simulink model "ABB_1010"  (R2024a)
(part 15 of 16)

et89 = Iyy6*dQ1*dQ5*t2*t4*t7*t35*t36*4.0+Iyy6*dQ1*dQ6*t4*t5*t9*t32*t33*4.0+Iyy6*dQ1*dQ2*t4*t5*t10*t33*t36*4.0+Iyy6*dQ1*dQ3*t4*t5*t10*t32*t36*4.0+Iyy6*dQ1*dQ3*t4*t5*t10*t33*t36*4.0+Iyy6*dQ1*dQ4*t5*t6*t11*t32*t33*4.0+Iyy6*dQ1*dQ5*t3*t4*t8*t35*t36*4.0+Iyy6*dQ2*dQ5*t2*t3*t9*t35*t36*2.0+Iyy6*dQ1*dQ4*t5*t6*t11*t32*t34*4.0+Iyy6*dQ1*dQ6*t4*t5*t9*t32*t36*4.0+Iyy6*dQ2*dQ6*t2*t5*t8*t34*t36*4.0+Iyy6*dQ2*dQ6*t3*t5*t7*t34*t36*4.0+Iyy6*dQ3*dQ5*t2*t3*t9*t35*t36*2.0+Iyy6*dQ1*dQ4*t5*t6*t11*t33*t34*4.0+Iyy6*dQ1*dQ6*t4*t5*t9*t33*t36*4.0+Iyy6*dQ3*dQ6*t2*t5*t8*t34*t36*4.0+Iyy6*dQ3*dQ6*t3*t5*t7*t34*t36*4.0-Iyy6*dQ4*dQ5*t2*t4*t8*t35*t36*2.0-Iyy6*dQ4*dQ5*t3*t4*t7*t35*t36*2.0;
et90 = Iyy6*dQ2*dQ5*t7*t8*t9*t35*t36*-2.0-Iyy6*dQ3*dQ5*t7*t8*t9*t35*t36*2.0+Iyy6*dQ1*dQ2*t2*t7*t33*t34*t35*4.0-Iyy6*dQ1*dQ2*t2*t7*t33*t34*t36*4.0+Iyy6*dQ1*dQ2*t3*t8*t32*t34*t35*4.0+Iyy6*dQ1*dQ3*t2*t7*t33*t34*t35*4.0-Iyy6*dQ1*dQ2*t2*t7*t33*t35*t36*4.0-Iyy6*dQ1*dQ2*t3*t8*t32*t34*t36*4.0-Iyy6*dQ1*dQ3*t2*t7*t33*t34*t36*4.0+Iyy6*dQ1*dQ3*t3*t8*t32*t34*t35*4.0+Iyy6*dQ1*dQ2*t2*t7*t34*t35*t36*2.0-Iyy6*dQ1*dQ2*t3*t8*t32*t35*t36*4.0-Iyy6*dQ1*dQ3*t2*t7*t33*t35*t36*4.0-Iyy6*dQ1*dQ3*t3*t8*t32*t34*t36*4.0+Iyy6*dQ1*dQ3*t2*t7*t34*t35*t36*2.0-Iyy6*dQ1*dQ3*t3*t8*t32*t35*t36*4.0+Iyy6*dQ1*dQ4*t4*t9*t32*t33*t35*4.0+Iyy6*dQ1*dQ2*t3*t8*t34*t35*t36*2.0;
et91 = Iyy6*dQ1*dQ4*t4*t9*t32*t33*t36*-4.0+Iyy6*dQ1*dQ3*t3*t8*t34*t35*t36*2.0+Iyy6*dQ1*dQ5*t5*t10*t32*t33*t34*4.0+Iyy6*dQ1*dQ4*t4*t9*t32*t35*t36*2.0+Iyy6*dQ2*dQ4*t2*t8*t34*t35*t36*2.0+Iyy6*dQ2*dQ4*t3*t7*t34*t35*t36*2.0+Iyy6*dQ1*dQ4*t4*t9*t33*t35*t36*2.0-Iyy6*dQ1*dQ5*t5*t10*t32*t33*t36*4.0+Iyy6*dQ3*dQ4*t2*t8*t34*t35*t36*2.0+Iyy6*dQ3*dQ4*t3*t7*t34*t35*t36*2.0+Iyy6*dQ1*dQ5*t5*t10*t32*t34*t36*2.0-Iyy6*dQ1*dQ6*t6*t11*t32*t33*t34*4.0+Iyy6*dQ1*dQ5*t5*t10*t33*t34*t36*2.0-Iyy6*dQ1*dQ6*t6*t11*t32*t33*t35*4.0+Iyy6*dQ1*dQ6*t6*t11*t32*t34*t35*2.0+Iyy6*dQ1*dQ6*t6*t11*t33*t34*t35*2.0-Izz5*dQ1*dQ4*t2*t5*t7*t9*t10*2.0-Izz5*dQ2*dQ3*t2*t5*t8*t9*t10*2.0-Izz5*dQ2*dQ3*t3*t5*t7*t9*t10*2.0;
et92 = Izz6*dQ1*dQ4*t2*t5*t7*t9*t10*-2.0-Izz5*dQ1*dQ4*t3*t5*t8*t9*t10*2.0-Izz6*dQ2*dQ3*t2*t5*t8*t9*t10*2.0-Izz6*dQ2*dQ3*t3*t5*t7*t9*t10*2.0-Izz6*dQ1*dQ4*t3*t5*t8*t9*t10*2.0+Izz5*dQ2*dQ3*t2*t3*t4*t9*t35*2.0+Izz6*dQ2*dQ3*t2*t3*t4*t9*t35*2.0-Izz5*dQ2*dQ3*t4*t7*t8*t9*t35*2.0-Izz6*dQ2*dQ3*t4*t7*t8*t9*t35*2.0-Izz5*dQ1*dQ2*t4*t5*t10*t32*t33*8.0-Izz5*dQ1*dQ5*t2*t4*t7*t33*t35*8.0-Izz5*dQ1*dQ3*t4*t5*t10*t32*t33*8.0-Izz5*dQ1*dQ5*t3*t4*t8*t32*t35*8.0-Izz6*dQ1*dQ2*t4*t5*t10*t32*t33*8.0-Izz6*dQ1*dQ5*t2*t4*t7*t33*t35*8.0-Izz6*dQ1*dQ3*t4*t5*t10*t32*t33*8.0-Izz6*dQ1*dQ5*t3*t4*t8*t32*t35*8.0;
et93 = Izz5*dQ1*dQ2*t2*t7*t33*t34*t35*-4.0-Izz5*dQ1*dQ2*t3*t8*t32*t34*t35*4.0-Izz5*dQ1*dQ3*t2*t7*t33*t34*t35*4.0-Izz6*dQ1*dQ2*t2*t7*t33*t34*t35*4.0-Izz5*dQ1*dQ3*t3*t8*t32*t34*t35*4.0-Izz6*dQ1*dQ2*t3*t8*t32*t34*t35*4.0-Izz6*dQ1*dQ3*t2*t7*t33*t34*t35*4.0-Izz6*dQ1*dQ3*t3*t8*t32*t34*t35*4.0-Izz5*dQ1*dQ4*t4*t9*t32*t33*t35*4.0-Izz6*dQ1*dQ4*t4*t9*t32*t33*t35*4.0-Izz5*dQ1*dQ5*t5*t10*t32*t33*t34*4.0-Izz6*dQ1*dQ5*t5*t10*t32*t33*t34*4.0+dQ2*dQ3*m4*t2*t3*t4*t9*t14*2.0+dQ2*dQ3*m5*t2*t3*t4*t9*t14*2.0+dQ2*dQ3*m4*t2*t3*t4*t9*t16*2.0+dQ2*dQ3*m6*t2*t3*t4*t9*t14*2.0-dQ2*dQ3*m4*t2*t3*t4*t9*t19*2.0-dQ2*dQ3*m6*t2*t3*t4*t9*t18*2.0;
et94 = dQ2*dQ3*m5*t2*t3*t4*t9*t20*-2.0-dQ2*dQ3*m4*t4*t7*t8*t9*t14*2.0+dQ2*dQ3*m6*t2*t3*t4*t9*t22*2.0-dQ2*dQ6*m6*t2*t3*t4*t10*t18*2.0-dQ4*dQ5*m5*t2*t3*t5*t10*t17*2.0-dQ2*dQ3*m5*t4*t7*t8*t9*t14*2.0-dQ3*dQ6*m6*t2*t3*t4*t10*t18*2.0-dQ2*dQ3*m4*t4*t7*t8*t9*t16*2.0+dQ2*dQ3*m5*t2*t3*t4*t9*t25*2.0-dQ2*dQ3*m6*t4*t7*t8*t9*t14*2.0-dQ5*dQ6*m6*t2*t4*t5*t8*t18*2.0-dQ5*dQ6*m6*t3*t4*t5*t7*t18*2.0+dQ2*dQ3*m6*t2*t3*t4*t9*t26*2.0+dQ2*dQ3*m4*t4*t7*t8*t9*t19*2.0-dQ4*dQ5*m6*t2*t3*t5*t10*t21*2.0+dQ4*dQ6*m6*t2*t3*t6*t11*t18*2.0+dQ2*dQ3*m6*t4*t7*t8*t9*t18*2.0+dQ4*dQ5*m6*t2*t3*t5*t10*t22*2.0;
et95 = dQ2*dQ3*m5*t4*t7*t8*t9*t20*2.0+dQ1*dQ6*m6*t2*t7*t9*t10*t18*2.0+dQ4*dQ5*m5*t2*t3*t5*t10*t25*2.0-dQ4*dQ6*m6*t2*t3*t6*t11*t21*2.0+dQ1*dQ6*m6*t3*t8*t9*t10*t18*2.0-dQ2*dQ3*m6*t4*t7*t8*t9*t22*2.0+dQ2*dQ6*m6*t4*t7*t8*t10*t18*2.0+dQ4*dQ5*m5*t5*t7*t8*t10*t17*2.0+dQ4*dQ5*m6*t2*t3*t5*t10*t26*2.0-dQ1*dQ6*m6*t2*t7*t9*t10*t21*2.0+dQ3*dQ6*m6*t4*t7*t8*t10*t18*2.0+dQ1*dQ2*m6*t6*t9*t10*t11*t18*2.0-dQ2*dQ3*m5*t4*t7*t8*t9*t25*2.0+dQ1*dQ3*m6*t6*t9*t10*t11*t18*2.0-dQ1*dQ6*m6*t3*t8*t9*t10*t21*2.0-dQ2*dQ3*m6*t4*t7*t8*t9*t26*2.0-dQ1*dQ2*m6*t6*t9*t10*t11*t21*2.0+dQ4*dQ5*m6*t5*t7*t8*t10*t21*2.0+dQ4*dQ6*m6*t2*t8*t9*t10*t21*2.0;
et96 = dQ4*dQ6*m6*t3*t7*t9*t10*t21*2.0-dQ4*dQ6*m6*t6*t7*t8*t11*t18*2.0-dQ1*dQ3*m6*t6*t9*t10*t11*t21*2.0-dQ4*dQ5*m6*t5*t7*t8*t10*t22*2.0-dQ4*dQ5*m5*t5*t7*t8*t10*t25*2.0+dQ4*dQ6*m6*t6*t7*t8*t11*t21*2.0-dQ4*dQ5*m6*t5*t7*t8*t10*t26*2.0+dQ1*dQ5*m5*t2*t4*t7*t17*t33*4.0+dQ1*dQ5*m5*t3*t4*t8*t17*t32*4.0+dQ1*dQ2*m5*t4*t5*t10*t17*t32*4.0+dQ1*dQ5*m5*t2*t4*t7*t17*t35*4.0+dQ1*dQ2*m5*t4*t5*t10*t17*t33*4.0+dQ1*dQ3*m5*t4*t5*t10*t17*t32*4.0+dQ1*dQ3*m5*t4*t5*t10*t17*t33*4.0+dQ1*dQ5*m5*t3*t4*t8*t17*t35*4.0+dQ2*dQ5*m5*t2*t3*t9*t17*t35*2.0-dQ1*dQ5*m6*t2*t4*t7*t18*t36*2.0+dQ1*dQ5*m6*t2*t4*t7*t21*t33*4.0+dQ3*dQ5*m5*t2*t3*t9*t17*t35*2.0;
et97 = dQ1*dQ5*m6*t2*t4*t7*t22*t33*-4.0+dQ1*dQ5*m6*t3*t4*t8*t21*t32*4.0-dQ4*dQ5*m5*t2*t4*t8*t17*t35*2.0-dQ4*dQ5*m5*t3*t4*t7*t17*t35*2.0+dQ1*dQ2*m6*t4*t5*t10*t21*t32*4.0+dQ1*dQ5*m6*t2*t4*t7*t21*t35*4.0-dQ1*dQ5*m6*t3*t4*t8*t18*t36*2.0-dQ1*dQ5*m6*t3*t4*t8*t22*t32*4.0-dQ1*dQ6*m6*t4*t5*t9*t18*t32*2.0-dQ2*dQ6*m6*t2*t5*t8*t18*t34*2.0-dQ2*dQ6*m6*t3*t5*t7*t18*t34*2.0-dQ1*dQ2*m6*t4*t5*t10*t18*t36*2.0+dQ1*dQ2*m6*t4*t5*t10*t21*t33*4.0-dQ1*dQ2*m6*t4*t5*t10*t22*t32*4.0+dQ1*dQ3*m6*t4*t5*t10*t21*t32*4.0-dQ1*dQ5*m5*t2*t4*t7*t25*t33*4.0+dQ1*dQ5*m6*t2*t4*t7*t21*t36*2.0-dQ1*dQ5*m6*t2*t4*t7*t22*t35*4.0;
et98 = dQ1*dQ6*m6*t4*t5*t9*t18*t33*-2.0-dQ3*dQ6*m6*t2*t5*t8*t18*t34*2.0-dQ3*dQ6*m6*t3*t5*t7*t18*t34*2.0-dQ1*dQ2*m6*t4*t5*t10*t22*t33*4.0-dQ1*dQ3*m6*t4*t5*t10*t18*t36*2.0+dQ1*dQ3*m6*t4*t5*t10*t21*t33*4.0-dQ1*dQ3*m6*t4*t5*t10*t22*t32*4.0-dQ1*dQ4*m6*t5*t6*t11*t18*t32*2.0-dQ1*dQ5*m5*t3*t4*t8*t25*t32*4.0+dQ1*dQ5*m6*t3*t4*t8*t21*t35*4.0+dQ2*dQ5*m6*t2*t3*t9*t21*t35*2.0-dQ2*dQ6*m6*t2*t5*t8*t18*t36*2.0-dQ2*dQ6*m6*t3*t5*t7*t18*t36*2.0+dQ4*dQ5*m6*t2*t4*t8*t18*t36*2.0+dQ4*dQ5*m6*t3*t4*t7*t18*t36*2.0-dQ1*dQ2*m5*t4*t5*t10*t25*t32*4.0-dQ1*dQ3*m6*t4*t5*t10*t22*t33*4.0-dQ1*dQ4*m6*t5*t6*t11*t18*t33*2.0;
et99 = dQ1*dQ5*m5*t2*t4*t7*t25*t35*-4.0-dQ1*dQ5*m6*t2*t4*t7*t26*t33*4.0+dQ1*dQ5*m6*t3*t4*t8*t21*t36*2.0-dQ1*dQ5*m6*t3*t4*t8*t22*t35*4.0+dQ1*dQ6*m6*t4*t5*t9*t21*t32*2.0-dQ2*dQ5*m6*t2*t3*t9*t22*t35*2.0+dQ2*dQ6*m6*t2*t5*t8*t21*t34*2.0+dQ2*dQ6*m6*t3*t5*t7*t21*t34*2.0+dQ3*dQ5*m6*t2*t3*t9*t21*t35*2.0-dQ3*dQ6*m6*t2*t5*t8*t18*t36*2.0-dQ3*dQ6*m6*t3*t5*t7*t18*t36*2.0-dQ1*dQ2*m5*t4*t5*t10*t25*t33*4.0+dQ1*dQ2*m6*t4*t5*t10*t21*t36*2.0-dQ1*dQ3*m5*t4*t5*t10*t25*t32*4.0-dQ1*dQ5*m6*t3*t4*t8*t26*t32*4.0+dQ1*dQ6*m6*t4*t5*t9*t21*t33*2.0-dQ3*dQ5*m6*t2*t3*t9*t22*t35*2.0+dQ3*dQ6*m6*t2*t5*t8*t21*t34*2.0+dQ3*dQ6*m6*t3*t5*t7*t21*t34*2.0;
et100 = dQ4*dQ5*m6*t2*t4*t8*t21*t35*-2.0-dQ4*dQ5*m6*t3*t4*t7*t21*t35*2.0-dQ1*dQ2*m6*t4*t5*t10*t26*t32*4.0-dQ1*dQ3*m5*t4*t5*t10*t25*t33*4.0+dQ1*dQ3*m6*t4*t5*t10*t21*t36*2.0+dQ1*dQ4*m6*t5*t6*t11*t21*t32*2.0-dQ1*dQ5*m5*t3*t4*t8*t25*t35*4.0-dQ1*dQ5*m6*t2*t4*t7*t26*t35*4.0-dQ2*dQ5*m5*t2*t3*t9*t25*t35*2.0+dQ2*dQ6*m6*t2*t5*t8*t21*t36*2.0+dQ2*dQ6*m6*t3*t5*t7*t21*t36*2.0-dQ4*dQ5*m6*t2*t4*t8*t21*t36*2.0+dQ4*dQ5*m6*t2*t4*t8*t22*t35*2.0-dQ4*dQ5*m6*t3*t4*t7*t21*t36*2.0+dQ4*dQ5*m6*t3*t4*t7*t22*t35*2.0+dQ5*dQ6*m6*t2*t3*t10*t18*t36*2.0-dQ1*dQ2*m6*t4*t5*t10*t26*t33*4.0-dQ1*dQ3*m6*t4*t5*t10*t26*t32*4.0;
et101 = dQ1*dQ4*m6*t5*t6*t11*t21*t33*2.0-dQ3*dQ5*m5*t2*t3*t9*t25*t35*2.0+dQ3*dQ6*m6*t2*t5*t8*t21*t36*2.0+dQ3*dQ6*m6*t3*t5*t7*t21*t36*2.0-dQ1*dQ3*m6*t4*t5*t10*t26*t33*4.0-dQ1*dQ5*m6*t3*t4*t8*t26*t35*4.0-dQ2*dQ5*m5*t7*t8*t9*t17*t35*2.0-dQ2*dQ5*m6*t2*t3*t9*t26*t35*2.0+dQ4*dQ5*m5*t2*t4*t8*t25*t35*2.0+dQ4*dQ5*m5*t3*t4*t7*t25*t35*2.0-dQ3*dQ5*m5*t7*t8*t9*t17*t35*2.0-dQ3*dQ5*m6*t2*t3*t9*t26*t35*2.0-dQ5*dQ6*m6*t2*t3*t10*t21*t36*2.0+dQ4*dQ5*m6*t2*t4*t8*t26*t35*2.0+dQ4*dQ5*m6*t3*t4*t7*t26*t35*2.0-dQ2*dQ5*m6*t7*t8*t9*t21*t35*2.0+dQ2*dQ5*m6*t7*t8*t9*t22*t35*2.0-dQ3*dQ5*m6*t7*t8*t9*t21*t35*2.0+dQ3*dQ5*m6*t7*t8*t9*t22*t35*2.0;
et102 = dQ2*dQ5*m5*t7*t8*t9*t25*t35*2.0-dQ5*dQ6*m6*t7*t8*t10*t18*t36*2.0-dQ1*dQ2*m4*t2*t7*t14*t33*t34*4.0+dQ3*dQ5*m5*t7*t8*t9*t25*t35*2.0-dQ1*dQ2*m4*t3*t8*t14*t32*t34*4.0-dQ1*dQ2*m5*t2*t7*t14*t33*t34*4.0-dQ1*dQ3*m4*t2*t7*t14*t33*t34*4.0+dQ2*dQ5*m6*t7*t8*t9*t26*t35*2.0-dQ1*dQ2*m4*t2*t7*t16*t33*t34*4.0-dQ1*dQ2*m5*t3*t8*t14*t32*t34*4.0-dQ1*dQ2*m6*t2*t7*t14*t33*t34*4.0-dQ1*dQ3*m4*t3*t8*t14*t32*t34*4.0-dQ1*dQ3*m5*t2*t7*t14*t33*t34*4.0+dQ3*dQ5*m6*t7*t8*t9*t26*t35*2.0+dQ5*dQ6*m6*t7*t8*t10*t21*t36*2.0-dQ1*dQ2*m4*t3*t8*t16*t32*t34*4.0-dQ1*dQ2*m6*t3*t8*t14*t32*t34*4.0-dQ1*dQ3*m4*t2*t7*t16*t33*t34*4.0;
et103 = dQ1*dQ3*m5*t3*t8*t14*t32*t34*-4.0-dQ1*dQ3*m6*t2*t7*t14*t33*t34*4.0-dQ1*dQ3*m4*t3*t8*t16*t32*t34*4.0-dQ1*dQ3*m6*t3*t8*t14*t32*t34*4.0-dQ1*dQ4*m4*t4*t9*t14*t32*t33*4.0+dQ1*dQ2*m4*t2*t7*t19*t33*t34*4.0-dQ1*dQ2*m5*t2*t7*t17*t33*t35*4.0-dQ1*dQ4*m5*t4*t9*t14*t32*t33*4.0+dQ1*dQ2*m4*t3*t8*t19*t32*t34*4.0+dQ1*dQ2*m5*t2*t7*t17*t34*t35*2.0-dQ1*dQ2*m5*t3*t8*t17*t32*t35*4.0+dQ1*dQ2*m6*t2*t7*t18*t33*t34*4.0+dQ1*dQ3*m4*t2*t7*t19*t33*t34*4.0-dQ1*dQ3*m5*t2*t7*t17*t33*t35*4.0-dQ1*dQ4*m4*t4*t9*t16*t32*t33*4.0-dQ1*dQ4*m6*t4*t9*t14*t32*t33*4.0+dQ1*dQ2*m5*t2*t7*t20*t33*t34*4.0+dQ1*dQ2*m6*t3*t8*t18*t32*t34*4.0;
et104 = dQ1*dQ3*m4*t3*t8*t19*t32*t34*4.0+dQ1*dQ3*m5*t2*t7*t17*t34*t35*2.0-dQ1*dQ3*m5*t3*t8*t17*t32*t35*4.0+dQ1*dQ3*m6*t2*t7*t18*t33*t34*4.0+dQ1*dQ2*m5*t3*t8*t17*t34*t35*2.0+dQ1*dQ2*m5*t3*t8*t20*t32*t34*4.0+dQ1*dQ2*m6*t2*t7*t18*t33*t36*8.0+dQ1*dQ3*m5*t2*t7*t20*t33*t34*4.0+dQ1*dQ3*m6*t3*t8*t18*t32*t34*4.0+dQ1*dQ2*m6*t2*t7*t18*t34*t36*2.0+dQ1*dQ2*m6*t3*t8*t18*t32*t36*8.0+dQ1*dQ3*m5*t3*t8*t17*t34*t35*2.0+dQ1*dQ3*m5*t3*t8*t20*t32*t34*4.0+dQ1*dQ3*m6*t2*t7*t18*t33*t36*8.0+dQ1*dQ4*m4*t4*t9*t19*t32*t33*4.0+dQ1*dQ2*m6*t2*t7*t18*t35*t36*2.0-dQ1*dQ2*m6*t2*t7*t21*t33*t35*4.0-dQ1*dQ2*m6*t2*t7*t22*t33*t34*4.0+dQ1*dQ3*m6*t2*t7*t18*t34*t36*2.0;
et105 = dQ1*dQ3*m6*t3*t8*t18*t32*t36*8.0+dQ1*dQ4*m5*t4*t9*t17*t32*t35*2.0+dQ1*dQ4*m6*t4*t9*t18*t32*t33*4.0+dQ2*dQ4*m5*t2*t8*t17*t34*t35*2.0+dQ2*dQ4*m5*t3*t7*t17*t34*t35*2.0-dQ1*dQ2*m6*t2*t7*t21*t33*t36*8.0+dQ1*dQ2*m6*t2*t7*t21*t34*t35*2.0+dQ1*dQ2*m6*t2*t7*t22*t33*t35*4.0+dQ1*dQ2*m6*t3*t8*t18*t34*t36*2.0-dQ1*dQ2*m6*t3*t8*t21*t32*t35*4.0-dQ1*dQ2*m6*t3*t8*t22*t32*t34*4.0+dQ1*dQ3*m6*t2*t7*t18*t35*t36*2.0-dQ1*dQ3*m6*t2*t7*t21*t33*t35*4.0-dQ1*dQ3*m6*t2*t7*t22*t33*t34*4.0+dQ1*dQ4*m5*t4*t9*t17*t33*t35*2.0+dQ1*dQ4*m5*t4*t9*t20*t32*t33*4.0-dQ1*dQ5*m5*t5*t10*t17*t32*t33*4.0+dQ3*dQ4*m5*t2*t8*t17*t34*t35*2.0+dQ3*dQ4*m5*t3*t7*t17*t34*t35*2.0;
et106 = dQ1*dQ2*m5*t2*t7*t25*t33*t34*-4.0-dQ1*dQ2*m6*t2*t7*t21*t34*t36*2.0-dQ1*dQ2*m6*t2*t7*t22*t34*t35*2.0+dQ1*dQ2*m6*t3*t8*t18*t35*t36*2.0-dQ1*dQ2*m6*t3*t8*t21*t32*t36*8.0+dQ1*dQ2*m6*t3*t8*t22*t32*t35*4.0-dQ1*dQ3*m6*t2*t7*t21*t33*t36*8.0+dQ1*dQ3*m6*t2*t7*t21*t34*t35*2.0+dQ1*dQ3*m6*t2*t7*t22*t33*t35*4.0+dQ1*dQ3*m6*t3*t8*t18*t34*t36*2.0-dQ1*dQ3*m6*t3*t8*t21*t32*t35*4.0-dQ1*dQ3*m6*t3*t8*t22*t32*t34*4.0+dQ1*dQ5*m5*t5*t10*t17*t32*t34*2.0+dQ1*dQ2*m5*t2*t7*t25*t33*t35*4.0-dQ1*dQ2*m5*t3*t8*t25*t32*t34*4.0-dQ1*dQ2*m6*t2*t7*t21*t35*t36*2.0+dQ1*dQ2*m6*t3*t8*t21*t34*t35*2.0-dQ1*dQ3*m5*t2*t7*t25*t33*t34*4.0;
et107 = dQ1*dQ3*m6*t2*t7*t21*t34*t36*-2.0-dQ1*dQ3*m6*t2*t7*t22*t34*t35*2.0+dQ1*dQ3*m6*t3*t8*t18*t35*t36*2.0-dQ1*dQ3*m6*t3*t8*t21*t32*t36*8.0+dQ1*dQ3*m6*t3*t8*t22*t32*t35*4.0+dQ1*dQ4*m6*t4*t9*t18*t32*t36*2.0+dQ1*dQ5*m5*t5*t10*t17*t33*t34*2.0+dQ2*dQ4*m6*t2*t8*t18*t34*t36*2.0+dQ2*dQ4*m6*t3*t7*t18*t34*t36*2.0-dQ1*dQ2*m5*t2*t7*t25*t34*t35*2.0+dQ1*dQ2*m5*t3*t8*t25*t32*t35*4.0-dQ1*dQ2*m6*t2*t7*t26*t33*t34*4.0-dQ1*dQ2*m6*t3*t8*t21*t34*t36*2.0-dQ1*dQ2*m6*t3*t8*t22*t34*t35*2.0+dQ1*dQ3*m5*t2*t7*t25*t33*t35*4.0-dQ1*dQ3*m5*t3*t8*t25*t32*t34*4.0-dQ1*dQ3*m6*t2*t7*t21*t35*t36*2.0+dQ1*dQ3*m6*t3*t8*t21*t34*t35*2.0+dQ1*dQ4*m6*t4*t9*t18*t33*t36*2.0;
et108 = dQ1*dQ4*m6*t4*t9*t22*t32*t33*-4.0-dQ2*dQ4*m6*t2*t8*t18*t35*t36*2.0-dQ2*dQ4*m6*t3*t7*t18*t35*t36*2.0+dQ3*dQ4*m6*t2*t8*t18*t34*t36*2.0+dQ3*dQ4*m6*t3*t7*t18*t34*t36*2.0+dQ1*dQ2*m6*t2*t7*t26*t33*t35*4.0-dQ1*dQ2*m6*t3*t8*t21*t35*t36*2.0-dQ1*dQ2*m6*t3*t8*t26*t32*t34*4.0-dQ1*dQ3*m5*t2*t7*t25*t34*t35*2.0+dQ1*dQ3*m5*t3*t8*t25*t32*t35*4.0-dQ1*dQ3*m6*t2*t7*t26*t33*t34*4.0-dQ1*dQ3*m6*t3*t8*t21*t34*t36*2.0-dQ1*dQ3*m6*t3*t8*t22*t34*t35*2.0+dQ1*dQ4*m6*t4*t9*t21*t32*t35*2.0+dQ2*dQ4*m6*t2*t8*t21*t34*t35*2.0+dQ2*dQ4*m6*t3*t7*t21*t34*t35*2.0-dQ3*dQ4*m6*t2*t8*t18*t35*t36*2.0-dQ3*dQ4*m6*t3*t7*t18*t35*t36*2.0;
et109 = dQ1*dQ2*m5*t3*t8*t25*t34*t35*-2.0-dQ1*dQ2*m6*t2*t7*t26*t34*t35*2.0+dQ1*dQ2*m6*t3*t8*t26*t32*t35*4.0+dQ1*dQ3*m6*t2*t7*t26*t33*t35*4.0-dQ1*dQ3*m6*t3*t8*t21*t35*t36*2.0-dQ1*dQ3*m6*t3*t8*t26*t32*t34*4.0-dQ1*dQ4*m5*t4*t9*t25*t32*t33*4.0-dQ1*dQ4*m6*t4*t9*t21*t32*t36*2.0+dQ1*dQ4*m6*t4*t9*t21*t33*t35*2.0-dQ1*dQ4*m6*t4*t9*t22*t32*t35*2.0+dQ1*dQ5*m6*t5*t10*t18*t32*t36*2.0-dQ1*dQ5*m6*t5*t10*t21*t32*t33*4.0+dQ1*dQ6*m6*t6*t11*t18*t32*t33*8.0-dQ2*dQ4*m6*t2*t8*t21*t34*t36*2.0-dQ2*dQ4*m6*t2*t8*t22*t34*t35*2.0-dQ2*dQ4*m6*t3*t7*t21*t34*t36*2.0-dQ2*dQ4*m6*t3*t7*t22*t34*t35*2.0+dQ3*dQ4*m6*t2*t8*t21*t34*t35*2.0;
et110 = dQ3*dQ4*m6*t3*t7*t21*t34*t35*2.0-dQ1*dQ3*m5*t3*t8*t25*t34*t35*2.0-dQ1*dQ3*m6*t2*t7*t26*t34*t35*2.0+dQ1*dQ3*m6*t3*t8*t26*t32*t35*4.0-dQ1*dQ4*m6*t4*t9*t21*t33*t36*2.0-dQ1*dQ4*m6*t4*t9*t22*t33*t35*2.0+dQ1*dQ5*m6*t5*t10*t18*t33*t36*2.0+dQ1*dQ5*m6*t5*t10*t21*t32*t34*2.0+dQ1*dQ5*m6*t5*t10*t22*t32*t33*4.0+dQ1*dQ6*m6*t6*t11*t18*t32*t34*2.0+dQ2*dQ4*m6*t2*t8*t21*t35*t36*2.0+dQ2*dQ4*m6*t3*t7*t21*t35*t36*2.0-dQ3*dQ4*m6*t2*t8*t21*t34*t36*2.0-dQ3*dQ4*m6*t2*t8*t22*t34*t35*2.0-dQ3*dQ4*m6*t3*t7*t21*t34*t36*2.0-dQ3*dQ4*m6*t3*t7*t22*t34*t35*2.0-dQ1*dQ2*m6*t3*t8*t26*t34*t35*2.0-dQ1*dQ4*m5*t4*t9*t25*t32*t35*2.0;
et111 = dQ1*dQ4*m6*t4*t9*t26*t32*t33*-4.0+dQ1*dQ5*m6*t5*t10*t21*t33*t34*2.0-dQ1*dQ5*m6*t5*t10*t22*t32*t34*2.0+dQ1*dQ6*m6*t6*t11*t18*t32*t35*2.0+dQ1*dQ6*m6*t6*t11*t18*t33*t34*2.0-dQ2*dQ4*m5*t2*t8*t25*t34*t35*2.0-dQ2*dQ4*m5*t3*t7*t25*t34*t35*2.0+dQ3*dQ4*m6*t2*t8*t21*t35*t36*2.0+dQ3*dQ4*m6*t3*t7*t21*t35*t36*2.0-dQ1*dQ3*m6*t3*t8*t26*t34*t35*2.0-dQ1*dQ4*m5*t4*t9*t25*t33*t35*2.0+dQ1*dQ5*m5*t5*t10*t25*t32*t33*4.0-dQ1*dQ5*m6*t5*t10*t21*t32*t36*2.0-dQ1*dQ5*m6*t5*t10*t22*t33*t34*2.0+dQ1*dQ6*m6*t6*t11*t18*t33*t35*2.0-dQ1*dQ6*m6*t6*t11*t21*t32*t33*8.0-dQ3*dQ4*m5*t2*t8*t25*t34*t35*2.0-dQ3*dQ4*m5*t3*t7*t25*t34*t35*2.0;
et112 = dQ1*dQ4*m6*t4*t9*t26*t32*t35*-2.0-dQ1*dQ5*m5*t5*t10*t25*t32*t34*2.0-dQ1*dQ5*m6*t5*t10*t21*t33*t36*2.0-dQ1*dQ6*m6*t6*t11*t21*t32*t34*2.0-dQ2*dQ4*m6*t2*t8*t26*t34*t35*2.0-dQ2*dQ4*m6*t3*t7*t26*t34*t35*2.0-dQ1*dQ4*m6*t4*t9*t26*t33*t35*2.0-dQ1*dQ5*m5*t5*t10*t25*t33*t34*2.0+dQ1*dQ5*m6*t5*t10*t26*t32*t33*4.0-dQ1*dQ6*m6*t6*t11*t21*t32*t35*2.0-dQ1*dQ6*m6*t6*t11*t21*t33*t34*2.0-dQ3*dQ4*m6*t2*t8*t26*t34*t35*2.0-dQ3*dQ4*m6*t3*t7*t26*t34*t35*2.0-dQ1*dQ5*m6*t5*t10*t26*t32*t34*2.0-dQ1*dQ6*m6*t6*t11*t21*t33*t35*2.0-dQ1*dQ5*m6*t5*t10*t26*t33*t34*2.0-Ixx6*dQ2*dQ5*t2*t3*t4*t5*t6*t11*2.0-Ixx6*dQ3*dQ5*t2*t3*t4*t5*t6*t11*2.0;
et113 = Ixx5*dQ1*dQ5*t2*t3*t5*t7*t8*t10*-4.0+Ixx5*dQ2*dQ5*t2*t4*t5*t8*t9*t10*2.0+Ixx5*dQ2*dQ5*t3*t4*t5*t7*t9*t10*2.0+Ixx6*dQ1*dQ6*t2*t3*t6*t7*t8*t11*8.0+Ixx5*dQ3*dQ5*t2*t4*t5*t8*t9*t10*2.0+Ixx5*dQ3*dQ5*t3*t4*t5*t7*t9*t10*2.0+Ixx6*dQ1*dQ4*t2*t4*t6*t7*t10*t11*2.0+Ixx6*dQ1*dQ5*t2*t5*t6*t7*t9*t11*2.0+Ixx6*dQ2*dQ3*t2*t4*t6*t8*t10*t11*2.0+Ixx6*dQ2*dQ3*t3*t4*t6*t7*t10*t11*2.0+Ixx6*dQ1*dQ4*t3*t4*t6*t8*t10*t11*2.0+Ixx6*dQ1*dQ5*t3*t5*t6*t8*t9*t11*2.0+Ixx6*dQ2*dQ5*t4*t5*t6*t7*t8*t11*2.0+Ixx6*dQ2*dQ6*t2*t4*t6*t8*t9*t11*2.0+Ixx6*dQ2*dQ6*t3*t4*t6*t7*t9*t11*2.0+Ixx6*dQ3*dQ5*t4*t5*t6*t7*t8*t11*2.0+Ixx6*dQ3*dQ6*t2*t4*t6*t8*t9*t11*2.0+Ixx6*dQ3*dQ6*t3*t4*t6*t7*t9*t11*2.0;
et114 = Ixx6*dQ2*dQ3*t2*t3*t5*t6*t11*t34*-4.0-Ixx5*dQ1*dQ4*t2*t5*t7*t9*t10*t33*4.0-Ixx5*dQ1*dQ4*t3*t5*t8*t9*t10*t32*4.0+Ixx6*dQ1*dQ4*t2*t5*t7*t9*t10*t36*2.0+Ixx6*dQ2*dQ3*t2*t5*t8*t9*t10*t36*2.0+Ixx6*dQ2*dQ3*t3*t5*t7*t9*t10*t36*2.0+Ixx6*dQ1*dQ4*t3*t5*t8*t9*t10*t36*2.0+Ixx6*dQ2*dQ3*t5*t6*t7*t8*t11*t34*4.0+Ixx6*dQ1*dQ5*t4*t6*t9*t10*t11*t32*2.0+Ixx6*dQ2*dQ5*t2*t6*t8*t10*t11*t34*2.0+Ixx6*dQ2*dQ5*t3*t6*t7*t10*t11*t34*2.0+Ixx6*dQ1*dQ5*t4*t6*t9*t10*t11*t33*2.0+Ixx6*dQ3*dQ5*t2*t6*t8*t10*t11*t34*2.0+Ixx6*dQ3*dQ5*t3*t6*t7*t10*t11*t34*2.0-Ixx6*dQ2*dQ3*t2*t3*t4*t9*t35*t36*2.0-Ixx6*dQ1*dQ2*t6*t9*t10*t11*t32*t33*8.0-Ixx6*dQ1*dQ6*t2*t7*t9*t10*t33*t36*8.0;
et115 = Ixx6*dQ2*dQ3*t4*t7*t8*t9*t35*t36*2.0-Ixx6*dQ1*dQ3*t6*t9*t10*t11*t32*t33*8.0-Ixx6*dQ1*dQ6*t3*t8*t9*t10*t32*t36*8.0+Ixx6*dQ1*dQ2*t4*t5*t10*t32*t33*t36*8.0+Ixx6*dQ1*dQ5*t2*t4*t7*t33*t35*t36*8.0+Ixx6*dQ1*dQ3*t4*t5*t10*t32*t33*t36*8.0+Ixx6*dQ1*dQ5*t3*t4*t8*t32*t35*t36*8.0+Ixx6*dQ1*dQ4*t5*t6*t11*t32*t33*t34*8.0+Ixx6*dQ1*dQ6*t4*t5*t9*t32*t33*t36*8.0+Ixx6*dQ1*dQ2*t2*t7*t33*t34*t35*t36*4.0+Ixx6*dQ1*dQ2*t3*t8*t32*t34*t35*t36*4.0+Ixx6*dQ1*dQ3*t2*t7*t33*t34*t35*t36*4.0+Ixx6*dQ1*dQ3*t3*t8*t32*t34*t35*t36*4.0+Ixx6*dQ1*dQ4*t4*t9*t32*t33*t35*t36*4.0+Ixx6*dQ1*dQ5*t5*t10*t32*t33*t34*t36*4.0+Ixx6*dQ1*dQ6*t6*t11*t32*t33*t34*t35*4.0+Iyy6*dQ2*dQ5*t2*t3*t4*t5*t6*t11*2.0;
et116 = Iyy6*dQ3*dQ5*t2*t3*t4*t5*t6*t11*2.0-Iyy6*dQ1*dQ5*t2*t3*t5*t7*t8*t10*4.0-Iyy6*dQ1*dQ6*t2*t3*t6*t7*t8*t11*8.0-Iyy6*dQ1*dQ4*t2*t4*t6*t7*t10*t11*2.0+Iyy6*dQ2*dQ5*t2*t4*t5*t8*t9*t10*2.0+Iyy6*dQ2*dQ5*t3*t4*t5*t7*t9*t10*2.0-Iyy6*dQ1*dQ5*t2*t5*t6*t7*t9*t11*2.0-Iyy6*dQ2*dQ3*t2*t4*t6*t8*t10*t11*2.0-Iyy6*dQ2*dQ3*t3*t4*t6*t7*t10*t11*2.0+Iyy6*dQ3*dQ5*t2*t4*t5*t8*t9*t10*2.0+Iyy6*dQ3*dQ5*t3*t4*t5*t7*t9*t10*2.0-Iyy6*dQ1*dQ4*t3*t4*t6*t8*t10*t11*2.0-Iyy6*dQ1*dQ5*t3*t5*t6*t8*t9*t11*2.0-Iyy6*dQ2*dQ5*t4*t5*t6*t7*t8*t11*2.0-Iyy6*dQ2*dQ6*t2*t4*t6*t8*t9*t11*2.0-Iyy6*dQ2*dQ6*t3*t4*t6*t7*t9*t11*2.0-Iyy6*dQ3*dQ5*t4*t5*t6*t7*t8*t11*2.0;
et117 = Iyy6*dQ3*dQ6*t2*t4*t6*t8*t9*t11*-2.0-Iyy6*dQ3*dQ6*t3*t4*t6*t7*t9*t11*2.0+Iyy6*dQ2*dQ3*t2*t3*t5*t6*t11*t34*4.0-Iyy6*dQ1*dQ4*t2*t5*t7*t9*t10*t33*4.0-Iyy6*dQ1*dQ4*t3*t5*t8*t9*t10*t32*4.0-Iyy6*dQ1*dQ4*t2*t5*t7*t9*t10*t36*2.0-Iyy6*dQ2*dQ3*t2*t5*t8*t9*t10*t36*2.0-Iyy6*dQ2*dQ3*t3*t5*t7*t9*t10*t36*2.0-Iyy6*dQ1*dQ4*t3*t5*t8*t9*t10*t36*2.0-Iyy6*dQ2*dQ3*t5*t6*t7*t8*t11*t34*4.0-Iyy6*dQ1*dQ5*t4*t6*t9*t10*t11*t32*2.0-Iyy6*dQ2*dQ5*t2*t6*t8*t10*t11*t34*2.0-Iyy6*dQ2*dQ5*t3*t6*t7*t10*t11*t34*2.0-Iyy6*dQ1*dQ5*t4*t6*t9*t10*t11*t33*2.0-Iyy6*dQ3*dQ5*t2*t6*t8*t10*t11*t34*2.0-Iyy6*dQ3*dQ5*t3*t6*t7*t10*t11*t34*2.0;
et118 = Iyy6*dQ2*dQ3*t2*t3*t4*t9*t35*t36*2.0+Iyy6*dQ1*dQ2*t6*t9*t10*t11*t32*t33*8.0+Iyy6*dQ1*dQ6*t2*t7*t9*t10*t33*t36*8.0-Iyy6*dQ2*dQ3*t4*t7*t8*t9*t35*t36*2.0+Iyy6*dQ1*dQ3*t6*t9*t10*t11*t32*t33*8.0+Iyy6*dQ1*dQ6*t3*t8*t9*t10*t32*t36*8.0-Iyy6*dQ1*dQ2*t4*t5*t10*t32*t33*t36*8.0-Iyy6*dQ1*dQ5*t2*t4*t7*t33*t35*t36*8.0-Iyy6*dQ1*dQ3*t4*t5*t10*t32*t33*t36*8.0-Iyy6*dQ1*dQ5*t3*t4*t8*t32*t35*t36*8.0-Iyy6*dQ1*dQ4*t5*t6*t11*t32*t33*t34*8.0-Iyy6*dQ1*dQ6*t4*t5*t9*t32*t33*t36*8.0-Iyy6*dQ1*dQ2*t2*t7*t33*t34*t35*t36*4.0-Iyy6*dQ1*dQ2*t3*t8*t32*t34*t35*t36*4.0-Iyy6*dQ1*dQ3*t2*t7*t33*t34*t35*t36*4.0-Iyy6*dQ1*dQ3*t3*t8*t32*t34*t35*t36*4.0;
et119 = Iyy6*dQ1*dQ4*t4*t9*t32*t33*t35*t36*-4.0-Iyy6*dQ1*dQ5*t5*t10*t32*t33*t34*t36*4.0-Iyy6*dQ1*dQ6*t6*t11*t32*t33*t34*t35*4.0+Izz5*dQ1*dQ5*t2*t3*t5*t7*t8*t10*4.0+Izz6*dQ1*dQ5*t2*t3*t5*t7*t8*t10*4.0-Izz5*dQ2*dQ5*t2*t4*t5*t8*t9*t10*2.0-Izz5*dQ2*dQ5*t3*t4*t5*t7*t9*t10*2.0-Izz5*dQ3*dQ5*t2*t4*t5*t8*t9*t10*2.0-Izz5*dQ3*dQ5*t3*t4*t5*t7*t9*t10*2.0-Izz6*dQ2*dQ5*t2*t4*t5*t8*t9*t10*2.0-Izz6*dQ2*dQ5*t3*t4*t5*t7*t9*t10*2.0-Izz6*dQ3*dQ5*t2*t4*t5*t8*t9*t10*2.0-Izz6*dQ3*dQ5*t3*t4*t5*t7*t9*t10*2.0+Izz5*dQ1*dQ4*t2*t5*t7*t9*t10*t33*4.0+Izz5*dQ1*dQ4*t3*t5*t8*t9*t10*t32*4.0+Izz6*dQ1*dQ4*t2*t5*t7*t9*t10*t33*4.0+Izz6*dQ1*dQ4*t3*t5*t8*t9*t10*t32*4.0;
et120 = dQ2*dQ3*m6*t2*t3*t5*t6*t11*t18*-2.0+dQ2*dQ3*m6*t2*t3*t5*t6*t11*t21*2.0-dQ1*dQ4*m5*t2*t5*t7*t9*t10*t17*2.0-dQ2*dQ3*m5*t2*t5*t8*t9*t10*t17*2.0-dQ2*dQ3*m5*t3*t5*t7*t9*t10*t17*2.0-dQ1*dQ4*m5*t3*t5*t8*t9*t10*t17*2.0-dQ1*dQ4*m6*t2*t5*t7*t9*t10*t21*2.0+dQ1*dQ4*m6*t2*t5*t7*t9*t10*t22*2.0-dQ2*dQ3*m6*t2*t5*t8*t9*t10*t21*2.0-dQ2*dQ3*m6*t3*t5*t7*t9*t10*t21*2.0+dQ2*dQ3*m6*t5*t6*t7*t8*t11*t18*2.0-dQ1*dQ4*m6*t3*t5*t8*t9*t10*t21*2.0+dQ2*dQ3*m6*t2*t5*t8*t9*t10*t22*2.0+dQ2*dQ3*m6*t3*t5*t7*t9*t10*t22*2.0+dQ1*dQ4*m5*t2*t5*t7*t9*t10*t25*2.0+dQ1*dQ4*m6*t3*t5*t8*t9*t10*t22*2.0+dQ2*dQ3*m5*t2*t5*t8*t9*t10*t25*2.0;
et121 = dQ2*dQ3*m5*t3*t5*t7*t9*t10*t25*2.0-dQ2*dQ3*m6*t5*t6*t7*t8*t11*t21*2.0+dQ1*dQ4*m5*t3*t5*t8*t9*t10*t25*2.0+dQ1*dQ4*m6*t2*t5*t7*t9*t10*t26*2.0+dQ2*dQ3*m6*t2*t5*t8*t9*t10*t26*2.0+dQ2*dQ3*m6*t3*t5*t7*t9*t10*t26*2.0-dQ5*dQ6*m6*t2*t6*t8*t9*t11*t18*2.0-dQ5*dQ6*m6*t3*t6*t7*t9*t11*t18*2.0+dQ1*dQ4*m6*t3*t5*t8*t9*t10*t26*2.0+dQ5*dQ6*m6*t2*t6*t8*t9*t11*t21*2.0+dQ5*dQ6*m6*t3*t6*t7*t9*t11*t21*2.0+dQ2*dQ3*m5*t2*t3*t4*t9*t17*t35*2.0+dQ2*dQ3*m6*t2*t3*t4*t9*t18*t36*2.0+dQ2*dQ3*m6*t2*t3*t4*t9*t21*t35*2.0-dQ2*dQ3*m6*t2*t3*t4*t9*t21*t36*2.0-dQ2*dQ3*m6*t2*t3*t4*t9*t22*t35*2.0+dQ2*dQ6*m6*t2*t3*t4*t10*t18*t36*2.0;
et122 = dQ2*dQ3*m5*t2*t3*t4*t9*t25*t35*-2.0+dQ3*dQ6*m6*t2*t3*t4*t10*t18*t36*2.0-dQ4*dQ5*m6*t2*t3*t5*t10*t18*t36*2.0-dQ2*dQ3*m5*t4*t7*t8*t9*t17*t35*2.0-dQ2*dQ3*m6*t2*t3*t4*t9*t26*t35*2.0-dQ2*dQ6*m6*t2*t3*t4*t10*t21*t36*2.0+dQ5*dQ6*m6*t2*t4*t5*t8*t18*t36*2.0+dQ5*dQ6*m6*t3*t4*t5*t7*t18*t36*2.0-dQ3*dQ6*m6*t2*t3*t4*t10*t21*t36*2.0-dQ4*dQ6*m6*t2*t3*t6*t11*t18*t35*2.0-dQ1*dQ6*m6*t2*t7*t9*t10*t18*t33*4.0+dQ4*dQ5*m6*t2*t3*t5*t10*t21*t36*2.0-dQ1*dQ6*m6*t3*t8*t9*t10*t18*t32*4.0-dQ2*dQ3*m6*t4*t7*t8*t9*t18*t36*2.0-dQ5*dQ6*m6*t2*t4*t5*t8*t21*t36*2.0-dQ5*dQ6*m6*t3*t4*t5*t7*t21*t36*2.0+dQ4*dQ6*m6*t2*t3*t6*t11*t21*t35*2.0;
et123 = dQ1*dQ2*m6*t6*t9*t10*t11*t18*t32*-4.0-dQ1*dQ6*m6*t2*t7*t9*t10*t18*t36*4.0+dQ1*dQ6*m6*t2*t7*t9*t10*t21*t33*4.0-dQ2*dQ3*m6*t4*t7*t8*t9*t21*t35*2.0-dQ1*dQ2*m6*t6*t9*t10*t11*t18*t33*4.0-dQ1*dQ3*m6*t6*t9*t10*t11*t18*t32*4.0+dQ1*dQ6*m6*t3*t8*t9*t10*t21*t32*4.0+dQ2*dQ3*m6*t4*t7*t8*t9*t21*t36*2.0+dQ2*dQ3*m6*t4*t7*t8*t9*t22*t35*2.0-dQ1*dQ3*m6*t6*t9*t10*t11*t18*t33*4.0-dQ1*dQ6*m6*t3*t8*t9*t10*t18*t36*4.0-dQ2*dQ6*m6*t4*t7*t8*t10*t18*t36*2.0+dQ1*dQ2*m6*t6*t9*t10*t11*t21*t32*4.0+dQ1*dQ6*m6*t2*t7*t9*t10*t21*t36*4.0+dQ2*dQ3*m5*t4*t7*t8*t9*t25*t35*2.0-dQ3*dQ6*m6*t4*t7*t8*t10*t18*t36*2.0+dQ1*dQ2*m6*t6*t9*t10*t11*t21*t33*4.0;
et124 = dQ1*dQ3*m6*t6*t9*t10*t11*t21*t32*4.0+dQ4*dQ5*m6*t5*t7*t8*t10*t18*t36*2.0+dQ4*dQ6*m6*t2*t8*t9*t10*t18*t36*2.0+dQ4*dQ6*m6*t3*t7*t9*t10*t18*t36*2.0+dQ1*dQ3*m6*t6*t9*t10*t11*t21*t33*4.0+dQ1*dQ6*m6*t3*t8*t9*t10*t21*t36*4.0+dQ2*dQ3*m6*t4*t7*t8*t9*t26*t35*2.0+dQ2*dQ6*m6*t4*t7*t8*t10*t21*t36*2.0+dQ3*dQ6*m6*t4*t7*t8*t10*t21*t36*2.0+dQ4*dQ6*m6*t6*t7*t8*t11*t18*t35*2.0-dQ4*dQ5*m6*t5*t7*t8*t10*t21*t36*2.0-dQ4*dQ6*m6*t2*t8*t9*t10*t21*t36*2.0-dQ4*dQ6*m6*t3*t7*t9*t10*t21*t36*2.0-dQ4*dQ6*m6*t6*t7*t8*t11*t21*t35*2.0-dQ1*dQ2*m5*t4*t5*t10*t17*t32*t33*8.0-dQ1*dQ5*m5*t2*t4*t7*t17*t33*t35*8.0-dQ1*dQ3*m5*t4*t5*t10*t17*t32*t33*8.0;
et125 = dQ1*dQ5*m5*t3*t4*t8*t17*t32*t35*-8.0+dQ1*dQ5*m6*t2*t4*t7*t18*t33*t36*4.0+dQ1*dQ5*m6*t3*t4*t8*t18*t32*t36*4.0+dQ1*dQ2*m6*t4*t5*t10*t18*t32*t36*4.0-dQ1*dQ2*m6*t4*t5*t10*t21*t32*t33*8.0+dQ1*dQ5*m6*t2*t4*t7*t18*t35*t36*4.0-dQ1*dQ5*m6*t2*t4*t7*t21*t33*t35*8.0+dQ1*dQ6*m6*t4*t5*t9*t18*t32*t33*4.0+dQ1*dQ2*m6*t4*t5*t10*t18*t33*t36*4.0+dQ1*dQ2*m6*t4*t5*t10*t22*t32*t33*8.0+dQ1*dQ3*m6*t4*t5*t10*t18*t32*t36*4.0-dQ1*dQ3*m6*t4*t5*t10*t21*t32*t33*8.0-dQ1*dQ5*m6*t2*t4*t7*t21*t33*t36*4.0+dQ1*dQ5*m6*t2*t4*t7*t22*t33*t35*8.0-dQ1*dQ5*m6*t3*t4*t8*t21*t32*t35*8.0+dQ1*dQ3*m6*t4*t5*t10*t18*t33*t36*4.0;
et126 = dQ1*dQ3*m6*t4*t5*t10*t22*t32*t33*8.0+dQ1*dQ4*m6*t5*t6*t11*t18*t32*t33*4.0+dQ1*dQ5*m6*t3*t4*t8*t18*t35*t36*4.0-dQ1*dQ5*m6*t3*t4*t8*t21*t32*t36*4.0+dQ1*dQ5*m6*t3*t4*t8*t22*t32*t35*8.0+dQ2*dQ5*m6*t2*t3*t9*t18*t35*t36*2.0+dQ1*dQ2*m5*t4*t5*t10*t25*t32*t33*8.0-dQ1*dQ2*m6*t4*t5*t10*t21*t32*t36*4.0+dQ1*dQ4*m6*t5*t6*t11*t18*t32*t34*4.0+dQ1*dQ5*m5*t2*t4*t7*t25*t33*t35*8.0-dQ1*dQ5*m6*t2*t4*t7*t21*t35*t36*4.0+dQ1*dQ6*m6*t4*t5*t9*t18*t32*t36*4.0-dQ1*dQ6*m6*t4*t5*t9*t21*t32*t33*4.0+dQ2*dQ6*m6*t2*t5*t8*t18*t34*t36*4.0+dQ2*dQ6*m6*t3*t5*t7*t18*t34*t36*4.0+dQ3*dQ5*m6*t2*t3*t9*t18*t35*t36*2.0-dQ1*dQ2*m6*t4*t5*t10*t21*t33*t36*4.0;
et127 = dQ1*dQ3*m5*t4*t5*t10*t25*t32*t33*8.0-dQ1*dQ3*m6*t4*t5*t10*t21*t32*t36*4.0+dQ1*dQ4*m6*t5*t6*t11*t18*t33*t34*4.0+dQ1*dQ5*m5*t3*t4*t8*t25*t32*t35*8.0+dQ1*dQ6*m6*t4*t5*t9*t18*t33*t36*4.0+dQ3*dQ6*m6*t2*t5*t8*t18*t34*t36*4.0+dQ3*dQ6*m6*t3*t5*t7*t18*t34*t36*4.0-dQ4*dQ5*m6*t2*t4*t8*t18*t35*t36*2.0-dQ4*dQ5*m6*t3*t4*t7*t18*t35*t36*2.0+dQ1*dQ2*m6*t4*t5*t10*t26*t32*t33*8.0-dQ1*dQ3*m6*t4*t5*t10*t21*t33*t36*4.0-dQ1*dQ4*m6*t5*t6*t11*t21*t32*t33*4.0+dQ1*dQ5*m6*t2*t4*t7*t26*t33*t35*8.0-dQ1*dQ5*m6*t3*t4*t8*t21*t35*t36*4.0-dQ2*dQ5*m6*t2*t3*t9*t21*t35*t36*2.0+dQ1*dQ3*m6*t4*t5*t10*t26*t32*t33*8.0-dQ1*dQ4*m6*t5*t6*t11*t21*t32*t34*4.0;
et128 = dQ1*dQ5*m6*t3*t4*t8*t26*t32*t35*8.0-dQ1*dQ6*m6*t4*t5*t9*t21*t32*t36*4.0-dQ2*dQ6*m6*t2*t5*t8*t21*t34*t36*4.0-dQ2*dQ6*m6*t3*t5*t7*t21*t34*t36*4.0-dQ3*dQ5*m6*t2*t3*t9*t21*t35*t36*2.0-dQ1*dQ4*m6*t5*t6*t11*t21*t33*t34*4.0-dQ1*dQ6*m6*t4*t5*t9*t21*t33*t36*4.0-dQ3*dQ6*m6*t2*t5*t8*t21*t34*t36*4.0-dQ3*dQ6*m6*t3*t5*t7*t21*t34*t36*4.0+dQ4*dQ5*m6*t2*t4*t8*t21*t35*t36*2.0+dQ4*dQ5*m6*t3*t4*t7*t21*t35*t36*2.0-dQ2*dQ5*m6*t7*t8*t9*t18*t35*t36*2.0-dQ3*dQ5*m6*t7*t8*t9*t18*t35*t36*2.0+dQ2*dQ5*m6*t7*t8*t9*t21*t35*t36*2.0+dQ3*dQ5*m6*t7*t8*t9*t21*t35*t36*2.0-dQ1*dQ2*m5*t2*t7*t17*t33*t34*t35*4.0-dQ1*dQ2*m5*t3*t8*t17*t32*t34*t35*4.0;
et129 = dQ1*dQ3*m5*t2*t7*t17*t33*t34*t35*-4.0-dQ1*dQ3*m5*t3*t8*t17*t32*t34*t35*4.0-dQ1*dQ2*m6*t2*t7*t18*t33*t34*t36*4.0-dQ1*dQ2*m6*t2*t7*t18*t33*t35*t36*4.0-dQ1*dQ2*m6*t3*t8*t18*t32*t34*t36*4.0-dQ1*dQ3*m6*t2*t7*t18*t33*t34*t36*4.0-dQ1*dQ4*m5*t4*t9*t17*t32*t33*t35*4.0+dQ1*dQ2*m6*t2*t7*t18*t34*t35*t36*2.0-dQ1*dQ2*m6*t2*t7*t21*t33*t34*t35*4.0-dQ1*dQ2*m6*t3*t8*t18*t32*t35*t36*4.0-dQ1*dQ3*m6*t2*t7*t18*t33*t35*t36*4.0-dQ1*dQ3*m6*t3*t8*t18*t32*t34*t36*4.0+dQ1*dQ2*m6*t2*t7*t21*t33*t34*t36*4.0+dQ1*dQ2*m6*t2*t7*t22*t33*t34*t35*4.0-dQ1*dQ2*m6*t3*t8*t21*t32*t34*t35*4.0+dQ1*dQ3*m6*t2*t7*t18*t34*t35*t36*2.0-dQ1*dQ3*m6*t2*t7*t21*t33*t34*t35*4.0;
et130 = dQ1*dQ3*m6*t3*t8*t18*t32*t35*t36*-4.0-dQ1*dQ5*m5*t5*t10*t17*t32*t33*t34*4.0+dQ1*dQ2*m6*t2*t7*t21*t33*t35*t36*4.0+dQ1*dQ2*m6*t3*t8*t18*t34*t35*t36*2.0+dQ1*dQ2*m6*t3*t8*t21*t32*t34*t36*4.0+dQ1*dQ2*m6*t3*t8*t22*t32*t34*t35*4.0+dQ1*dQ3*m6*t2*t7*t21*t33*t34*t36*4.0+dQ1*dQ3*m6*t2*t7*t22*t33*t34*t35*4.0-dQ1*dQ3*m6*t3*t8*t21*t32*t34*t35*4.0-dQ1*dQ4*m6*t4*t9*t18*t32*t33*t36*4.0+dQ1*dQ2*m5*t2*t7*t25*t33*t34*t35*4.0-dQ1*dQ2*m6*t2*t7*t21*t34*t35*t36*2.0+dQ1*dQ2*m6*t3*t8*t21*t32*t35*t36*4.0+dQ1*dQ3*m6*t2*t7*t21*t33*t35*t36*4.0+dQ1*dQ3*m6*t3*t8*t18*t34*t35*t36*2.0+dQ1*dQ3*m6*t3*t8*t21*t32*t34*t36*4.0+dQ1*dQ3*m6*t3*t8*t22*t32*t34*t35*4.0;
et131 = dQ1*dQ2*m5*t3*t8*t25*t32*t34*t35*4.0+dQ1*dQ3*m5*t2*t7*t25*t33*t34*t35*4.0-dQ1*dQ3*m6*t2*t7*t21*t34*t35*t36*2.0+dQ1*dQ3*m6*t3*t8*t21*t32*t35*t36*4.0+dQ1*dQ4*m6*t4*t9*t18*t32*t35*t36*2.0-dQ1*dQ4*m6*t4*t9*t21*t32*t33*t35*4.0+dQ2*dQ4*m6*t2*t8*t18*t34*t35*t36*2.0+dQ2*dQ4*m6*t3*t7*t18*t34*t35*t36*2.0+dQ1*dQ2*m6*t2*t7*t26*t33*t34*t35*4.0-dQ1*dQ2*m6*t3*t8*t21*t34*t35*t36*2.0+dQ1*dQ3*m5*t3*t8*t25*t32*t34*t35*4.0+dQ1*dQ4*m6*t4*t9*t18*t33*t35*t36*2.0+dQ1*dQ4*m6*t4*t9*t21*t32*t33*t36*4.0+dQ1*dQ4*m6*t4*t9*t22*t32*t33*t35*4.0-dQ1*dQ5*m6*t5*t10*t18*t32*t33*t36*4.0+dQ3*dQ4*m6*t2*t8*t18*t34*t35*t36*2.0+dQ3*dQ4*m6*t3*t7*t18*t34*t35*t36*2.0;
et132 = dQ1*dQ2*m6*t3*t8*t26*t32*t34*t35*4.0+dQ1*dQ3*m6*t2*t7*t26*t33*t34*t35*4.0-dQ1*dQ3*m6*t3*t8*t21*t34*t35*t36*2.0+dQ1*dQ5*m6*t5*t10*t18*t32*t34*t36*2.0-dQ1*dQ5*m6*t5*t10*t21*t32*t33*t34*4.0-dQ1*dQ6*m6*t6*t11*t18*t32*t33*t34*4.0+dQ1*dQ3*m6*t3*t8*t26*t32*t34*t35*4.0+dQ1*dQ4*m5*t4*t9*t25*t32*t33*t35*4.0-dQ1*dQ4*m6*t4*t9*t21*t32*t35*t36*2.0+dQ1*dQ5*m6*t5*t10*t18*t33*t34*t36*2.0+dQ1*dQ5*m6*t5*t10*t22*t32*t33*t34*4.0-dQ1*dQ6*m6*t6*t11*t18*t32*t33*t35*4.0-dQ2*dQ4*m6*t2*t8*t21*t34*t35*t36*2.0-dQ2*dQ4*m6*t3*t7*t21*t34*t35*t36*2.0-dQ1*dQ4*m6*t4*t9*t21*t33*t35*t36*2.0+dQ1*dQ5*m6*t5*t10*t21*t32*t33*t36*4.0+dQ1*dQ6*m6*t6*t11*t18*t32*t34*t35*2.0;
et133 = dQ3*dQ4*m6*t2*t8*t21*t34*t35*t36*-2.0-dQ3*dQ4*m6*t3*t7*t21*t34*t35*t36*2.0+dQ1*dQ4*m6*t4*t9*t26*t32*t33*t35*4.0+dQ1*dQ5*m5*t5*t10*t25*t32*t33*t34*4.0-dQ1*dQ5*m6*t5*t10*t21*t32*t34*t36*2.0+dQ1*dQ6*m6*t6*t11*t18*t33*t34*t35*2.0+dQ1*dQ6*m6*t6*t11*t21*t32*t33*t34*4.0-dQ1*dQ5*m6*t5*t10*t21*t33*t34*t36*2.0+dQ1*dQ6*m6*t6*t11*t21*t32*t33*t35*4.0+dQ1*dQ5*m6*t5*t10*t26*t32*t33*t34*4.0-dQ1*dQ6*m6*t6*t11*t21*t32*t34*t35*2.0-dQ1*dQ6*m6*t6*t11*t21*t33*t34*t35*2.0-Lx2*Lx4*dQ1*dQ2*m4*t2*t3*t4*t7*4.0-Lx2*Lx4*dQ1*dQ2*m5*t2*t3*t4*t7*4.0-Lx2*Lx4*dQ1*dQ3*m4*t2*t3*t4*t7*2.0-Lx2*Lx4*dQ1*dQ2*m6*t2*t3*t4*t7*4.0-Lx2*Lx4*dQ1*dQ3*m5*t2*t3*t4*t7*2.0;
et134 = Lx2*Lx4*dQ1*dQ3*m6*t2*t3*t4*t7*-2.0+Lx2*Lx4*dQ1*dQ4*m4*t2*t7*t8*t9*2.0+Lx2*Lx4*dQ1*dQ4*m5*t2*t7*t8*t9*2.0+Lx2*Lx4*dQ1*dQ4*m6*t2*t7*t8*t9*2.0-Lx3*Lx4*dQ1*dQ2*m4*t2*t4*t7*t33*8.0-Lx3*Lx4*dQ1*dQ2*m4*t3*t4*t8*t32*8.0-Lx3*Lx4*dQ1*dQ2*m5*t2*t4*t7*t33*8.0-Lx3*Lx4*dQ1*dQ3*m4*t2*t4*t7*t33*8.0-Lx3*Lx4*dQ1*dQ2*m5*t3*t4*t8*t32*8.0-Lx3*Lx4*dQ1*dQ2*m6*t2*t4*t7*t33*8.0-Lx3*Lx4*dQ1*dQ3*m4*t3*t4*t8*t32*8.0-Lx3*Lx4*dQ1*dQ3*m5*t2*t4*t7*t33*8.0-Lx3*Lx4*dQ1*dQ2*m6*t3*t4*t8*t32*8.0-Lx3*Lx4*dQ1*dQ3*m5*t3*t4*t8*t32*8.0-Lx3*Lx4*dQ1*dQ3*m6*t2*t4*t7*t33*8.0;
et135 = Lx3*Lx4*dQ1*dQ3*m6*t3*t4*t8*t32*-8.0-Lx2*Lxcm4*dQ1*dQ2*m4*t2*t3*t4*t7*4.0-Lx2*Lxcm4*dQ1*dQ3*m4*t2*t3*t4*t7*2.0+Lx3*Lxcm5*dQ1*dQ2*m5*t2*t4*t5*t7*4.0-Lx2*Lxcm5*dQ1*dQ5*m5*t2*t3*t5*t7*2.0+Lx3*Lxcm5*dQ1*dQ3*m5*t2*t4*t5*t7*4.0+Lx4*Lxcm4*dQ2*dQ3*m4*t2*t3*t4*t9*4.0+Lx3*Lxcm5*dQ1*dQ2*m5*t3*t4*t5*t8*4.0+Lx3*Lxcm5*dQ1*dQ3*m5*t3*t4*t5*t8*4.0+Lx3*Lxcm5*dQ2*dQ3*m5*t2*t3*t5*t9*2.0+Lx4*Lxcm5*dQ1*dQ5*m5*t2*t4*t5*t7*2.0+Lx2*Lxcm6*dQ1*dQ2*m6*t4*t5*t6*t8*2.0+Lx3*Lxcm6*dQ2*dQ3*m6*t2*t3*t4*t11*2.0+Lx4*Lxcm5*dQ1*dQ5*m5*t3*t4*t5*t8*2.0+Lx4*Lxcm5*dQ2*dQ5*m5*t2*t3*t5*t9*2.0+Lx2*Lxcm4*dQ1*dQ4*m4*t2*t7*t8*t9*2.0-Lx3*Lxcm5*dQ4*dQ5*m5*t2*t3*t4*t10*2.0;
et136 = Lx3*Lxcm6*dQ1*dQ5*m6*t2*t5*t6*t7*2.0+Lx4*Lxcm5*dQ3*dQ5*m5*t2*t3*t5*t9*2.0+Lx2*Lxcm5*dQ1*dQ2*m5*t2*t7*t8*t10*4.0+Lx2*Lxcm5*dQ1*dQ3*m5*t2*t7*t8*t10*2.0+Lx3*Lxcm6*dQ1*dQ5*m6*t3*t5*t6*t8*2.0-Lx4*Lxcm6*dQ2*dQ4*m6*t2*t5*t6*t8*4.0-Lx4*Lxcm6*dQ2*dQ4*m6*t3*t5*t6*t7*4.0-Lx4*Lxcm6*dQ3*dQ4*m6*t2*t5*t6*t8*4.0-Lx4*Lxcm6*dQ3*dQ4*m6*t3*t5*t6*t7*4.0-Lx2*Lxcm6*dQ4*dQ5*m6*t2*t4*t6*t10*2.0-Lx3*Lxcm6*dQ4*dQ6*m6*t2*t3*t6*t9*2.0-Lx4*Lxcm4*dQ2*dQ3*m4*t4*t7*t8*t9*4.0-Lx2*Lxcm6*dQ4*dQ6*m6*t2*t4*t5*t11*2.0-Lx4*Lxcm6*dQ4*dQ5*m6*t2*t3*t6*t10*2.0-Lx3*Lxcm5*dQ2*dQ3*m5*t5*t7*t8*t9*2.0-Lx3*Lxcm6*dQ1*dQ2*m6*t2*t7*t9*t11*4.0-Lx4*Lxcm5*dQ1*dQ4*m5*t2*t7*t9*t10*2.0;
et137 = Lx4*Lxcm6*dQ4*dQ6*m6*t2*t3*t5*t11*-2.0-Lx3*Lxcm6*dQ1*dQ3*m6*t2*t7*t9*t11*4.0-Lx4*Lxcm5*dQ2*dQ3*m5*t2*t8*t9*t10*2.0-Lx4*Lxcm5*dQ2*dQ3*m5*t3*t7*t9*t10*2.0-Lx3*Lxcm6*dQ1*dQ2*m6*t3*t8*t9*t11*4.0-Lx4*Lxcm5*dQ1*dQ4*m5*t3*t8*t9*t10*2.0-Lx3*Lxcm6*dQ1*dQ3*m6*t3*t8*t9*t11*4.0-Lx3*Lxcm6*dQ2*dQ3*m6*t4*t7*t8*t11*2.0-Lx4*Lxcm5*dQ2*dQ5*m5*t5*t7*t8*t9*2.0+Lx3*Lxcm5*dQ4*dQ5*m5*t4*t7*t8*t10*2.0-Lx4*Lxcm5*dQ3*dQ5*m5*t5*t7*t8*t9*2.0-Lx3*Lxcm6*dQ1*dQ6*m6*t2*t7*t10*t11*2.0-Lx3*Lxcm6*dQ1*dQ6*m6*t3*t8*t10*t11*2.0+Lx3*Lxcm6*dQ4*dQ6*m6*t6*t7*t8*t9*2.0+Lx4*Lxcm6*dQ4*dQ5*m6*t6*t7*t8*t10*2.0+Lx2*Lxcm6*dQ5*dQ6*m6*t2*t9*t10*t11*2.0+Lx4*Lxcm6*dQ4*dQ6*m6*t5*t7*t8*t11*2.0;
et138 = Lx3*Lxcm4*dQ1*dQ2*m4*t2*t4*t7*t33*-8.0-Lx3*Lxcm4*dQ1*dQ2*m4*t3*t4*t8*t32*8.0-Lx3*Lxcm4*dQ1*dQ3*m4*t2*t4*t7*t33*8.0-Lx3*Lxcm4*dQ1*dQ3*m4*t3*t4*t8*t32*8.0-Lx2*Lxcm5*dQ1*dQ2*m5*t4*t5*t8*t32*4.0-Lx2*Lxcm5*dQ1*dQ3*m5*t4*t5*t8*t32*2.0+Lx4*Lxcm5*dQ1*dQ2*m5*t2*t5*t7*t34*4.0-Lx2*Lxcm5*dQ1*dQ4*m5*t3*t5*t9*t32*2.0-Lx3*Lxcm5*dQ1*dQ5*m5*t2*t5*t7*t33*4.0+Lx4*Lxcm5*dQ1*dQ3*m5*t2*t5*t7*t34*4.0-Lx2*Lxcm5*dQ1*dQ5*m5*t3*t4*t10*t32*2.0-Lx3*Lxcm5*dQ1*dQ5*m5*t3*t5*t8*t32*4.0+Lx4*Lxcm5*dQ1*dQ2*m5*t3*t5*t8*t34*4.0-Lx2*Lxcm6*dQ1*dQ2*m6*t3*t6*t10*t32*4.0+Lx4*Lxcm5*dQ1*dQ3*m5*t3*t5*t8*t34*4.0-Lx2*Lxcm6*dQ1*dQ3*m6*t3*t6*t10*t32*2.0;
et139 = Lx2*Lxcm6*dQ1*dQ4*m6*t3*t4*t11*t32*-2.0+Lx4*Lxcm5*dQ1*dQ4*m5*t4*t5*t9*t32*4.0+Lx4*Lxcm5*dQ2*dQ4*m5*t2*t5*t8*t34*4.0+Lx4*Lxcm5*dQ2*dQ4*m5*t3*t5*t7*t34*4.0+Lx4*Lxcm5*dQ1*dQ4*m5*t4*t5*t9*t33*4.0+Lx4*Lxcm5*dQ3*dQ4*m5*t2*t5*t8*t34*4.0+Lx4*Lxcm5*dQ3*dQ4*m5*t3*t5*t7*t34*4.0-Lx2*Lxcm6*dQ1*dQ5*m6*t5*t6*t8*t32*2.0-Lx2*Lxcm6*dQ1*dQ6*m6*t3*t6*t9*t32*2.0+Lx4*Lxcm6*dQ1*dQ2*m6*t4*t6*t10*t32*4.0+Lx4*Lxcm6*dQ2*dQ3*m6*t2*t3*t11*t34*4.0+Lx3*Lxcm6*dQ1*dQ4*m6*t5*t6*t9*t32*2.0+Lx4*Lxcm6*dQ1*dQ2*m6*t4*t6*t10*t33*4.0+Lx4*Lxcm6*dQ1*dQ3*m6*t4*t6*t10*t32*4.0+Lx3*Lxcm6*dQ1*dQ4*m6*t5*t6*t9*t33*2.0+Lx3*Lxcm6*dQ1*dQ5*m6*t4*t6*t10*t32*2.0+Lx4*Lxcm6*dQ1*dQ3*m6*t4*t6*t10*t33*4.0;
et140 = Lx3*Lxcm6*dQ1*dQ5*m6*t4*t6*t10*t33*2.0+Lx3*Lxcm6*dQ1*dQ6*m6*t4*t5*t11*t32*2.0+Lx4*Lxcm6*dQ1*dQ6*m6*t4*t6*t9*t32*2.0+Lx4*Lxcm6*dQ2*dQ6*m6*t2*t6*t8*t34*2.0+Lx4*Lxcm6*dQ2*dQ6*m6*t3*t6*t7*t34*2.0+Lx3*Lxcm6*dQ1*dQ6*m6*t4*t5*t11*t33*2.0+Lx4*Lxcm6*dQ1*dQ6*m6*t4*t6*t9*t33*2.0+Lx4*Lxcm6*dQ3*dQ6*m6*t2*t6*t8*t34*2.0+Lx4*Lxcm6*dQ3*dQ6*m6*t3*t6*t7*t34*2.0+Lx2*Lxcm6*dQ1*dQ2*m6*t8*t9*t11*t32*4.0+Lx2*Lxcm6*dQ1*dQ3*m6*t8*t9*t11*t32*2.0-Lx4*Lxcm6*dQ2*dQ3*m6*t7*t8*t11*t34*4.0+Lx2*Lxcm6*dQ1*dQ6*m6*t8*t10*t11*t32*2.0-Lx4*Lxcm4*dQ1*dQ2*m4*t2*t7*t33*t34*8.0-Lx4*Lxcm4*dQ1*dQ2*m4*t3*t8*t32*t34*8.0-Lx4*Lxcm4*dQ1*dQ3*m4*t2*t7*t33*t34*8.0-Lx4*Lxcm4*dQ1*dQ3*m4*t3*t8*t32*t34*8.0;
et141 = Lx4*Lxcm4*dQ1*dQ4*m4*t4*t9*t32*t33*-8.0-Lx4*Lxcm5*dQ1*dQ2*m5*t4*t10*t32*t33*8.0-Lx3*Lxcm5*dQ1*dQ4*m5*t5*t9*t32*t33*4.0-Lx4*Lxcm5*dQ1*dQ3*m5*t4*t10*t32*t33*8.0-Lx3*Lxcm5*dQ1*dQ5*m5*t4*t10*t32*t33*4.0-Lx3*Lxcm6*dQ1*dQ2*m6*t6*t10*t32*t33*8.0-Lx3*Lxcm6*dQ1*dQ3*m6*t6*t10*t32*t33*8.0-Lx3*Lxcm6*dQ1*dQ4*m6*t4*t11*t32*t33*4.0-Lx3*Lxcm6*dQ1*dQ6*m6*t6*t9*t32*t33*4.0+Lx4*Lxcm6*dQ1*dQ5*m6*t6*t10*t32*t34*2.0+Lx4*Lxcm6*dQ1*dQ5*m6*t6*t10*t33*t34*2.0+Lx4*Lxcm6*dQ1*dQ6*m6*t5*t11*t32*t34*2.0+Lx4*Lxcm6*dQ1*dQ6*m6*t5*t11*t33*t34*2.0-Lx4*Lxcm5*dQ1*dQ5*m5*t10*t32*t33*t34*4.0-Lx4*Lxcm6*dQ1*dQ4*m6*t11*t32*t33*t34*8.0+Lx2*Lycm4*dQ1*dQ2*m4*t2*t3*t7*t9*4.0;
et142 = Lx2*Lycm4*dQ1*dQ3*m4*t2*t3*t7*t9*2.0+Lx3*Lycm6*dQ2*dQ3*m6*t2*t3*t4*t6*2.0+Lx2*Lycm4*dQ1*dQ4*m4*t2*t4*t7*t8*2.0+Lx2*Lycm5*dQ1*dQ2*m5*t2*t3*t7*t9*4.0+Lx2*Lycm5*dQ1*dQ3*m5*t2*t3*t7*t9*2.0-Lx4*Lycm4*dQ1*dQ2*m4*t2*t4*t7*t9*4.0-Lx4*Lycm4*dQ1*dQ4*m4*t2*t3*t7*t8*4.0+Lx2*Lycm5*dQ1*dQ4*m5*t2*t4*t7*t8*2.0-Lx4*Lycm4*dQ1*dQ3*m4*t2*t4*t7*t9*4.0-Lx4*Lycm4*dQ1*dQ2*m4*t3*t4*t8*t9*4.0-Lx4*Lycm5*dQ1*dQ2*m5*t2*t4*t7*t9*4.0-Lx4*Lycm5*dQ1*dQ4*m5*t2*t3*t7*t8*4.0-Lx4*Lycm4*dQ1*dQ3*m4*t3*t4*t8*t9*4.0-Lx4*Lycm5*dQ1*dQ3*m5*t2*t4*t7*t9*4.0-Lx2*Lycm6*dQ4*dQ6*m6*t2*t4*t5*t6*2.0-Lx4*Lycm4*dQ2*dQ4*m4*t2*t4*t8*t9*4.0-Lx4*Lycm4*dQ2*dQ4*m4*t3*t4*t7*t9*4.0;
et143 = Lx4*Lycm5*dQ1*dQ2*m5*t3*t4*t8*t9*-4.0-Lx3*Lycm6*dQ1*dQ2*m6*t2*t6*t7*t9*4.0-Lx4*Lycm4*dQ3*dQ4*m4*t2*t4*t8*t9*4.0-Lx4*Lycm4*dQ3*dQ4*m4*t3*t4*t7*t9*4.0-Lx4*Lycm5*dQ1*dQ3*m5*t3*t4*t8*t9*4.0-Lx4*Lycm6*dQ4*dQ6*m6*t2*t3*t5*t6*2.0-Lx3*Lycm6*dQ1*dQ3*m6*t2*t6*t7*t9*4.0-Lx4*Lycm5*dQ2*dQ4*m5*t2*t4*t8*t9*4.0-Lx4*Lycm5*dQ2*dQ4*m5*t3*t4*t7*t9*4.0-Lx3*Lycm6*dQ1*dQ2*m6*t3*t6*t8*t9*4.0-Lx4*Lycm5*dQ3*dQ4*m5*t2*t4*t8*t9*4.0-Lx4*Lycm5*dQ3*dQ4*m5*t3*t4*t7*t9*4.0-Lx2*Lycm6*dQ1*dQ2*m6*t4*t5*t8*t11*2.0-Lx3*Lycm6*dQ1*dQ3*m6*t3*t6*t8*t9*4.0-Lx3*Lycm6*dQ2*dQ3*m6*t4*t6*t7*t8*2.0-Lx3*Lycm6*dQ1*dQ5*m6*t2*t5*t7*t11*2.0;
et144 = Lx3*Lycm6*dQ1*dQ6*m6*t2*t6*t7*t10*-2.0-Lx3*Lycm6*dQ1*dQ5*m6*t3*t5*t8*t11*2.0+Lx4*Lycm6*dQ2*dQ4*m6*t2*t5*t8*t11*4.0+Lx4*Lycm6*dQ2*dQ4*m6*t3*t5*t7*t11*4.0-Lx3*Lycm6*dQ1*dQ6*m6*t3*t6*t8*t10*2.0+Lx4*Lycm6*dQ3*dQ4*m6*t2*t5*t8*t11*4.0+Lx4*Lycm6*dQ3*dQ4*m6*t3*t5*t7*t11*4.0+Lx2*Lycm6*dQ4*dQ5*m6*t2*t4*t10*t11*2.0+Lx3*Lycm6*dQ4*dQ6*m6*t2*t3*t9*t11*2.0+Lx4*Lycm6*dQ4*dQ5*m6*t2*t3*t10*t11*2.0+Lx2*Lycm6*dQ5*dQ6*m6*t2*t6*t9*t10*2.0+Lx4*Lycm6*dQ4*dQ6*m6*t5*t6*t7*t8*2.0-Lx3*Lycm6*dQ4*dQ6*m6*t7*t8*t9*t11*2.0-Lx4*Lycm6*dQ4*dQ5*m6*t7*t8*t10*t11*2.0-Lx2*Lycm6*dQ1*dQ4*m6*t3*t4*t6*t32*2.0+Lx3*Lycm4*dQ1*dQ2*m4*t2*t7*t9*t33*8.0+Lx3*Lycm4*dQ1*dQ2*m4*t3*t8*t9*t32*8.0;
et145 = Lx3*Lycm4*dQ1*dQ3*m4*t2*t7*t9*t33*8.0+Lx4*Lycm6*dQ2*dQ3*m6*t2*t3*t6*t34*4.0+Lx3*Lycm4*dQ1*dQ3*m4*t3*t8*t9*t32*8.0+Lx3*Lycm5*dQ1*dQ2*m5*t2*t7*t9*t33*8.0+Lx3*Lycm5*dQ1*dQ2*m5*t3*t8*t9*t32*8.0+Lx3*Lycm5*dQ1*dQ3*m5*t2*t7*t9*t33*8.0+Lx3*Lycm5*dQ1*dQ3*m5*t3*t8*t9*t32*8.0+Lx3*Lycm6*dQ1*dQ6*m6*t4*t5*t6*t32*2.0+Lx3*Lycm6*dQ1*dQ6*m6*t4*t5*t6*t33*2.0+Lx2*Lycm6*dQ1*dQ2*m6*t6*t8*t9*t32*4.0+Lx2*Lycm6*dQ1*dQ2*m6*t3*t10*t11*t32*4.0+Lx2*Lycm6*dQ1*dQ3*m6*t6*t8*t9*t32*2.0+Lx2*Lycm6*dQ1*dQ3*m6*t3*t10*t11*t32*2.0+Lx2*Lycm6*dQ1*dQ5*m6*t5*t8*t11*t32*2.0+Lx2*Lycm6*dQ1*dQ6*m6*t3*t9*t11*t32*2.0-Lx4*Lycm6*dQ1*dQ2*m6*t4*t10*t11*t32*4.0-Lx4*Lycm6*dQ2*dQ3*m6*t6*t7*t8*t34*4.0;
et146 = Lx2*Lycm6*dQ1*dQ6*m6*t6*t8*t10*t32*2.0-Lx3*Lycm6*dQ1*dQ4*m6*t5*t9*t11*t32*2.0-Lx4*Lycm6*dQ1*dQ2*m6*t4*t10*t11*t33*4.0-Lx4*Lycm6*dQ1*dQ3*m6*t4*t10*t11*t32*4.0-Lx3*Lycm6*dQ1*dQ4*m6*t5*t9*t11*t33*2.0-Lx3*Lycm6*dQ1*dQ5*m6*t4*t10*t11*t32*2.0-Lx4*Lycm6*dQ1*dQ3*m6*t4*t10*t11*t33*4.0-Lx3*Lycm6*dQ1*dQ5*m6*t4*t10*t11*t33*2.0-Lx4*Lycm6*dQ1*dQ6*m6*t4*t9*t11*t32*2.0-Lx4*Lycm6*dQ2*dQ6*m6*t2*t8*t11*t34*2.0-Lx4*Lycm6*dQ2*dQ6*m6*t3*t7*t11*t34*2.0-Lx4*Lycm6*dQ1*dQ6*m6*t4*t9*t11*t33*2.0-Lx4*Lycm6*dQ3*dQ6*m6*t2*t8*t11*t34*2.0-Lx4*Lycm6*dQ3*dQ6*m6*t3*t7*t11*t34*2.0-Lx3*Lycm6*dQ1*dQ4*m6*t4*t6*t32*t33*4.0+Lx4*Lycm6*dQ1*dQ6*m6*t5*t6*t32*t34*2.0;
et147 = Lx4*Lycm6*dQ1*dQ6*m6*t5*t6*t33*t34*2.0+Lx3*Lycm6*dQ1*dQ2*m6*t10*t11*t32*t33*8.0+Lx3*Lycm6*dQ1*dQ3*m6*t10*t11*t32*t33*8.0+Lx3*Lycm6*dQ1*dQ6*m6*t9*t11*t32*t33*4.0-Lx4*Lycm6*dQ1*dQ5*m6*t10*t11*t32*t34*2.0-Lx4*Lycm6*dQ1*dQ5*m6*t10*t11*t33*t34*2.0-Lx4*Lycm6*dQ1*dQ4*m6*t6*t32*t33*t34*8.0+Lxcm5*Lycm5*dQ2*dQ5*m5*t2*t3*t4*t5*2.0-Lxcm4*Lycm4*dQ1*dQ2*m4*t2*t4*t7*t9*4.0-Lxcm4*Lycm4*dQ1*dQ4*m4*t2*t3*t7*t8*4.0+Lxcm5*Lycm5*dQ3*dQ5*m5*t2*t3*t4*t5*2.0-Lxcm4*Lycm4*dQ1*dQ3*m4*t2*t4*t7*t9*4.0-Lxcm4*Lycm4*dQ1*dQ2*m4*t3*t4*t8*t9*4.0-Lxcm6*Lycm6*dQ2*dQ5*m6*t2*t3*t4*t5*2.0-Lxcm4*Lycm4*dQ1*dQ3*m4*t3*t4*t8*t9*4.0-Lxcm6*Lycm6*dQ3*dQ5*m6*t2*t3*t4*t5*2.0;
et148 = Lxcm4*Lycm4*dQ2*dQ4*m4*t2*t4*t8*t9*-4.0-Lxcm4*Lycm4*dQ2*dQ4*m4*t3*t4*t7*t9*4.0-Lxcm4*Lycm4*dQ3*dQ4*m4*t2*t4*t8*t9*4.0-Lxcm4*Lycm4*dQ3*dQ4*m4*t3*t4*t7*t9*4.0-Lxcm5*Lycm5*dQ1*dQ4*m5*t2*t4*t7*t10*2.0-Lxcm5*Lycm5*dQ1*dQ5*m5*t2*t5*t7*t9*2.0-Lxcm5*Lycm5*dQ2*dQ3*m5*t2*t4*t8*t10*2.0-Lxcm5*Lycm5*dQ2*dQ3*m5*t3*t4*t7*t10*2.0-Lxcm5*Lycm5*dQ1*dQ4*m5*t3*t4*t8*t10*2.0+Lxcm6*Lycm6*dQ1*dQ6*m6*t2*t3*t7*t8*8.0-Lxcm5*Lycm5*dQ1*dQ5*m5*t3*t5*t8*t9*2.0-Lxcm5*Lycm5*dQ2*dQ5*m5*t4*t5*t7*t8*2.0+Lxcm6*Lycm6*dQ1*dQ4*m6*t2*t4*t7*t10*2.0-Lxcm5*Lycm5*dQ3*dQ5*m5*t4*t5*t7*t8*2.0+Lxcm6*Lycm6*dQ1*dQ2*m6*t2*t6*t7*t11*8.0+Lxcm6*Lycm6*dQ1*dQ5*m6*t2*t5*t7*t9*2.0;
et149 = Lxcm6*Lycm6*dQ2*dQ3*m6*t2*t4*t8*t10*2.0+Lxcm6*Lycm6*dQ2*dQ3*m6*t3*t4*t7*t10*2.0+Lxcm6*Lycm6*dQ1*dQ3*m6*t2*t6*t7*t11*8.0+Lxcm6*Lycm6*dQ1*dQ4*m6*t3*t4*t8*t10*2.0+Lxcm6*Lycm6*dQ1*dQ2*m6*t3*t6*t8*t11*8.0+Lxcm6*Lycm6*dQ1*dQ5*m6*t3*t5*t8*t9*2.0+Lxcm6*Lycm6*dQ2*dQ5*m6*t4*t5*t7*t8*2.0+Lxcm6*Lycm6*dQ2*dQ6*m6*t2*t4*t8*t9*2.0+Lxcm6*Lycm6*dQ2*dQ6*m6*t3*t4*t7*t9*2.0+Lxcm6*Lycm6*dQ1*dQ3*m6*t3*t6*t8*t11*8.0+Lxcm6*Lycm6*dQ3*dQ5*m6*t4*t5*t7*t8*2.0+Lxcm6*Lycm6*dQ3*dQ6*m6*t2*t4*t8*t9*2.0+Lxcm6*Lycm6*dQ3*dQ6*m6*t3*t4*t7*t9*2.0+Lxcm6*Lycm6*dQ1*dQ5*m6*t5*t6*t10*t11*4.0+Lxcm5*Lycm5*dQ2*dQ3*m5*t2*t3*t5*t34*4.0-Lxcm6*Lycm6*dQ2*dQ3*m6*t2*t3*t5*t34*4.0-Lxcm6*Lycm6*dQ2*dQ3*m6*t2*t3*t5*t36*4.0;
et150 = Lxcm5*Lycm5*dQ2*dQ3*m5*t5*t7*t8*t34*-4.0-Lxcm5*Lycm5*dQ1*dQ5*m5*t4*t9*t10*t32*2.0-Lxcm5*Lycm5*dQ2*dQ5*m5*t2*t8*t10*t34*2.0-Lxcm5*Lycm5*dQ2*dQ5*m5*t3*t7*t10*t34*2.0-Lxcm5*Lycm5*dQ1*dQ5*m5*t4*t9*t10*t33*2.0-Lxcm5*Lycm5*dQ3*dQ5*m5*t2*t8*t10*t34*2.0-Lxcm5*Lycm5*dQ3*dQ5*m5*t3*t7*t10*t34*2.0+Lxcm6*Lycm6*dQ2*dQ3*m6*t5*t7*t8*t34*4.0+Lxcm6*Lycm6*dQ1*dQ5*m6*t4*t9*t10*t32*2.0+Lxcm6*Lycm6*dQ2*dQ3*m6*t5*t7*t8*t36*4.0+Lxcm6*Lycm6*dQ2*dQ5*m6*t2*t8*t10*t34*2.0+Lxcm6*Lycm6*dQ2*dQ5*m6*t3*t7*t10*t34*2.0+Lxcm6*Lycm6*dQ1*dQ5*m6*t4*t9*t10*t33*2.0+Lxcm6*Lycm6*dQ3*dQ5*m6*t2*t8*t10*t34*2.0+Lxcm6*Lycm6*dQ3*dQ5*m6*t3*t7*t10*t34*2.0-Lxcm6*Lycm6*dQ5*dQ6*m6*t2*t8*t9*t36*4.0-Lxcm6*Lycm6*dQ5*dQ6*m6*t3*t7*t9*t36*4.0;
et151 = Lxcm5*Lycm5*dQ1*dQ2*m5*t9*t10*t32*t33*8.0+Lxcm5*Lycm5*dQ1*dQ3*m5*t9*t10*t32*t33*8.0-Lxcm6*Lycm6*dQ4*dQ6*m6*t2*t3*t35*t36*4.0-Lxcm6*Lycm6*dQ1*dQ2*m6*t9*t10*t32*t33*8.0-Lxcm6*Lycm6*dQ1*dQ3*m6*t9*t10*t32*t33*8.0-Lxcm6*Lycm6*dQ1*dQ2*m6*t9*t10*t32*t36*8.0-Lxcm6*Lycm6*dQ1*dQ2*m6*t9*t10*t33*t36*8.0-Lxcm6*Lycm6*dQ1*dQ3*m6*t9*t10*t32*t36*8.0-Lxcm6*Lycm6*dQ1*dQ3*m6*t9*t10*t33*t36*8.0+Lxcm6*Lycm6*dQ4*dQ6*m6*t7*t8*t35*t36*4.0-Lxcm5*Lycm5*dQ1*dQ4*m5*t5*t32*t33*t34*8.0+Lxcm6*Lycm6*dQ1*dQ4*m6*t5*t32*t33*t34*8.0+Lxcm6*Lycm6*dQ1*dQ4*m6*t5*t32*t33*t36*8.0+Lxcm6*Lycm6*dQ1*dQ4*m6*t5*t32*t34*t36*8.0+Lxcm6*Lycm6*dQ1*dQ4*m6*t5*t33*t34*t36*8.0+Lxcm6*Lycm6*dQ1*dQ6*m6*t32*t33*t34*t35*4.0;
et152 = Lxcm6*Lycm6*dQ1*dQ6*m6*t32*t33*t34*t36*-8.0-Lxcm6*Lycm6*dQ1*dQ6*m6*t32*t33*t35*t36*8.0+Lxcm6*Lycm6*dQ1*dQ6*m6*t32*t34*t35*t36*4.0+Lxcm6*Lycm6*dQ1*dQ6*m6*t33*t34*t35*t36*4.0+Lx3*Lz6*dQ4*dQ5*m6*t2*t3*t4*t5*2.0-Lx2*Lz6*dQ1*dQ2*m6*t2*t5*t7*t8*4.0-Lx2*Lz6*dQ1*dQ3*m6*t2*t5*t7*t8*2.0+Lx3*Lz6*dQ1*dQ2*m6*t2*t4*t7*t10*4.0-Lx2*Lz6*dQ1*dQ5*m6*t2*t3*t7*t10*2.0+Lx3*Lz6*dQ1*dQ3*m6*t2*t4*t7*t10*4.0+Lx3*Lz6*dQ1*dQ2*m6*t3*t4*t8*t10*4.0+Lx3*Lz6*dQ1*dQ3*m6*t3*t4*t8*t10*4.0+Lx3*Lz6*dQ2*dQ3*m6*t2*t3*t9*t10*2.0+Lx4*Lz6*dQ1*dQ4*m6*t2*t5*t7*t9*2.0+Lx4*Lz6*dQ1*dQ5*m6*t2*t4*t7*t10*2.0+Lx4*Lz6*dQ2*dQ3*m6*t2*t5*t8*t9*2.0+Lx4*Lz6*dQ2*dQ3*m6*t3*t5*t7*t9*2.0;
et153 = Lx4*Lz6*dQ1*dQ4*m6*t3*t5*t8*t9*2.0+Lx4*Lz6*dQ1*dQ5*m6*t3*t4*t8*t10*2.0+Lx4*Lz6*dQ2*dQ5*m6*t2*t3*t9*t10*2.0-Lx3*Lz6*dQ4*dQ5*m6*t4*t5*t7*t8*2.0+Lx4*Lz6*dQ3*dQ5*m6*t2*t3*t9*t10*2.0-Lx3*Lz6*dQ2*dQ3*m6*t7*t8*t9*t10*2.0-Lx4*Lz6*dQ2*dQ5*m6*t7*t8*t9*t10*2.0-Lx4*Lz6*dQ3*dQ5*m6*t7*t8*t9*t10*2.0+Lx2*Lz6*dQ1*dQ5*m6*t3*t4*t5*t32*2.0-Lx2*Lz6*dQ1*dQ2*m6*t4*t8*t10*t32*4.0-Lx2*Lz6*dQ1*dQ3*m6*t4*t8*t10*t32*2.0+Lx4*Lz6*dQ1*dQ2*m6*t2*t7*t10*t34*4.0-Lx2*Lz6*dQ1*dQ4*m6*t3*t9*t10*t32*2.0-Lx3*Lz6*dQ1*dQ5*m6*t2*t7*t10*t33*4.0+Lx4*Lz6*dQ1*dQ3*m6*t2*t7*t10*t34*4.0-Lx3*Lz6*dQ1*dQ5*m6*t3*t8*t10*t32*4.0+Lx4*Lz6*dQ1*dQ2*m6*t3*t8*t10*t34*4.0;
et154 = Lx4*Lz6*dQ1*dQ3*m6*t3*t8*t10*t34*4.0+Lx4*Lz6*dQ1*dQ4*m6*t4*t9*t10*t32*4.0+Lx4*Lz6*dQ2*dQ4*m6*t2*t8*t10*t34*4.0+Lx4*Lz6*dQ2*dQ4*m6*t3*t7*t10*t34*4.0+Lx4*Lz6*dQ1*dQ4*m6*t4*t9*t10*t33*4.0+Lx4*Lz6*dQ3*dQ4*m6*t2*t8*t10*t34*4.0+Lx4*Lz6*dQ3*dQ4*m6*t3*t7*t10*t34*4.0+Lx4*Lz6*dQ1*dQ2*m6*t4*t5*t32*t33*8.0+Lx4*Lz6*dQ1*dQ3*m6*t4*t5*t32*t33*8.0+Lx3*Lz6*dQ1*dQ5*m6*t4*t5*t32*t33*4.0-Lx3*Lz6*dQ1*dQ4*m6*t9*t10*t32*t33*4.0+Lx4*Lz6*dQ1*dQ5*m6*t5*t32*t33*t34*4.0-Lx3*Lzcm3*dQ1*dQ2*m3*t2*t3*t7*t8*8.0-Lx3*Lzcm3*dQ1*dQ3*m3*t2*t3*t7*t8*8.0-Lx3*Lzcm4*dQ1*dQ2*m4*t2*t3*t7*t8*8.0-Lx3*Lzcm4*dQ1*dQ3*m4*t2*t3*t7*t8*8.0+Lx3*Lzcm5*dQ4*dQ5*m5*t2*t3*t4*t5*2.0;
et155 = Lx2*Lzcm5*dQ1*dQ2*m5*t2*t5*t7*t8*-4.0-Lx2*Lzcm5*dQ1*dQ3*m5*t2*t5*t7*t8*2.0+Lx3*Lzcm6*dQ4*dQ5*m6*t2*t3*t4*t5*2.0-Lx2*Lzcm6*dQ1*dQ2*m6*t2*t5*t7*t8*4.0+Lx3*Lzcm5*dQ1*dQ2*m5*t2*t4*t7*t10*4.0-Lx2*Lzcm5*dQ1*dQ5*m5*t2*t3*t7*t10*2.0-Lx2*Lzcm6*dQ1*dQ3*m6*t2*t5*t7*t8*2.0+Lx3*Lzcm5*dQ1*dQ3*m5*t2*t4*t7*t10*4.0+Lx3*Lzcm5*dQ1*dQ2*m5*t3*t4*t8*t10*4.0+Lx3*Lzcm6*dQ1*dQ2*m6*t2*t4*t7*t10*4.0-Lx2*Lzcm6*dQ1*dQ5*m6*t2*t3*t7*t10*2.0+Lx3*Lzcm5*dQ1*dQ3*m5*t3*t4*t8*t10*4.0+Lx3*Lzcm5*dQ2*dQ3*m5*t2*t3*t9*t10*2.0+Lx3*Lzcm6*dQ1*dQ3*m6*t2*t4*t7*t10*4.0+Lx4*Lzcm5*dQ1*dQ4*m5*t2*t5*t7*t9*2.0+Lx3*Lzcm6*dQ1*dQ2*m6*t3*t4*t8*t10*4.0+Lx4*Lzcm5*dQ1*dQ5*m5*t2*t4*t7*t10*2.0;
et156 = Lx4*Lzcm5*dQ2*dQ3*m5*t2*t5*t8*t9*2.0+Lx4*Lzcm5*dQ2*dQ3*m5*t3*t5*t7*t9*2.0+Lx3*Lzcm6*dQ1*dQ3*m6*t3*t4*t8*t10*4.0+Lx3*Lzcm6*dQ2*dQ3*m6*t2*t3*t9*t10*2.0+Lx4*Lzcm5*dQ1*dQ4*m5*t3*t5*t8*t9*2.0+Lx4*Lzcm6*dQ1*dQ4*m6*t2*t5*t7*t9*2.0+Lx4*Lzcm5*dQ1*dQ5*m5*t3*t4*t8*t10*2.0+Lx4*Lzcm5*dQ2*dQ5*m5*t2*t3*t9*t10*2.0+Lx4*Lzcm6*dQ1*dQ5*m6*t2*t4*t7*t10*2.0+Lx4*Lzcm6*dQ2*dQ3*m6*t2*t5*t8*t9*2.0+Lx4*Lzcm6*dQ2*dQ3*m6*t3*t5*t7*t9*2.0-Lx3*Lzcm5*dQ4*dQ5*m5*t4*t5*t7*t8*2.0+Lx4*Lzcm5*dQ3*dQ5*m5*t2*t3*t9*t10*2.0+Lx4*Lzcm6*dQ1*dQ4*m6*t3*t5*t8*t9*2.0+Lx4*Lzcm6*dQ1*dQ5*m6*t3*t4*t8*t10*2.0+Lx4*Lzcm6*dQ2*dQ5*m6*t2*t3*t9*t10*2.0-Lxcm6*Lz6*dQ1*dQ4*m6*t2*t6*t7*t9*2.0;
et157 = Lx3*Lzcm6*dQ4*dQ5*m6*t4*t5*t7*t8*-2.0+Lx4*Lzcm6*dQ3*dQ5*m6*t2*t3*t9*t10*2.0-Lxcm6*Lz6*dQ2*dQ3*m6*t2*t6*t8*t9*2.0-Lxcm6*Lz6*dQ2*dQ3*m6*t3*t6*t7*t9*2.0-Lxcm6*Lz6*dQ1*dQ4*m6*t3*t6*t8*t9*2.0-Lxcm6*Lz6*dQ1*dQ6*m6*t2*t4*t7*t11*2.0-Lxcm6*Lz6*dQ2*dQ3*m6*t2*t3*t10*t11*2.0-Lxcm6*Lz6*dQ1*dQ6*m6*t3*t4*t8*t11*2.0-Lxcm6*Lz6*dQ2*dQ6*m6*t2*t3*t9*t11*2.0-Lx3*Lzcm5*dQ2*dQ3*m5*t7*t8*t9*t10*2.0-Lxcm6*Lz6*dQ2*dQ6*m6*t2*t6*t8*t10*2.0-Lxcm6*Lz6*dQ2*dQ6*m6*t3*t6*t7*t10*2.0-Lxcm6*Lz6*dQ3*dQ6*m6*t2*t3*t9*t11*2.0-Lxcm6*Lz6*dQ3*dQ6*m6*t2*t6*t8*t10*2.0-Lxcm6*Lz6*dQ3*dQ6*m6*t3*t6*t7*t10*2.0-Lx3*Lzcm6*dQ2*dQ3*m6*t7*t8*t9*t10*2.0;
et158 = Lx4*Lzcm5*dQ2*dQ5*m5*t7*t8*t9*t10*-2.0-Lx4*Lzcm5*dQ3*dQ5*m5*t7*t8*t9*t10*2.0-Lx4*Lzcm6*dQ2*dQ5*m6*t7*t8*t9*t10*2.0-Lx4*Lzcm6*dQ3*dQ5*m6*t7*t8*t9*t10*2.0+Lxcm6*Lz6*dQ2*dQ3*m6*t7*t8*t10*t11*2.0+Lxcm6*Lz6*dQ2*dQ6*m6*t7*t8*t9*t11*2.0+Lx2*Lzcm5*dQ1*dQ5*m5*t3*t4*t5*t32*2.0+Lxcm6*Lz6*dQ3*dQ6*m6*t7*t8*t9*t11*2.0+Lx2*Lzcm6*dQ1*dQ5*m6*t3*t4*t5*t32*2.0-Lx4*Lzcm4*dQ1*dQ4*m4*t2*t7*t9*t33*4.0-Lx2*Lzcm5*dQ1*dQ2*m5*t4*t8*t10*t32*4.0-Lx4*Lzcm4*dQ1*dQ4*m4*t3*t8*t9*t32*4.0-Lx2*Lzcm5*dQ1*dQ3*m5*t4*t8*t10*t32*2.0+Lx4*Lzcm5*dQ1*dQ2*m5*t2*t7*t10*t34*4.0-Lx2*Lzcm5*dQ1*dQ4*m5*t3*t9*t10*t32*2.0-Lx2*Lzcm6*dQ1*dQ2*m6*t4*t8*t10*t32*4.0-Lx3*Lzcm5*dQ1*dQ5*m5*t2*t7*t10*t33*4.0;
et159 = Lx4*Lzcm5*dQ1*dQ3*m5*t2*t7*t10*t34*4.0-Lx2*Lzcm6*dQ1*dQ3*m6*t4*t8*t10*t32*2.0-Lx3*Lzcm5*dQ1*dQ5*m5*t3*t8*t10*t32*4.0+Lx4*Lzcm5*dQ1*dQ2*m5*t3*t8*t10*t34*4.0+Lx4*Lzcm6*dQ1*dQ2*m6*t2*t7*t10*t34*4.0-Lx2*Lzcm6*dQ1*dQ4*m6*t3*t9*t10*t32*2.0-Lx3*Lzcm6*dQ1*dQ5*m6*t2*t7*t10*t33*4.0+Lx4*Lzcm5*dQ1*dQ3*m5*t3*t8*t10*t34*4.0+Lx4*Lzcm6*dQ1*dQ3*m6*t2*t7*t10*t34*4.0+Lxcm6*Lz6*dQ4*dQ5*m6*t2*t3*t6*t35*4.0-Lx3*Lzcm6*dQ1*dQ5*m6*t3*t8*t10*t32*4.0+Lx4*Lzcm5*dQ1*dQ4*m5*t4*t9*t10*t32*4.0+Lx4*Lzcm5*dQ2*dQ4*m5*t2*t8*t10*t34*4.0+Lx4*Lzcm5*dQ2*dQ4*m5*t3*t7*t10*t34*4.0+Lx4*Lzcm6*dQ1*dQ2*m6*t3*t8*t10*t34*4.0+Lx4*Lzcm5*dQ1*dQ4*m5*t4*t9*t10*t33*4.0+Lx4*Lzcm5*dQ3*dQ4*m5*t2*t8*t10*t34*4.0;
et160 = Lx4*Lzcm5*dQ3*dQ4*m5*t3*t7*t10*t34*4.0+Lx4*Lzcm6*dQ1*dQ3*m6*t3*t8*t10*t34*4.0+Lx4*Lzcm6*dQ1*dQ4*m6*t4*t9*t10*t32*4.0+Lx4*Lzcm6*dQ2*dQ4*m6*t2*t8*t10*t34*4.0+Lx4*Lzcm6*dQ2*dQ4*m6*t3*t7*t10*t34*4.0+Lx4*Lzcm6*dQ1*dQ4*m6*t4*t9*t10*t33*4.0+Lx4*Lzcm6*dQ3*dQ4*m6*t2*t8*t10*t34*4.0+Lx4*Lzcm6*dQ3*dQ4*m6*t3*t7*t10*t34*4.0+Lxcm6*Lz6*dQ1*dQ2*m6*t5*t9*t11*t32*4.0+Lxcm6*Lz6*dQ1*dQ2*m6*t5*t9*t11*t33*4.0+Lxcm6*Lz6*dQ1*dQ3*m6*t5*t9*t11*t32*4.0+Lxcm6*Lz6*dQ1*dQ3*m6*t5*t9*t11*t33*4.0+Lxcm6*Lz6*dQ1*dQ6*m6*t5*t10*t11*t32*2.0-Lxcm6*Lz6*dQ4*dQ5*m6*t6*t7*t8*t35*4.0+Lxcm6*Lz6*dQ1*dQ6*m6*t5*t10*t11*t33*2.0+Lx4*Lzcm5*dQ1*dQ2*m5*t4*t5*t32*t33*8.0+Lx4*Lzcm5*dQ1*dQ3*m5*t4*t5*t32*t33*8.0;
et161 = Lx3*Lzcm5*dQ1*dQ5*m5*t4*t5*t32*t33*4.0+Lx4*Lzcm6*dQ1*dQ2*m6*t4*t5*t32*t33*8.0+Lx4*Lzcm6*dQ1*dQ3*m6*t4*t5*t32*t33*8.0+Lx3*Lzcm6*dQ1*dQ5*m6*t4*t5*t32*t33*4.0-Lxcm6*Lz6*dQ1*dQ2*m6*t4*t6*t32*t33*8.0-Lxcm6*Lz6*dQ1*dQ3*m6*t4*t6*t32*t33*8.0-Lxcm6*Lz6*dQ1*dQ2*m6*t4*t6*t32*t35*8.0-Lxcm6*Lz6*dQ1*dQ2*m6*t4*t6*t33*t35*8.0-Lxcm6*Lz6*dQ1*dQ3*m6*t4*t6*t32*t35*8.0-Lxcm6*Lz6*dQ1*dQ3*m6*t4*t6*t33*t35*8.0-Lx3*Lzcm5*dQ1*dQ4*m5*t9*t10*t32*t33*4.0-Lx3*Lzcm6*dQ1*dQ4*m6*t9*t10*t32*t33*4.0+Lxcm6*Lz6*dQ1*dQ4*m6*t10*t11*t32*t33*4.0+Lxcm6*Lz6*dQ1*dQ4*m6*t10*t11*t32*t34*4.0+Lxcm6*Lz6*dQ1*dQ4*m6*t10*t11*t33*t34*4.0+Lx4*Lzcm5*dQ1*dQ5*m5*t5*t32*t33*t34*4.0;
et162 = Lx4*Lzcm6*dQ1*dQ5*m6*t5*t32*t33*t34*4.0-Lxcm6*Lz6*dQ1*dQ5*m6*t6*t32*t33*t34*4.0+Lxcm6*Lz6*dQ1*dQ5*m6*t6*t32*t33*t35*8.0-Lxcm6*Lz6*dQ1*dQ5*m6*t6*t32*t34*t35*4.0-Lxcm6*Lz6*dQ1*dQ5*m6*t6*t33*t34*t35*4.0-Lxcm3*Lzcm3*dQ1*dQ2*m3*t2*t3*t7*t8*8.0-Lxcm3*Lzcm3*dQ1*dQ3*m3*t2*t3*t7*t8*8.0+Lxcm5*Lzcm5*dQ1*dQ5*m5*t2*t3*t7*t8*4.0+Lxcm5*Lzcm5*dQ1*dQ2*m5*t2*t5*t7*t10*4.0+Lxcm5*Lzcm5*dQ1*dQ3*m5*t2*t5*t7*t10*4.0+Lxcm5*Lzcm5*dQ1*dQ2*m5*t3*t5*t8*t10*4.0+Lxcm5*Lzcm5*dQ1*dQ3*m5*t3*t5*t8*t10*4.0-Lxcm5*Lzcm5*dQ2*dQ5*m5*t2*t4*t8*t9*2.0-Lxcm5*Lzcm5*dQ2*dQ5*m5*t3*t4*t7*t9*2.0-Lxcm5*Lzcm5*dQ2*dQ4*m5*t2*t5*t8*t10*4.0-Lxcm5*Lzcm5*dQ2*dQ4*m5*t3*t5*t7*t10*4.0-Lxcm5*Lzcm5*dQ3*dQ5*m5*t2*t4*t8*t9*2.0;
et163 = Lxcm5*Lzcm5*dQ3*dQ5*m5*t3*t4*t7*t9*-2.0-Lxcm5*Lzcm5*dQ3*dQ4*m5*t2*t5*t8*t10*4.0-Lxcm5*Lzcm5*dQ3*dQ4*m5*t3*t5*t7*t10*4.0-Lxcm6*Lzcm6*dQ1*dQ4*m6*t2*t6*t7*t9*2.0-Lxcm6*Lzcm6*dQ2*dQ3*m6*t2*t6*t8*t9*2.0-Lxcm6*Lzcm6*dQ2*dQ3*m6*t3*t6*t7*t9*2.0-Lxcm6*Lzcm6*dQ1*dQ4*m6*t3*t6*t8*t9*2.0-Lxcm6*Lzcm6*dQ1*dQ6*m6*t2*t4*t7*t11*2.0-Lxcm6*Lzcm6*dQ2*dQ3*m6*t2*t3*t10*t11*2.0-Lxcm6*Lzcm6*dQ1*dQ6*m6*t3*t4*t8*t11*2.0-Lxcm6*Lzcm6*dQ2*dQ6*m6*t2*t3*t9*t11*2.0-Lxcm6*Lzcm6*dQ2*dQ6*m6*t2*t6*t8*t10*2.0-Lxcm6*Lzcm6*dQ2*dQ6*m6*t3*t6*t7*t10*2.0-Lxcm6*Lzcm6*dQ3*dQ6*m6*t2*t3*t9*t11*2.0-Lxcm6*Lzcm6*dQ3*dQ6*m6*t2*t6*t8*t10*2.0-Lxcm6*Lzcm6*dQ3*dQ6*m6*t3*t6*t7*t10*2.0;
et164 = Lxcm6*Lzcm6*dQ2*dQ3*m6*t7*t8*t10*t11*2.0+Lxcm6*Lzcm6*dQ2*dQ6*m6*t7*t8*t9*t11*2.0+Lxcm6*Lzcm6*dQ3*dQ6*m6*t7*t8*t9*t11*2.0-Lxcm4*Lzcm4*dQ1*dQ4*m4*t2*t7*t9*t33*4.0-Lxcm4*Lzcm4*dQ1*dQ4*m4*t3*t8*t9*t32*4.0+Lxcm5*Lzcm5*dQ1*dQ4*m5*t2*t7*t9*t33*4.0+Lxcm5*Lzcm5*dQ1*dQ4*m5*t3*t8*t9*t32*4.0+Lxcm5*Lzcm5*dQ1*dQ4*m5*t2*t7*t9*t35*4.0+Lxcm6*Lzcm6*dQ4*dQ5*m6*t2*t3*t6*t35*4.0+Lxcm5*Lzcm5*dQ2*dQ3*m5*t2*t8*t9*t35*4.0+Lxcm5*Lzcm5*dQ2*dQ3*m5*t3*t7*t9*t35*4.0+Lxcm5*Lzcm5*dQ1*dQ4*m5*t3*t8*t9*t35*4.0+Lxcm6*Lzcm6*dQ1*dQ2*m6*t5*t9*t11*t32*4.0+Lxcm6*Lzcm6*dQ1*dQ2*m6*t5*t9*t11*t33*4.0+Lxcm6*Lzcm6*dQ1*dQ3*m6*t5*t9*t11*t32*4.0+Lxcm6*Lzcm6*dQ1*dQ3*m6*t5*t9*t11*t33*4.0+Lxcm6*Lzcm6*dQ1*dQ6*m6*t5*t10*t11*t32*2.0;
et165 = Lxcm6*Lzcm6*dQ4*dQ5*m6*t6*t7*t8*t35*-4.0+Lxcm6*Lzcm6*dQ1*dQ6*m6*t5*t10*t11*t33*2.0-Lxcm6*Lzcm6*dQ1*dQ2*m6*t4*t6*t32*t33*8.0-Lxcm6*Lzcm6*dQ1*dQ3*m6*t4*t6*t32*t33*8.0-Lxcm6*Lzcm6*dQ1*dQ2*m6*t4*t6*t32*t35*8.0-Lxcm6*Lzcm6*dQ1*dQ2*m6*t4*t6*t33*t35*8.0-Lxcm6*Lzcm6*dQ1*dQ3*m6*t4*t6*t32*t35*8.0-Lxcm6*Lzcm6*dQ1*dQ3*m6*t4*t6*t33*t35*8.0+Lxcm6*Lzcm6*dQ1*dQ4*m6*t10*t11*t32*t33*4.0+Lxcm6*Lzcm6*dQ1*dQ4*m6*t10*t11*t32*t34*4.0+Lxcm6*Lzcm6*dQ1*dQ4*m6*t10*t11*t33*t34*4.0+Lxcm5*Lzcm5*dQ1*dQ2*m5*t4*t32*t33*t35*1.6e+1+Lxcm5*Lzcm5*dQ1*dQ3*m5*t4*t32*t33*t35*1.6e+1-Lxcm6*Lzcm6*dQ1*dQ5*m6*t6*t32*t33*t34*4.0+Lxcm6*Lzcm6*dQ1*dQ5*m6*t6*t32*t33*t35*8.0-Lxcm6*Lzcm6*dQ1*dQ5*m6*t6*t32*t34*t35*4.0;
et166 = Lxcm6*Lzcm6*dQ1*dQ5*m6*t6*t33*t34*t35*-4.0+Lxcm5*Lzcm5*dQ1*dQ5*m5*t32*t33*t34*t35*8.0-Lycm6*Lz6*dQ1*dQ6*m6*t2*t4*t6*t7*2.0-Lycm6*Lz6*dQ2*dQ3*m6*t2*t3*t6*t10*2.0-Lycm6*Lz6*dQ1*dQ6*m6*t3*t4*t6*t8*2.0-Lycm6*Lz6*dQ2*dQ6*m6*t2*t3*t6*t9*2.0-Lycm6*Lz6*dQ3*dQ6*m6*t2*t3*t6*t9*2.0+Lycm6*Lz6*dQ1*dQ4*m6*t2*t7*t9*t11*2.0+Lycm6*Lz6*dQ2*dQ3*m6*t2*t8*t9*t11*2.0+Lycm6*Lz6*dQ2*dQ3*m6*t3*t7*t9*t11*2.0+Lycm6*Lz6*dQ1*dQ4*m6*t3*t8*t9*t11*2.0+Lycm6*Lz6*dQ2*dQ3*m6*t6*t7*t8*t10*2.0+Lycm6*Lz6*dQ2*dQ6*m6*t6*t7*t8*t9*2.0+Lycm6*Lz6*dQ2*dQ6*m6*t2*t8*t10*t11*2.0+Lycm6*Lz6*dQ2*dQ6*m6*t3*t7*t10*t11*2.0+Lycm6*Lz6*dQ3*dQ6*m6*t6*t7*t8*t9*2.0+Lycm6*Lz6*dQ3*dQ6*m6*t2*t8*t10*t11*2.0;
et167 = Lycm6*Lz6*dQ3*dQ6*m6*t3*t7*t10*t11*2.0+Lycm6*Lz6*dQ1*dQ2*m6*t5*t6*t9*t32*4.0+Lycm6*Lz6*dQ1*dQ2*m6*t5*t6*t9*t33*4.0+Lycm6*Lz6*dQ1*dQ3*m6*t5*t6*t9*t32*4.0+Lycm6*Lz6*dQ1*dQ3*m6*t5*t6*t9*t33*4.0+Lycm6*Lz6*dQ1*dQ6*m6*t5*t6*t10*t32*2.0-Lycm6*Lz6*dQ4*dQ5*m6*t2*t3*t11*t35*4.0+Lycm6*Lz6*dQ1*dQ6*m6*t5*t6*t10*t33*2.0+Lycm6*Lz6*dQ4*dQ5*m6*t7*t8*t11*t35*4.0+Lycm6*Lz6*dQ1*dQ2*m6*t4*t11*t32*t33*8.0+Lycm6*Lz6*dQ1*dQ3*m6*t4*t11*t32*t33*8.0+Lycm6*Lz6*dQ1*dQ2*m6*t4*t11*t32*t35*8.0+Lycm6*Lz6*dQ1*dQ2*m6*t4*t11*t33*t35*8.0+Lycm6*Lz6*dQ1*dQ3*m6*t4*t11*t32*t35*8.0+Lycm6*Lz6*dQ1*dQ4*m6*t6*t10*t32*t33*4.0+Lycm6*Lz6*dQ1*dQ3*m6*t4*t11*t33*t35*8.0+Lycm6*Lz6*dQ1*dQ4*m6*t6*t10*t32*t34*4.0;
et168 = Lycm6*Lz6*dQ1*dQ4*m6*t6*t10*t33*t34*4.0+Lycm6*Lz6*dQ1*dQ5*m6*t11*t32*t33*t34*4.0-Lycm6*Lz6*dQ1*dQ5*m6*t11*t32*t33*t35*8.0+Lycm6*Lz6*dQ1*dQ5*m6*t11*t32*t34*t35*4.0+Lycm6*Lz6*dQ1*dQ5*m6*t11*t33*t34*t35*4.0+Lycm5*Lzcm5*dQ1*dQ4*m5*t2*t4*t5*t7*2.0+Lycm5*Lzcm5*dQ2*dQ3*m5*t2*t4*t5*t8*2.0+Lycm5*Lzcm5*dQ2*dQ3*m5*t3*t4*t5*t7*2.0+Lycm5*Lzcm5*dQ1*dQ4*m5*t3*t4*t5*t8*2.0+Lycm5*Lzcm5*dQ2*dQ5*m5*t2*t3*t4*t10*2.0+Lycm5*Lzcm5*dQ3*dQ5*m5*t2*t3*t4*t10*2.0-Lycm6*Lzcm6*dQ1*dQ6*m6*t2*t4*t6*t7*2.0-Lycm6*Lzcm6*dQ2*dQ3*m6*t2*t3*t6*t10*2.0-Lycm6*Lzcm6*dQ1*dQ6*m6*t3*t4*t6*t8*2.0-Lycm6*Lzcm6*dQ2*dQ6*m6*t2*t3*t6*t9*2.0-Lycm6*Lzcm6*dQ3*dQ6*m6*t2*t3*t6*t9*2.0-Lycm5*Lzcm5*dQ1*dQ5*m5*t2*t7*t9*t10*2.0;
et169 = Lycm5*Lzcm5*dQ1*dQ5*m5*t3*t8*t9*t10*-2.0-Lycm5*Lzcm5*dQ2*dQ5*m5*t4*t7*t8*t10*2.0-Lycm5*Lzcm5*dQ3*dQ5*m5*t4*t7*t8*t10*2.0+Lycm6*Lzcm6*dQ1*dQ4*m6*t2*t7*t9*t11*2.0+Lycm6*Lzcm6*dQ2*dQ3*m6*t2*t8*t9*t11*2.0+Lycm6*Lzcm6*dQ2*dQ3*m6*t3*t7*t9*t11*2.0+Lycm6*Lzcm6*dQ1*dQ4*m6*t3*t8*t9*t11*2.0+Lycm6*Lzcm6*dQ2*dQ3*m6*t6*t7*t8*t10*2.0+Lycm6*Lzcm6*dQ2*dQ6*m6*t6*t7*t8*t9*2.0+Lycm6*Lzcm6*dQ2*dQ6*m6*t2*t8*t10*t11*2.0+Lycm6*Lzcm6*dQ2*dQ6*m6*t3*t7*t10*t11*2.0+Lycm6*Lzcm6*dQ3*dQ6*m6*t6*t7*t8*t9*2.0+Lycm6*Lzcm6*dQ3*dQ6*m6*t2*t8*t10*t11*2.0+Lycm6*Lzcm6*dQ3*dQ6*m6*t3*t7*t10*t11*2.0-Lycm4*Lzcm4*dQ1*dQ4*m4*t2*t4*t7*t33*4.0-Lycm4*Lzcm4*dQ1*dQ4*m4*t3*t4*t8*t32*4.0+Lycm5*Lzcm5*dQ2*dQ3*m5*t2*t3*t10*t34*4.0;
et170 = Lycm5*Lzcm5*dQ1*dQ5*m5*t4*t5*t9*t32*2.0+Lycm5*Lzcm5*dQ2*dQ5*m5*t2*t5*t8*t34*2.0+Lycm5*Lzcm5*dQ2*dQ5*m5*t3*t5*t7*t34*2.0+Lycm5*Lzcm5*dQ1*dQ5*m5*t4*t5*t9*t33*2.0+Lycm5*Lzcm5*dQ3*dQ5*m5*t2*t5*t8*t34*2.0+Lycm5*Lzcm5*dQ3*dQ5*m5*t3*t5*t7*t34*2.0+Lycm6*Lzcm6*dQ1*dQ2*m6*t5*t6*t9*t32*4.0+Lycm6*Lzcm6*dQ1*dQ2*m6*t5*t6*t9*t33*4.0+Lycm6*Lzcm6*dQ1*dQ3*m6*t5*t6*t9*t32*4.0+Lycm6*Lzcm6*dQ1*dQ3*m6*t5*t6*t9*t33*4.0+Lycm6*Lzcm6*dQ1*dQ6*m6*t5*t6*t10*t32*2.0-Lycm6*Lzcm6*dQ4*dQ5*m6*t2*t3*t11*t35*4.0-Lycm5*Lzcm5*dQ2*dQ3*m5*t7*t8*t10*t34*4.0+Lycm6*Lzcm6*dQ1*dQ6*m6*t5*t6*t10*t33*2.0+Lycm6*Lzcm6*dQ4*dQ5*m6*t7*t8*t11*t35*4.0-Lycm5*Lzcm5*dQ1*dQ2*m5*t5*t9*t32*t33*8.0-Lycm5*Lzcm5*dQ1*dQ3*m5*t5*t9*t32*t33*8.0;
et171 = Lycm6*Lzcm6*dQ1*dQ2*m6*t4*t11*t32*t33*8.0+Lycm6*Lzcm6*dQ1*dQ3*m6*t4*t11*t32*t33*8.0+Lycm6*Lzcm6*dQ1*dQ2*m6*t4*t11*t32*t35*8.0+Lycm6*Lzcm6*dQ1*dQ2*m6*t4*t11*t33*t35*8.0+Lycm6*Lzcm6*dQ1*dQ3*m6*t4*t11*t32*t35*8.0+Lycm6*Lzcm6*dQ1*dQ4*m6*t6*t10*t32*t33*4.0+Lycm6*Lzcm6*dQ1*dQ3*m6*t4*t11*t33*t35*8.0+Lycm6*Lzcm6*dQ1*dQ4*m6*t6*t10*t32*t34*4.0+Lycm6*Lzcm6*dQ1*dQ4*m6*t6*t10*t33*t34*4.0-Lycm5*Lzcm5*dQ1*dQ4*m5*t10*t32*t33*t34*8.0+Lycm6*Lzcm6*dQ1*dQ5*m6*t11*t32*t33*t34*4.0-Lycm6*Lzcm6*dQ1*dQ5*m6*t11*t32*t33*t35*8.0+Lycm6*Lzcm6*dQ1*dQ5*m6*t11*t32*t34*t35*4.0+Lycm6*Lzcm6*dQ1*dQ5*m6*t11*t33*t34*t35*4.0+Lz6*Lzcm6*dQ2*dQ3*m6*t2*t3*t4*t9*4.0+Lz6*Lzcm6*dQ4*dQ5*m6*t2*t3*t5*t10*4.0-Lz6*Lzcm6*dQ2*dQ3*m6*t4*t7*t8*t9*4.0;
et172 = Lz6*Lzcm6*dQ4*dQ5*m6*t5*t7*t8*t10*-4.0-Lz6*Lzcm6*dQ1*dQ5*m6*t2*t4*t7*t33*8.0-Lz6*Lzcm6*dQ1*dQ5*m6*t3*t4*t8*t32*8.0-Lz6*Lzcm6*dQ1*dQ2*m6*t4*t5*t10*t32*8.0-Lz6*Lzcm6*dQ1*dQ5*m6*t2*t4*t7*t35*8.0-Lz6*Lzcm6*dQ1*dQ2*m6*t4*t5*t10*t33*8.0-Lz6*Lzcm6*dQ1*dQ3*m6*t4*t5*t10*t32*8.0-Lz6*Lzcm6*dQ1*dQ3*m6*t4*t5*t10*t33*8.0-Lz6*Lzcm6*dQ1*dQ5*m6*t3*t4*t8*t35*8.0-Lz6*Lzcm6*dQ2*dQ5*m6*t2*t3*t9*t35*4.0-Lz6*Lzcm6*dQ3*dQ5*m6*t2*t3*t9*t35*4.0+Lz6*Lzcm6*dQ4*dQ5*m6*t2*t4*t8*t35*4.0+Lz6*Lzcm6*dQ4*dQ5*m6*t3*t4*t7*t35*4.0+Lz6*Lzcm6*dQ2*dQ5*m6*t7*t8*t9*t35*4.0+Lz6*Lzcm6*dQ3*dQ5*m6*t7*t8*t9*t35*4.0-Lz6*Lzcm6*dQ1*dQ2*m6*t2*t7*t33*t34*8.0;
et173 = Lz6*Lzcm6*dQ1*dQ2*m6*t2*t7*t33*t35*8.0-Lz6*Lzcm6*dQ1*dQ2*m6*t3*t8*t32*t34*8.0-Lz6*Lzcm6*dQ1*dQ3*m6*t2*t7*t33*t34*8.0-Lz6*Lzcm6*dQ1*dQ2*m6*t2*t7*t34*t35*4.0+Lz6*Lzcm6*dQ1*dQ2*m6*t3*t8*t32*t35*8.0+Lz6*Lzcm6*dQ1*dQ3*m6*t2*t7*t33*t35*8.0-Lz6*Lzcm6*dQ1*dQ3*m6*t3*t8*t32*t34*8.0-Lz6*Lzcm6*dQ1*dQ3*m6*t2*t7*t34*t35*4.0+Lz6*Lzcm6*dQ1*dQ3*m6*t3*t8*t32*t35*8.0-Lz6*Lzcm6*dQ1*dQ2*m6*t3*t8*t34*t35*4.0-Lz6*Lzcm6*dQ1*dQ4*m6*t4*t9*t32*t33*8.0-Lz6*Lzcm6*dQ1*dQ3*m6*t3*t8*t34*t35*4.0-Lz6*Lzcm6*dQ1*dQ4*m6*t4*t9*t32*t35*4.0-Lz6*Lzcm6*dQ2*dQ4*m6*t2*t8*t34*t35*4.0-Lz6*Lzcm6*dQ2*dQ4*m6*t3*t7*t34*t35*4.0-Lz6*Lzcm6*dQ1*dQ4*m6*t4*t9*t33*t35*4.0;
et174 = Lz6*Lzcm6*dQ1*dQ5*m6*t5*t10*t32*t33*8.0-Lz6*Lzcm6*dQ3*dQ4*m6*t2*t8*t34*t35*4.0-Lz6*Lzcm6*dQ3*dQ4*m6*t3*t7*t34*t35*4.0-Lz6*Lzcm6*dQ1*dQ5*m6*t5*t10*t32*t34*4.0-Lz6*Lzcm6*dQ1*dQ5*m6*t5*t10*t33*t34*4.0+Lx3*Lx4*dQ1*dQ4*m4*t2*t3*t7*t8*t9*4.0+Lx3*Lx4*dQ1*dQ4*m5*t2*t3*t7*t8*t9*4.0+Lx3*Lx4*dQ1*dQ4*m6*t2*t3*t7*t8*t9*4.0-Lx2*Lxcm5*dQ1*dQ2*m5*t2*t3*t4*t5*t7*4.0-Lx2*Lxcm5*dQ1*dQ3*m5*t2*t3*t4*t5*t7*2.0+Lx3*Lxcm6*dQ1*dQ2*m6*t2*t4*t5*t6*t7*4.0+Lx4*Lxcm5*dQ2*dQ3*m5*t2*t3*t4*t5*t9*4.0-Lx2*Lxcm6*dQ1*dQ5*m6*t2*t3*t5*t6*t7*2.0+Lx3*Lxcm6*dQ1*dQ3*m6*t2*t4*t5*t6*t7*4.0+Lx3*Lxcm6*dQ1*dQ2*m6*t3*t4*t5*t6*t8*4.0+Lx3*Lxcm4*dQ1*dQ4*m4*t2*t3*t7*t8*t9*4.0;
et175 = Lx3*Lxcm6*dQ1*dQ3*m6*t3*t4*t5*t6*t8*4.0+Lx3*Lxcm6*dQ2*dQ3*m6*t2*t3*t5*t6*t9*2.0+Lx3*Lxcm5*dQ1*dQ2*m5*t2*t3*t7*t8*t10*8.0+Lx4*Lxcm6*dQ1*dQ5*m6*t2*t4*t5*t6*t7*2.0+Lx3*Lxcm5*dQ1*dQ3*m5*t2*t3*t7*t8*t10*8.0+Lx2*Lxcm5*dQ1*dQ4*m5*t2*t5*t7*t8*t9*2.0+Lx4*Lxcm6*dQ1*dQ5*m6*t3*t4*t5*t6*t8*2.0+Lx4*Lxcm6*dQ2*dQ5*m6*t2*t3*t5*t6*t9*2.0+Lx2*Lxcm5*dQ1*dQ5*m5*t2*t4*t7*t8*t10*2.0+Lx2*Lxcm6*dQ1*dQ2*m6*t2*t3*t7*t9*t11*4.0-Lx3*Lxcm6*dQ4*dQ5*m6*t2*t3*t4*t6*t10*2.0+Lx4*Lxcm6*dQ3*dQ5*m6*t2*t3*t5*t6*t9*2.0+Lx2*Lxcm6*dQ1*dQ2*m6*t2*t6*t7*t8*t10*4.0+Lx2*Lxcm6*dQ1*dQ3*m6*t2*t3*t7*t9*t11*2.0-Lx3*Lxcm6*dQ4*dQ6*m6*t2*t3*t4*t5*t11*2.0+Lx2*Lxcm6*dQ1*dQ3*m6*t2*t6*t7*t8*t10*2.0;
et176 = Lx2*Lxcm6*dQ1*dQ4*m6*t2*t4*t7*t8*t11*2.0-Lx4*Lxcm5*dQ2*dQ3*m5*t4*t5*t7*t8*t9*4.0-Lx4*Lxcm6*dQ1*dQ2*m6*t2*t4*t7*t9*t11*4.0-Lx4*Lxcm6*dQ1*dQ4*m6*t2*t3*t7*t8*t11*4.0+Lx2*Lxcm6*dQ1*dQ6*m6*t2*t6*t7*t8*t9*2.0-Lx4*Lxcm6*dQ1*dQ3*m6*t2*t4*t7*t9*t11*4.0+Lx2*Lxcm6*dQ1*dQ6*m6*t2*t3*t7*t10*t11*2.0-Lx4*Lxcm5*dQ2*dQ5*m5*t2*t4*t8*t9*t10*2.0-Lx4*Lxcm5*dQ2*dQ5*m5*t3*t4*t7*t9*t10*2.0-Lx4*Lxcm6*dQ1*dQ2*m6*t3*t4*t8*t9*t11*4.0-Lx3*Lxcm6*dQ2*dQ3*m6*t5*t6*t7*t8*t9*2.0-Lx4*Lxcm5*dQ3*dQ5*m5*t2*t4*t8*t9*t10*2.0-Lx4*Lxcm5*dQ3*dQ5*m5*t3*t4*t7*t9*t10*2.0-Lx4*Lxcm6*dQ1*dQ3*m6*t3*t4*t8*t9*t11*4.0-Lx4*Lxcm6*dQ1*dQ4*m6*t2*t6*t7*t9*t10*2.0;
et177 = Lx4*Lxcm6*dQ2*dQ3*m6*t2*t6*t8*t9*t10*-2.0-Lx4*Lxcm6*dQ2*dQ3*m6*t3*t6*t7*t9*t10*2.0-Lx4*Lxcm6*dQ2*dQ4*m6*t2*t4*t8*t9*t11*4.0-Lx4*Lxcm6*dQ2*dQ4*m6*t3*t4*t7*t9*t11*4.0-Lx4*Lxcm6*dQ1*dQ4*m6*t3*t6*t8*t9*t10*2.0-Lx4*Lxcm6*dQ1*dQ6*m6*t2*t4*t7*t10*t11*2.0-Lx4*Lxcm6*dQ3*dQ4*m6*t2*t4*t8*t9*t11*4.0-Lx4*Lxcm6*dQ3*dQ4*m6*t3*t4*t7*t9*t11*4.0-Lx4*Lxcm6*dQ2*dQ5*m6*t5*t6*t7*t8*t9*2.0+Lx3*Lxcm6*dQ4*dQ5*m6*t4*t6*t7*t8*t10*2.0-Lx4*Lxcm6*dQ1*dQ6*m6*t3*t4*t8*t10*t11*2.0-Lx4*Lxcm6*dQ2*dQ6*m6*t2*t3*t9*t10*t11*2.0-Lx4*Lxcm6*dQ3*dQ5*m6*t5*t6*t7*t8*t9*2.0+Lx3*Lxcm6*dQ4*dQ6*m6*t4*t5*t7*t8*t11*2.0-Lx4*Lxcm6*dQ3*dQ6*m6*t2*t3*t9*t10*t11*2.0;
et178 = Lx3*Lxcm6*dQ5*dQ6*m6*t2*t3*t9*t10*t11*2.0-Lx4*Lxcm6*dQ5*dQ6*m6*t2*t5*t8*t9*t11*2.0-Lx4*Lxcm6*dQ5*dQ6*m6*t3*t5*t7*t9*t11*2.0-Lx3*Lxcm5*dQ1*dQ2*m5*t2*t4*t5*t7*t33*8.0-Lx3*Lxcm5*dQ1*dQ2*m5*t3*t4*t5*t8*t32*8.0-Lx3*Lxcm5*dQ1*dQ3*m5*t2*t4*t5*t7*t33*8.0-Lx3*Lxcm5*dQ1*dQ3*m5*t3*t4*t5*t8*t32*8.0+Lx4*Lxcm6*dQ2*dQ6*m6*t7*t8*t9*t10*t11*2.0+Lx4*Lxcm6*dQ3*dQ6*m6*t7*t8*t9*t10*t11*2.0-Lx3*Lxcm6*dQ5*dQ6*m6*t7*t8*t9*t10*t11*2.0-Lx4*Lxcm5*dQ1*dQ5*m5*t2*t4*t5*t7*t33*4.0-Lx2*Lxcm6*dQ1*dQ2*m6*t4*t5*t6*t8*t32*4.0-Lx4*Lxcm5*dQ1*dQ5*m5*t3*t4*t5*t8*t32*4.0-Lx2*Lxcm6*dQ1*dQ3*m6*t4*t5*t6*t8*t32*2.0+Lx4*Lxcm6*dQ1*dQ2*m6*t2*t5*t6*t7*t34*4.0;
et179 = Lx2*Lxcm6*dQ1*dQ4*m6*t3*t5*t6*t9*t32*-2.0-Lx3*Lxcm6*dQ1*dQ5*m6*t2*t5*t6*t7*t33*4.0+Lx4*Lxcm6*dQ1*dQ3*m6*t2*t5*t6*t7*t34*4.0-Lx2*Lxcm6*dQ1*dQ5*m6*t3*t4*t6*t10*t32*2.0-Lx3*Lxcm6*dQ1*dQ5*m6*t3*t5*t6*t8*t32*4.0+Lx4*Lxcm6*dQ1*dQ2*m6*t3*t5*t6*t8*t34*4.0-Lx2*Lxcm6*dQ1*dQ6*m6*t3*t4*t5*t11*t32*2.0+Lx4*Lxcm6*dQ1*dQ3*m6*t3*t5*t6*t8*t34*4.0+Lx4*Lxcm6*dQ1*dQ4*m6*t4*t5*t6*t9*t32*4.0+Lx4*Lxcm6*dQ2*dQ4*m6*t2*t5*t6*t8*t34*4.0+Lx4*Lxcm6*dQ2*dQ4*m6*t3*t5*t6*t7*t34*4.0+Lx4*Lxcm6*dQ1*dQ4*m6*t4*t5*t6*t9*t33*4.0+Lx4*Lxcm6*dQ3*dQ4*m6*t2*t5*t6*t8*t34*4.0+Lx4*Lxcm6*dQ3*dQ4*m6*t3*t5*t6*t7*t34*4.0+Lx3*Lxcm6*dQ1*dQ2*m6*t2*t7*t9*t11*t33*8.0+Lx4*Lxcm5*dQ1*dQ4*m5*t2*t7*t9*t10*t33*4.0;
et180 = Lx3*Lxcm6*dQ1*dQ2*m6*t3*t8*t9*t11*t32*8.0+Lx3*Lxcm6*dQ1*dQ3*m6*t2*t7*t9*t11*t33*8.0+Lx4*Lxcm5*dQ1*dQ4*m5*t3*t8*t9*t10*t32*4.0+Lx3*Lxcm6*dQ1*dQ3*m6*t3*t8*t9*t11*t32*8.0+Lx3*Lxcm6*dQ1*dQ6*m6*t2*t7*t10*t11*t33*4.0+Lx3*Lxcm6*dQ1*dQ6*m6*t3*t8*t10*t11*t32*4.0-Lx4*Lxcm5*dQ1*dQ2*m5*t2*t5*t7*t33*t34*8.0-Lx4*Lxcm5*dQ1*dQ2*m5*t3*t5*t8*t32*t34*8.0-Lx4*Lxcm5*dQ1*dQ3*m5*t2*t5*t7*t33*t34*8.0-Lx4*Lxcm5*dQ1*dQ3*m5*t3*t5*t8*t32*t34*8.0-Lx4*Lxcm5*dQ1*dQ4*m5*t4*t5*t9*t32*t33*8.0-Lx4*Lxcm6*dQ1*dQ2*m6*t4*t6*t10*t32*t33*8.0-Lx3*Lxcm6*dQ1*dQ4*m6*t5*t6*t9*t32*t33*4.0-Lx4*Lxcm6*dQ1*dQ3*m6*t4*t6*t10*t32*t33*8.0-Lx3*Lxcm6*dQ1*dQ5*m6*t4*t6*t10*t32*t33*4.0;
et181 = Lx3*Lxcm6*dQ1*dQ6*m6*t4*t5*t11*t32*t33*-4.0-Lx4*Lxcm6*dQ1*dQ6*m6*t4*t6*t9*t32*t33*4.0-Lx4*Lxcm6*dQ1*dQ5*m6*t6*t10*t32*t33*t34*4.0-Lx4*Lxcm6*dQ1*dQ6*m6*t5*t11*t32*t33*t34*4.0+Lx3*Lycm4*dQ1*dQ4*m4*t2*t3*t4*t7*t8*4.0+Lx3*Lycm5*dQ1*dQ4*m5*t2*t3*t4*t7*t8*4.0+Lx2*Lycm6*dQ1*dQ2*m6*t2*t3*t6*t7*t9*4.0+Lx2*Lycm6*dQ1*dQ3*m6*t2*t3*t6*t7*t9*2.0-Lx3*Lycm6*dQ4*dQ6*m6*t2*t3*t4*t5*t6*2.0+Lx2*Lycm6*dQ1*dQ4*m6*t2*t4*t6*t7*t8*2.0-Lx3*Lycm6*dQ1*dQ2*m6*t2*t4*t5*t7*t11*4.0-Lx4*Lycm6*dQ1*dQ2*m6*t2*t4*t6*t7*t9*4.0-Lx4*Lycm6*dQ1*dQ4*m6*t2*t3*t6*t7*t8*4.0+Lx2*Lycm6*dQ1*dQ5*m6*t2*t3*t5*t7*t11*2.0-Lx3*Lycm6*dQ1*dQ3*m6*t2*t4*t5*t7*t11*4.0;
et182 = Lx4*Lycm6*dQ1*dQ3*m6*t2*t4*t6*t7*t9*-4.0+Lx2*Lycm6*dQ1*dQ6*m6*t2*t3*t6*t7*t10*2.0-Lx3*Lycm6*dQ1*dQ2*m6*t3*t4*t5*t8*t11*4.0-Lx4*Lycm6*dQ1*dQ2*m6*t3*t4*t6*t8*t9*4.0-Lx3*Lycm6*dQ1*dQ3*m6*t3*t4*t5*t8*t11*4.0-Lx3*Lycm6*dQ2*dQ3*m6*t2*t3*t5*t9*t11*2.0-Lx4*Lycm6*dQ1*dQ3*m6*t3*t4*t6*t8*t9*4.0-Lx4*Lycm6*dQ1*dQ5*m6*t2*t4*t5*t7*t11*2.0-Lx4*Lycm6*dQ2*dQ4*m6*t2*t4*t6*t8*t9*4.0-Lx4*Lycm6*dQ2*dQ4*m6*t3*t4*t6*t7*t9*4.0-Lx4*Lycm6*dQ1*dQ6*m6*t2*t4*t6*t7*t10*2.0-Lx4*Lycm6*dQ3*dQ4*m6*t2*t4*t6*t8*t9*4.0-Lx4*Lycm6*dQ3*dQ4*m6*t3*t4*t6*t7*t9*4.0-Lx4*Lycm6*dQ1*dQ5*m6*t3*t4*t5*t8*t11*2.0-Lx4*Lycm6*dQ2*dQ5*m6*t2*t3*t5*t9*t11*2.0;
et183 = Lx3*Lycm6*dQ4*dQ5*m6*t2*t3*t4*t10*t11*2.0-Lx4*Lycm6*dQ1*dQ6*m6*t3*t4*t6*t8*t10*2.0-Lx4*Lycm6*dQ2*dQ6*m6*t2*t3*t6*t9*t10*2.0-Lx4*Lycm6*dQ3*dQ5*m6*t2*t3*t5*t9*t11*2.0-Lx2*Lycm6*dQ1*dQ2*m6*t2*t7*t8*t10*t11*4.0+Lx3*Lycm6*dQ4*dQ6*m6*t4*t5*t6*t7*t8*2.0-Lx4*Lycm6*dQ3*dQ6*m6*t2*t3*t6*t9*t10*2.0-Lx2*Lycm6*dQ1*dQ3*m6*t2*t7*t8*t10*t11*2.0+Lx3*Lycm6*dQ5*dQ6*m6*t2*t3*t6*t9*t10*2.0-Lx4*Lycm6*dQ5*dQ6*m6*t2*t5*t6*t8*t9*2.0-Lx4*Lycm6*dQ5*dQ6*m6*t3*t5*t6*t7*t9*2.0-Lx2*Lycm6*dQ1*dQ6*m6*t2*t7*t8*t9*t11*2.0+Lx3*Lycm6*dQ2*dQ3*m6*t5*t7*t8*t9*t11*2.0+Lx4*Lycm6*dQ1*dQ4*m6*t2*t7*t9*t10*t11*2.0+Lx4*Lycm6*dQ2*dQ3*m6*t2*t8*t9*t10*t11*2.0;
et184 = Lx4*Lycm6*dQ2*dQ3*m6*t3*t7*t9*t10*t11*2.0+Lx4*Lycm6*dQ1*dQ4*m6*t3*t8*t9*t10*t11*2.0+Lx4*Lycm6*dQ2*dQ5*m6*t5*t7*t8*t9*t11*2.0-Lx3*Lycm6*dQ4*dQ5*m6*t4*t7*t8*t10*t11*2.0+Lx4*Lycm6*dQ2*dQ6*m6*t6*t7*t8*t9*t10*2.0+Lx4*Lycm6*dQ3*dQ5*m6*t5*t7*t8*t9*t11*2.0+Lx4*Lycm6*dQ3*dQ6*m6*t6*t7*t8*t9*t10*2.0-Lx3*Lycm6*dQ5*dQ6*m6*t6*t7*t8*t9*t10*2.0+Lx4*Lycm4*dQ1*dQ2*m4*t2*t4*t7*t9*t33*8.0-Lx2*Lycm6*dQ1*dQ6*m6*t3*t4*t5*t6*t32*2.0+Lx4*Lycm4*dQ1*dQ2*m4*t3*t4*t8*t9*t32*8.0+Lx4*Lycm4*dQ1*dQ3*m4*t2*t4*t7*t9*t33*8.0+Lx4*Lycm4*dQ1*dQ4*m4*t2*t3*t7*t8*t34*8.0+Lx4*Lycm4*dQ1*dQ3*m4*t3*t4*t8*t9*t32*8.0+Lx4*Lycm5*dQ1*dQ2*m5*t2*t4*t7*t9*t33*8.0;
et185 = Lx4*Lycm5*dQ1*dQ2*m5*t3*t4*t8*t9*t32*8.0+Lx4*Lycm5*dQ1*dQ3*m5*t2*t4*t7*t9*t33*8.0+Lx4*Lycm5*dQ1*dQ4*m5*t2*t3*t7*t8*t34*8.0+Lx4*Lycm5*dQ1*dQ3*m5*t3*t4*t8*t9*t32*8.0+Lx3*Lycm6*dQ1*dQ2*m6*t2*t6*t7*t9*t33*8.0+Lx3*Lycm6*dQ1*dQ2*m6*t3*t6*t8*t9*t32*8.0+Lx3*Lycm6*dQ1*dQ3*m6*t2*t6*t7*t9*t33*8.0+Lx2*Lycm6*dQ1*dQ2*m6*t4*t5*t8*t11*t32*4.0+Lx3*Lycm6*dQ1*dQ3*m6*t3*t6*t8*t9*t32*8.0+Lx2*Lycm6*dQ1*dQ3*m6*t4*t5*t8*t11*t32*2.0-Lx4*Lycm6*dQ1*dQ2*m6*t2*t5*t7*t11*t34*4.0+Lx2*Lycm6*dQ1*dQ4*m6*t3*t5*t9*t11*t32*2.0+Lx3*Lycm6*dQ1*dQ5*m6*t2*t5*t7*t11*t33*4.0-Lx4*Lycm6*dQ1*dQ3*m6*t2*t5*t7*t11*t34*4.0+Lx2*Lycm6*dQ1*dQ5*m6*t3*t4*t10*t11*t32*2.0;
et186 = Lx3*Lycm6*dQ1*dQ5*m6*t3*t5*t8*t11*t32*4.0+Lx3*Lycm6*dQ1*dQ6*m6*t2*t6*t7*t10*t33*4.0-Lx4*Lycm6*dQ1*dQ2*m6*t3*t5*t8*t11*t34*4.0+Lx3*Lycm6*dQ1*dQ6*m6*t3*t6*t8*t10*t32*4.0-Lx4*Lycm6*dQ1*dQ3*m6*t3*t5*t8*t11*t34*4.0-Lx4*Lycm6*dQ1*dQ4*m6*t4*t5*t9*t11*t32*4.0-Lx4*Lycm6*dQ2*dQ4*m6*t2*t5*t8*t11*t34*4.0-Lx4*Lycm6*dQ2*dQ4*m6*t3*t5*t7*t11*t34*4.0-Lx4*Lycm6*dQ1*dQ4*m6*t4*t5*t9*t11*t33*4.0-Lx4*Lycm6*dQ3*dQ4*m6*t2*t5*t8*t11*t34*4.0-Lx4*Lycm6*dQ3*dQ4*m6*t3*t5*t7*t11*t34*4.0-Lx3*Lycm6*dQ1*dQ6*m6*t4*t5*t6*t32*t33*4.0+Lx4*Lycm6*dQ1*dQ2*m6*t4*t10*t11*t32*t33*8.0+Lx3*Lycm6*dQ1*dQ4*m6*t5*t9*t11*t32*t33*4.0+Lx4*Lycm6*dQ1*dQ3*m6*t4*t10*t11*t32*t33*8.0;
et187 = Lx3*Lycm6*dQ1*dQ5*m6*t4*t10*t11*t32*t33*4.0+Lx4*Lycm6*dQ1*dQ6*m6*t4*t9*t11*t32*t33*4.0-Lx4*Lycm6*dQ1*dQ6*m6*t5*t6*t32*t33*t34*4.0+Lx4*Lycm6*dQ1*dQ5*m6*t10*t11*t32*t33*t34*4.0-Lxcm5*Lycm5*dQ1*dQ2*m5*t2*t4*t5*t7*t9*4.0-Lxcm5*Lycm5*dQ1*dQ4*m5*t2*t3*t5*t7*t8*4.0-Lxcm5*Lycm5*dQ1*dQ3*m5*t2*t4*t5*t7*t9*4.0-Lxcm5*Lycm5*dQ1*dQ2*m5*t3*t4*t5*t8*t9*4.0-Lxcm5*Lycm5*dQ1*dQ3*m5*t3*t4*t5*t8*t9*4.0+Lxcm6*Lycm6*dQ1*dQ2*m6*t2*t4*t5*t7*t9*4.0+Lxcm6*Lycm6*dQ1*dQ4*m6*t2*t3*t5*t7*t8*4.0-Lxcm5*Lycm5*dQ2*dQ4*m5*t2*t4*t5*t8*t9*4.0-Lxcm5*Lycm5*dQ2*dQ4*m5*t3*t4*t5*t7*t9*4.0+Lxcm6*Lycm6*dQ1*dQ3*m6*t2*t4*t5*t7*t9*4.0-Lxcm5*Lycm5*dQ3*dQ4*m5*t2*t4*t5*t8*t9*4.0;
et188 = Lxcm5*Lycm5*dQ3*dQ4*m5*t3*t4*t5*t7*t9*-4.0+Lxcm6*Lycm6*dQ1*dQ2*m6*t3*t4*t5*t8*t9*4.0+Lxcm6*Lycm6*dQ1*dQ3*m6*t3*t4*t5*t8*t9*4.0+Lxcm6*Lycm6*dQ2*dQ4*m6*t2*t4*t5*t8*t9*4.0+Lxcm6*Lycm6*dQ2*dQ4*m6*t3*t4*t5*t7*t9*4.0+Lxcm6*Lycm6*dQ1*dQ6*m6*t2*t4*t5*t7*t10*4.0+Lxcm6*Lycm6*dQ3*dQ4*m6*t2*t4*t5*t8*t9*4.0+Lxcm6*Lycm6*dQ3*dQ4*m6*t3*t4*t5*t7*t9*4.0+Lxcm6*Lycm6*dQ1*dQ5*m6*t2*t4*t6*t7*t11*4.0+Lxcm6*Lycm6*dQ1*dQ6*m6*t3*t4*t5*t8*t10*4.0+Lxcm6*Lycm6*dQ2*dQ6*m6*t2*t3*t5*t9*t10*2.0+Lxcm6*Lycm6*dQ1*dQ5*m6*t3*t4*t6*t8*t11*4.0+Lxcm6*Lycm6*dQ3*dQ6*m6*t2*t3*t5*t9*t10*2.0+Lxcm6*Lycm6*dQ1*dQ2*m6*t4*t5*t6*t10*t11*4.0-Lxcm6*Lycm6*dQ4*dQ6*m6*t2*t4*t5*t8*t10*2.0-Lxcm6*Lycm6*dQ4*dQ6*m6*t3*t4*t5*t7*t10*2.0;
et189 = Lxcm6*Lycm6*dQ1*dQ3*m6*t4*t5*t6*t10*t11*4.0+Lxcm6*Lycm6*dQ2*dQ6*m6*t2*t5*t6*t8*t11*4.0+Lxcm6*Lycm6*dQ2*dQ6*m6*t3*t5*t6*t7*t11*4.0-Lxcm6*Lycm6*dQ4*dQ5*m6*t2*t4*t6*t8*t11*4.0-Lxcm6*Lycm6*dQ4*dQ5*m6*t3*t4*t6*t7*t11*4.0+Lxcm6*Lycm6*dQ3*dQ6*m6*t2*t5*t6*t8*t11*4.0+Lxcm6*Lycm6*dQ3*dQ6*m6*t3*t5*t6*t7*t11*4.0-Lxcm6*Lycm6*dQ5*dQ6*m6*t2*t3*t6*t10*t11*4.0-Lxcm6*Lycm6*dQ2*dQ6*m6*t5*t7*t8*t9*t10*2.0-Lxcm6*Lycm6*dQ3*dQ6*m6*t5*t7*t8*t9*t10*2.0+Lxcm4*Lycm4*dQ1*dQ2*m4*t2*t4*t7*t9*t33*8.0+Lxcm4*Lycm4*dQ1*dQ2*m4*t3*t4*t8*t9*t32*8.0+Lxcm4*Lycm4*dQ1*dQ3*m4*t2*t4*t7*t9*t33*8.0+Lxcm4*Lycm4*dQ1*dQ4*m4*t2*t3*t7*t8*t34*8.0+Lxcm6*Lycm6*dQ5*dQ6*m6*t6*t7*t8*t10*t11*4.0;
et190 = Lxcm4*Lycm4*dQ1*dQ3*m4*t3*t4*t8*t9*t32*8.0+Lxcm6*Lycm6*dQ2*dQ5*m6*t2*t3*t4*t5*t36*4.0+Lxcm5*Lycm5*dQ1*dQ4*m5*t2*t4*t7*t10*t33*4.0+Lxcm6*Lycm6*dQ3*dQ5*m6*t2*t3*t4*t5*t36*4.0+Lxcm5*Lycm5*dQ1*dQ4*m5*t3*t4*t8*t10*t32*4.0+Lxcm5*Lycm5*dQ1*dQ5*m5*t2*t5*t7*t9*t33*4.0+Lxcm5*Lycm5*dQ1*dQ5*m5*t3*t5*t8*t9*t32*4.0-Lxcm6*Lycm6*dQ1*dQ4*m6*t2*t4*t7*t10*t33*4.0-Lxcm6*Lycm6*dQ1*dQ6*m6*t2*t3*t7*t8*t34*4.0-Lxcm6*Lycm6*dQ1*dQ2*m6*t2*t6*t7*t11*t33*1.6e+1-Lxcm6*Lycm6*dQ1*dQ4*m6*t3*t4*t8*t10*t32*4.0-Lxcm6*Lycm6*dQ1*dQ5*m6*t2*t5*t7*t9*t33*4.0-Lxcm6*Lycm6*dQ1*dQ6*m6*t2*t3*t7*t8*t35*4.0-Lxcm6*Lycm6*dQ1*dQ2*m6*t2*t6*t7*t11*t34*4.0-Lxcm6*Lycm6*dQ1*dQ2*m6*t3*t6*t8*t11*t32*1.6e+1;
et191 = Lxcm6*Lycm6*dQ1*dQ3*m6*t2*t6*t7*t11*t33*-1.6e+1-Lxcm6*Lycm6*dQ1*dQ5*m6*t3*t5*t8*t9*t32*4.0-Lxcm6*Lycm6*dQ1*dQ6*m6*t2*t3*t7*t8*t36*1.6e+1-Lxcm6*Lycm6*dQ1*dQ2*m6*t2*t6*t7*t11*t35*4.0-Lxcm6*Lycm6*dQ1*dQ3*m6*t2*t6*t7*t11*t34*4.0-Lxcm6*Lycm6*dQ1*dQ3*m6*t3*t6*t8*t11*t32*1.6e+1-Lxcm6*Lycm6*dQ1*dQ4*m6*t2*t4*t7*t10*t36*4.0-Lxcm6*Lycm6*dQ1*dQ2*m6*t3*t6*t8*t11*t34*4.0-Lxcm6*Lycm6*dQ1*dQ3*m6*t2*t6*t7*t11*t35*4.0-Lxcm6*Lycm6*dQ1*dQ5*m6*t2*t5*t7*t9*t36*4.0-Lxcm6*Lycm6*dQ2*dQ3*m6*t2*t4*t8*t10*t36*4.0-Lxcm6*Lycm6*dQ2*dQ3*m6*t3*t4*t7*t10*t36*4.0-Lxcm6*Lycm6*dQ1*dQ2*m6*t3*t6*t8*t11*t35*4.0-Lxcm6*Lycm6*dQ1*dQ3*m6*t3*t6*t8*t11*t34*4.0-Lxcm6*Lycm6*dQ1*dQ4*m6*t3*t4*t8*t10*t36*4.0;
et192 = Lxcm6*Lycm6*dQ1*dQ3*m6*t3*t6*t8*t11*t35*-4.0-Lxcm6*Lycm6*dQ1*dQ4*m6*t4*t6*t9*t11*t32*4.0-Lxcm6*Lycm6*dQ1*dQ5*m6*t3*t5*t8*t9*t36*4.0-Lxcm6*Lycm6*dQ2*dQ4*m6*t2*t6*t8*t11*t34*4.0-Lxcm6*Lycm6*dQ2*dQ4*m6*t3*t6*t7*t11*t34*4.0-Lxcm6*Lycm6*dQ2*dQ5*m6*t4*t5*t7*t8*t36*4.0-Lxcm6*Lycm6*dQ2*dQ6*m6*t2*t4*t8*t9*t36*4.0-Lxcm6*Lycm6*dQ2*dQ6*m6*t3*t4*t7*t9*t36*4.0-Lxcm6*Lycm6*dQ1*dQ4*m6*t4*t6*t9*t11*t33*4.0+Lxcm6*Lycm6*dQ2*dQ4*m6*t2*t6*t8*t11*t35*4.0+Lxcm6*Lycm6*dQ2*dQ4*m6*t3*t6*t7*t11*t35*4.0-Lxcm6*Lycm6*dQ3*dQ4*m6*t2*t6*t8*t11*t34*4.0-Lxcm6*Lycm6*dQ3*dQ4*m6*t3*t6*t7*t11*t34*4.0-Lxcm6*Lycm6*dQ3*dQ5*m6*t4*t5*t7*t8*t36*4.0-Lxcm6*Lycm6*dQ3*dQ6*m6*t2*t4*t8*t9*t36*4.0;
et193 = Lxcm6*Lycm6*dQ3*dQ6*m6*t3*t4*t7*t9*t36*-4.0+Lxcm6*Lycm6*dQ3*dQ4*m6*t2*t6*t8*t11*t35*4.0+Lxcm6*Lycm6*dQ3*dQ4*m6*t3*t6*t7*t11*t35*4.0-Lxcm6*Lycm6*dQ1*dQ5*m6*t5*t6*t10*t11*t32*4.0-Lxcm6*Lycm6*dQ1*dQ5*m6*t5*t6*t10*t11*t33*4.0+Lxcm6*Lycm6*dQ2*dQ3*m6*t2*t3*t5*t34*t36*8.0+Lxcm5*Lycm5*dQ1*dQ5*m5*t4*t9*t10*t32*t33*4.0-Lxcm6*Lycm6*dQ1*dQ5*m6*t4*t9*t10*t32*t33*4.0-Lxcm6*Lycm6*dQ2*dQ3*m6*t5*t7*t8*t34*t36*8.0-Lxcm6*Lycm6*dQ1*dQ5*m6*t4*t9*t10*t32*t36*4.0-Lxcm6*Lycm6*dQ2*dQ5*m6*t2*t8*t10*t34*t36*4.0-Lxcm6*Lycm6*dQ2*dQ5*m6*t3*t7*t10*t34*t36*4.0-Lxcm6*Lycm6*dQ1*dQ5*m6*t4*t9*t10*t33*t36*4.0-Lxcm6*Lycm6*dQ3*dQ5*m6*t2*t8*t10*t34*t36*4.0-Lxcm6*Lycm6*dQ3*dQ5*m6*t3*t7*t10*t34*t36*4.0;
et194 = Lxcm6*Lycm6*dQ1*dQ2*m6*t9*t10*t32*t33*t36*1.6e+1+Lxcm6*Lycm6*dQ1*dQ3*m6*t9*t10*t32*t33*t36*1.6e+1-Lxcm6*Lycm6*dQ1*dQ4*m6*t5*t32*t33*t34*t36*1.6e+1-Lxcm6*Lycm6*dQ1*dQ6*m6*t32*t33*t34*t35*t36*8.0-Lx2*Lz6*dQ1*dQ2*m6*t2*t3*t4*t7*t10*4.0-Lx3*Lz6*dQ1*dQ2*m6*t2*t3*t5*t7*t8*8.0-Lx2*Lz6*dQ1*dQ3*m6*t2*t3*t4*t7*t10*2.0-Lx3*Lz6*dQ1*dQ3*m6*t2*t3*t5*t7*t8*8.0-Lx2*Lz6*dQ1*dQ5*m6*t2*t4*t5*t7*t8*2.0+Lx4*Lz6*dQ2*dQ3*m6*t2*t3*t4*t9*t10*4.0+Lx4*Lz6*dQ2*dQ5*m6*t2*t4*t5*t8*t9*2.0+Lx4*Lz6*dQ2*dQ5*m6*t3*t4*t5*t7*t9*2.0+Lx4*Lz6*dQ3*dQ5*m6*t2*t4*t5*t8*t9*2.0+Lx4*Lz6*dQ3*dQ5*m6*t3*t4*t5*t7*t9*2.0+Lx2*Lz6*dQ1*dQ4*m6*t2*t7*t8*t9*t10*2.0;
et195 = Lx4*Lz6*dQ2*dQ3*m6*t4*t7*t8*t9*t10*-4.0-Lx3*Lz6*dQ1*dQ2*m6*t2*t4*t7*t10*t33*8.0-Lx3*Lz6*dQ1*dQ2*m6*t3*t4*t8*t10*t32*8.0-Lx3*Lz6*dQ1*dQ3*m6*t2*t4*t7*t10*t33*8.0-Lx3*Lz6*dQ1*dQ3*m6*t3*t4*t8*t10*t32*8.0-Lx4*Lz6*dQ1*dQ4*m6*t2*t5*t7*t9*t33*4.0-Lx4*Lz6*dQ1*dQ4*m6*t3*t5*t8*t9*t32*4.0-Lx4*Lz6*dQ1*dQ5*m6*t2*t4*t7*t10*t33*4.0-Lx4*Lz6*dQ1*dQ5*m6*t3*t4*t8*t10*t32*4.0-Lx4*Lz6*dQ1*dQ2*m6*t2*t7*t10*t33*t34*8.0-Lx4*Lz6*dQ1*dQ2*m6*t3*t8*t10*t32*t34*8.0-Lx4*Lz6*dQ1*dQ3*m6*t2*t7*t10*t33*t34*8.0-Lx4*Lz6*dQ1*dQ3*m6*t3*t8*t10*t32*t34*8.0-Lx4*Lz6*dQ1*dQ4*m6*t4*t9*t10*t32*t33*8.0;
et196 = Lx4*Lzcm4*dQ1*dQ2*m4*t2*t3*t4*t7*t8*-8.0-Lx4*Lzcm4*dQ1*dQ3*m4*t2*t3*t4*t7*t8*8.0-Lx2*Lzcm5*dQ1*dQ2*m5*t2*t3*t4*t7*t10*4.0-Lx3*Lzcm5*dQ1*dQ2*m5*t2*t3*t5*t7*t8*8.0-Lx2*Lzcm5*dQ1*dQ3*m5*t2*t3*t4*t7*t10*2.0-Lx3*Lzcm5*dQ1*dQ3*m5*t2*t3*t5*t7*t8*8.0-Lx2*Lzcm6*dQ1*dQ2*m6*t2*t3*t4*t7*t10*4.0-Lx3*Lzcm6*dQ1*dQ2*m6*t2*t3*t5*t7*t8*8.0-Lx2*Lzcm5*dQ1*dQ5*m5*t2*t4*t5*t7*t8*2.0-Lx2*Lzcm6*dQ1*dQ3*m6*t2*t3*t4*t7*t10*2.0-Lx3*Lzcm6*dQ1*dQ3*m6*t2*t3*t5*t7*t8*8.0-Lx2*Lzcm6*dQ1*dQ5*m6*t2*t4*t5*t7*t8*2.0+Lx4*Lzcm5*dQ2*dQ3*m5*t2*t3*t4*t9*t10*4.0+Lx4*Lzcm5*dQ2*dQ5*m5*t2*t4*t5*t8*t9*2.0+Lx4*Lzcm5*dQ2*dQ5*m5*t3*t4*t5*t7*t9*2.0;
et197 = Lx4*Lzcm6*dQ2*dQ3*m6*t2*t3*t4*t9*t10*4.0+Lx4*Lzcm5*dQ3*dQ5*m5*t2*t4*t5*t8*t9*2.0+Lx4*Lzcm5*dQ3*dQ5*m5*t3*t4*t5*t7*t9*2.0+Lxcm6*Lz6*dQ1*dQ5*m6*t2*t3*t6*t7*t8*4.0+Lx4*Lzcm6*dQ2*dQ5*m6*t2*t4*t5*t8*t9*2.0+Lx4*Lzcm6*dQ2*dQ5*m6*t3*t4*t5*t7*t9*2.0+Lxcm6*Lz6*dQ1*dQ2*m6*t2*t5*t6*t7*t10*4.0+Lx4*Lzcm6*dQ3*dQ5*m6*t2*t4*t5*t8*t9*2.0+Lx4*Lzcm6*dQ3*dQ5*m6*t3*t4*t5*t7*t9*2.0+Lxcm6*Lz6*dQ1*dQ3*m6*t2*t5*t6*t7*t10*4.0+Lxcm6*Lz6*dQ1*dQ4*m6*t2*t4*t5*t7*t11*2.0+Lx2*Lzcm5*dQ1*dQ4*m5*t2*t7*t8*t9*t10*2.0+Lxcm6*Lz6*dQ1*dQ2*m6*t3*t5*t6*t8*t10*4.0+Lxcm6*Lz6*dQ2*dQ3*m6*t2*t4*t5*t8*t11*2.0+Lxcm6*Lz6*dQ2*dQ3*m6*t3*t4*t5*t7*t11*2.0+Lxcm6*Lz6*dQ1*dQ3*m6*t3*t5*t6*t8*t10*4.0;
et198 = Lxcm6*Lz6*dQ1*dQ4*m6*t3*t4*t5*t8*t11*2.0+Lxcm6*Lz6*dQ1*dQ6*m6*t2*t5*t6*t7*t9*2.0-Lxcm6*Lz6*dQ2*dQ5*m6*t2*t4*t6*t8*t9*2.0-Lxcm6*Lz6*dQ2*dQ5*m6*t3*t4*t6*t7*t9*2.0+Lx2*Lzcm6*dQ1*dQ4*m6*t2*t7*t8*t9*t10*2.0-Lxcm6*Lz6*dQ2*dQ4*m6*t2*t5*t6*t8*t10*4.0-Lxcm6*Lz6*dQ2*dQ4*m6*t3*t5*t6*t7*t10*4.0+Lxcm6*Lz6*dQ2*dQ5*m6*t2*t3*t4*t10*t11*2.0-Lxcm6*Lz6*dQ3*dQ5*m6*t2*t4*t6*t8*t9*2.0-Lxcm6*Lz6*dQ3*dQ5*m6*t3*t4*t6*t7*t9*2.0+Lxcm6*Lz6*dQ1*dQ6*m6*t3*t5*t6*t8*t9*2.0-Lxcm6*Lz6*dQ3*dQ4*m6*t2*t5*t6*t8*t10*4.0-Lxcm6*Lz6*dQ3*dQ4*m6*t3*t5*t6*t7*t10*4.0+Lxcm6*Lz6*dQ3*dQ5*m6*t2*t3*t4*t10*t11*2.0-Lx4*Lzcm5*dQ2*dQ3*m5*t4*t7*t8*t9*t10*4.0;
et199 = Lxcm6*Lz6*dQ4*dQ6*m6*t2*t5*t6*t8*t9*-2.0-Lxcm6*Lz6*dQ4*dQ6*m6*t3*t5*t6*t7*t9*2.0-Lx4*Lzcm6*dQ2*dQ3*m6*t4*t7*t8*t9*t10*4.0-Lxcm6*Lz6*dQ4*dQ6*m6*t2*t3*t5*t10*t11*2.0-Lxcm6*Lz6*dQ1*dQ5*m6*t2*t7*t9*t10*t11*2.0-Lxcm6*Lz6*dQ1*dQ5*m6*t3*t8*t9*t10*t11*2.0-Lxcm6*Lz6*dQ2*dQ5*m6*t4*t7*t8*t10*t11*2.0-Lxcm6*Lz6*dQ3*dQ5*m6*t4*t7*t8*t10*t11*2.0+Lxcm6*Lz6*dQ4*dQ6*m6*t5*t7*t8*t10*t11*2.0-Lx3*Lzcm5*dQ1*dQ2*m5*t2*t4*t7*t10*t33*8.0-Lx3*Lzcm5*dQ1*dQ2*m5*t3*t4*t8*t10*t32*8.0-Lx3*Lzcm5*dQ1*dQ3*m5*t2*t4*t7*t10*t33*8.0-Lx3*Lzcm5*dQ1*dQ3*m5*t3*t4*t8*t10*t32*8.0-Lx3*Lzcm6*dQ1*dQ2*m6*t2*t4*t7*t10*t33*8.0-Lx3*Lzcm6*dQ1*dQ2*m6*t3*t4*t8*t10*t32*8.0;
et200 = Lx3*Lzcm6*dQ1*dQ3*m6*t2*t4*t7*t10*t33*-8.0-Lx4*Lzcm5*dQ1*dQ4*m5*t2*t5*t7*t9*t33*4.0-Lx3*Lzcm6*dQ1*dQ3*m6*t3*t4*t8*t10*t32*8.0-Lx4*Lzcm5*dQ1*dQ4*m5*t3*t5*t8*t9*t32*4.0-Lx4*Lzcm5*dQ1*dQ5*m5*t2*t4*t7*t10*t33*4.0-Lx4*Lzcm5*dQ1*dQ5*m5*t3*t4*t8*t10*t32*4.0-Lx4*Lzcm6*dQ1*dQ4*m6*t2*t5*t7*t9*t33*4.0-Lx4*Lzcm6*dQ1*dQ4*m6*t3*t5*t8*t9*t32*4.0-Lx4*Lzcm6*dQ1*dQ5*m6*t2*t4*t7*t10*t33*4.0-Lx4*Lzcm6*dQ1*dQ5*m6*t3*t4*t8*t10*t32*4.0+Lxcm6*Lz6*dQ1*dQ4*m6*t2*t6*t7*t9*t33*4.0+Lxcm6*Lz6*dQ1*dQ4*m6*t3*t6*t8*t9*t32*4.0+Lxcm6*Lz6*dQ1*dQ4*m6*t2*t6*t7*t9*t35*4.0+Lxcm6*Lz6*dQ1*dQ6*m6*t2*t4*t7*t11*t33*4.0+Lxcm6*Lz6*dQ1*dQ6*m6*t3*t4*t8*t11*t32*4.0;
et201 = Lxcm6*Lz6*dQ2*dQ3*m6*t2*t3*t10*t11*t34*4.0+Lxcm6*Lz6*dQ2*dQ3*m6*t2*t6*t8*t9*t35*4.0+Lxcm6*Lz6*dQ2*dQ3*m6*t3*t6*t7*t9*t35*4.0+Lxcm6*Lz6*dQ1*dQ4*m6*t3*t6*t8*t9*t35*4.0+Lxcm6*Lz6*dQ1*dQ6*m6*t2*t4*t7*t11*t35*4.0+Lxcm6*Lz6*dQ1*dQ5*m6*t4*t5*t9*t11*t32*2.0+Lxcm6*Lz6*dQ2*dQ5*m6*t2*t5*t8*t11*t34*2.0+Lxcm6*Lz6*dQ2*dQ5*m6*t3*t5*t7*t11*t34*2.0+Lxcm6*Lz6*dQ1*dQ5*m6*t4*t5*t9*t11*t33*2.0+Lxcm6*Lz6*dQ1*dQ6*m6*t3*t4*t8*t11*t35*4.0+Lxcm6*Lz6*dQ1*dQ6*m6*t4*t6*t9*t10*t32*2.0+Lxcm6*Lz6*dQ2*dQ6*m6*t2*t3*t9*t11*t35*2.0+Lxcm6*Lz6*dQ2*dQ6*m6*t2*t6*t8*t10*t34*2.0+Lxcm6*Lz6*dQ2*dQ6*m6*t3*t6*t7*t10*t34*2.0+Lxcm6*Lz6*dQ3*dQ5*m6*t2*t5*t8*t11*t34*2.0+Lxcm6*Lz6*dQ3*dQ5*m6*t3*t5*t7*t11*t34*2.0;
et202 = Lxcm6*Lz6*dQ1*dQ6*m6*t4*t6*t9*t10*t33*2.0+Lxcm6*Lz6*dQ3*dQ6*m6*t2*t3*t9*t11*t35*2.0+Lxcm6*Lz6*dQ3*dQ6*m6*t2*t6*t8*t10*t34*2.0+Lxcm6*Lz6*dQ3*dQ6*m6*t3*t6*t7*t10*t34*2.0-Lxcm6*Lz6*dQ4*dQ6*m6*t2*t4*t8*t11*t35*2.0-Lxcm6*Lz6*dQ4*dQ6*m6*t3*t4*t7*t11*t35*2.0-Lxcm6*Lz6*dQ2*dQ3*m6*t7*t8*t10*t11*t34*4.0-Lxcm6*Lz6*dQ2*dQ6*m6*t7*t8*t9*t11*t35*2.0-Lxcm6*Lz6*dQ3*dQ6*m6*t7*t8*t9*t11*t35*2.0-Lx4*Lzcm5*dQ1*dQ2*m5*t2*t7*t10*t33*t34*8.0-Lx4*Lzcm5*dQ1*dQ2*m5*t3*t8*t10*t32*t34*8.0-Lx4*Lzcm5*dQ1*dQ3*m5*t2*t7*t10*t33*t34*8.0-Lx4*Lzcm5*dQ1*dQ3*m5*t3*t8*t10*t32*t34*8.0-Lx4*Lzcm6*dQ1*dQ2*m6*t2*t7*t10*t33*t34*8.0-Lx4*Lzcm6*dQ1*dQ2*m6*t3*t8*t10*t32*t34*8.0;
et203 = Lx4*Lzcm6*dQ1*dQ3*m6*t2*t7*t10*t33*t34*-8.0-Lx4*Lzcm5*dQ1*dQ4*m5*t4*t9*t10*t32*t33*8.0-Lx4*Lzcm6*dQ1*dQ3*m6*t3*t8*t10*t32*t34*8.0-Lx4*Lzcm6*dQ1*dQ4*m6*t4*t9*t10*t32*t33*8.0-Lxcm6*Lz6*dQ1*dQ2*m6*t5*t9*t11*t32*t33*8.0-Lxcm6*Lz6*dQ1*dQ3*m6*t5*t9*t11*t32*t33*8.0-Lxcm6*Lz6*dQ1*dQ6*m6*t5*t10*t11*t32*t33*4.0+Lxcm6*Lz6*dQ1*dQ6*m6*t5*t10*t11*t32*t34*2.0+Lxcm6*Lz6*dQ1*dQ6*m6*t5*t10*t11*t33*t34*2.0+Lxcm6*Lz6*dQ1*dQ2*m6*t4*t6*t32*t33*t35*1.6e+1+Lxcm6*Lz6*dQ1*dQ3*m6*t4*t6*t32*t33*t35*1.6e+1-Lxcm6*Lz6*dQ1*dQ4*m6*t10*t11*t32*t33*t34*8.0+Lxcm6*Lz6*dQ1*dQ5*m6*t6*t32*t33*t34*t35*8.0-Lxcm4*Lzcm4*dQ1*dQ2*m4*t2*t3*t4*t7*t8*8.0;
et204 = Lxcm4*Lzcm4*dQ1*dQ3*m4*t2*t3*t4*t7*t8*-8.0+Lxcm5*Lzcm5*dQ1*dQ2*m5*t2*t3*t4*t7*t8*8.0+Lxcm5*Lzcm5*dQ1*dQ3*m5*t2*t3*t4*t7*t8*8.0+Lxcm5*Lzcm5*dQ1*dQ5*m5*t2*t4*t5*t7*t10*8.0+Lxcm6*Lzcm6*dQ1*dQ5*m6*t2*t3*t6*t7*t8*4.0+Lxcm5*Lzcm5*dQ1*dQ5*m5*t3*t4*t5*t8*t10*8.0+Lxcm5*Lzcm5*dQ2*dQ5*m5*t2*t3*t5*t9*t10*4.0+Lxcm6*Lzcm6*dQ1*dQ2*m6*t2*t5*t6*t7*t10*4.0+Lxcm5*Lzcm5*dQ3*dQ5*m5*t2*t3*t5*t9*t10*4.0+Lxcm6*Lzcm6*dQ1*dQ3*m6*t2*t5*t6*t7*t10*4.0+Lxcm6*Lzcm6*dQ1*dQ4*m6*t2*t4*t5*t7*t11*2.0-Lxcm5*Lzcm5*dQ4*dQ5*m5*t2*t4*t5*t8*t10*4.0-Lxcm5*Lzcm5*dQ4*dQ5*m5*t3*t4*t5*t7*t10*4.0+Lxcm6*Lzcm6*dQ1*dQ2*m6*t3*t5*t6*t8*t10*4.0+Lxcm6*Lzcm6*dQ2*dQ3*m6*t2*t4*t5*t8*t11*2.0+Lxcm6*Lzcm6*dQ2*dQ3*m6*t3*t4*t5*t7*t11*2.0;
et205 = Lxcm6*Lzcm6*dQ1*dQ3*m6*t3*t5*t6*t8*t10*4.0+Lxcm6*Lzcm6*dQ1*dQ4*m6*t3*t4*t5*t8*t11*2.0+Lxcm6*Lzcm6*dQ1*dQ6*m6*t2*t5*t6*t7*t9*2.0-Lxcm6*Lzcm6*dQ2*dQ5*m6*t2*t4*t6*t8*t9*2.0-Lxcm6*Lzcm6*dQ2*dQ5*m6*t3*t4*t6*t7*t9*2.0-Lxcm6*Lzcm6*dQ2*dQ4*m6*t2*t5*t6*t8*t10*4.0-Lxcm6*Lzcm6*dQ2*dQ4*m6*t3*t5*t6*t7*t10*4.0+Lxcm6*Lzcm6*dQ2*dQ5*m6*t2*t3*t4*t10*t11*2.0-Lxcm6*Lzcm6*dQ3*dQ5*m6*t2*t4*t6*t8*t9*2.0-Lxcm6*Lzcm6*dQ3*dQ5*m6*t3*t4*t6*t7*t9*2.0+Lxcm6*Lzcm6*dQ1*dQ6*m6*t3*t5*t6*t8*t9*2.0-Lxcm6*Lzcm6*dQ3*dQ4*m6*t2*t5*t6*t8*t10*4.0-Lxcm6*Lzcm6*dQ3*dQ4*m6*t3*t5*t6*t7*t10*4.0+Lxcm6*Lzcm6*dQ3*dQ5*m6*t2*t3*t4*t10*t11*2.0-Lxcm6*Lzcm6*dQ4*dQ6*m6*t2*t5*t6*t8*t9*2.0;
et206 = Lxcm6*Lzcm6*dQ4*dQ6*m6*t3*t5*t6*t7*t9*-2.0-Lxcm6*Lzcm6*dQ4*dQ6*m6*t2*t3*t5*t10*t11*2.0-Lxcm5*Lzcm5*dQ2*dQ5*m5*t5*t7*t8*t9*t10*4.0-Lxcm5*Lzcm5*dQ3*dQ5*m5*t5*t7*t8*t9*t10*4.0-Lxcm6*Lzcm6*dQ1*dQ5*m6*t2*t7*t9*t10*t11*2.0-Lxcm6*Lzcm6*dQ1*dQ5*m6*t3*t8*t9*t10*t11*2.0-Lxcm6*Lzcm6*dQ2*dQ5*m6*t4*t7*t8*t10*t11*2.0-Lxcm6*Lzcm6*dQ3*dQ5*m6*t4*t7*t8*t10*t11*2.0+Lxcm6*Lzcm6*dQ4*dQ6*m6*t5*t7*t8*t10*t11*2.0-Lxcm5*Lzcm5*dQ1*dQ2*m5*t2*t5*t7*t10*t33*8.0+Lxcm5*Lzcm5*dQ1*dQ5*m5*t2*t3*t7*t8*t34*4.0+Lxcm5*Lzcm5*dQ1*dQ2*m5*t2*t5*t7*t10*t34*4.0-Lxcm5*Lzcm5*dQ1*dQ2*m5*t3*t5*t8*t10*t32*8.0-Lxcm5*Lzcm5*dQ1*dQ3*m5*t2*t5*t7*t10*t33*8.0-Lxcm5*Lzcm5*dQ1*dQ5*m5*t2*t3*t7*t8*t35*8.0;
et207 = Lxcm5*Lzcm5*dQ1*dQ3*m5*t2*t5*t7*t10*t34*4.0-Lxcm5*Lzcm5*dQ1*dQ3*m5*t3*t5*t8*t10*t32*8.0+Lxcm5*Lzcm5*dQ1*dQ2*m5*t3*t5*t8*t10*t34*4.0+Lxcm5*Lzcm5*dQ1*dQ3*m5*t3*t5*t8*t10*t34*4.0+Lxcm5*Lzcm5*dQ1*dQ4*m5*t4*t5*t9*t10*t32*4.0+Lxcm5*Lzcm5*dQ2*dQ4*m5*t2*t5*t8*t10*t34*4.0+Lxcm5*Lzcm5*dQ2*dQ4*m5*t3*t5*t7*t10*t34*4.0+Lxcm6*Lzcm6*dQ1*dQ4*m6*t2*t6*t7*t9*t33*4.0+Lxcm5*Lzcm5*dQ1*dQ4*m5*t4*t5*t9*t10*t33*4.0+Lxcm5*Lzcm5*dQ3*dQ4*m5*t2*t5*t8*t10*t34*4.0+Lxcm5*Lzcm5*dQ3*dQ4*m5*t3*t5*t7*t10*t34*4.0+Lxcm6*Lzcm6*dQ1*dQ4*m6*t3*t6*t8*t9*t32*4.0+Lxcm6*Lzcm6*dQ1*dQ4*m6*t2*t6*t7*t9*t35*4.0+Lxcm6*Lzcm6*dQ1*dQ6*m6*t2*t4*t7*t11*t33*4.0+Lxcm6*Lzcm6*dQ1*dQ6*m6*t3*t4*t8*t11*t32*4.0+Lxcm6*Lzcm6*dQ2*dQ3*m6*t2*t3*t10*t11*t34*4.0;
et208 = Lxcm6*Lzcm6*dQ2*dQ3*m6*t2*t6*t8*t9*t35*4.0+Lxcm6*Lzcm6*dQ2*dQ3*m6*t3*t6*t7*t9*t35*4.0+Lxcm6*Lzcm6*dQ1*dQ4*m6*t3*t6*t8*t9*t35*4.0+Lxcm6*Lzcm6*dQ1*dQ6*m6*t2*t4*t7*t11*t35*4.0+Lxcm6*Lzcm6*dQ1*dQ5*m6*t4*t5*t9*t11*t32*2.0+Lxcm6*Lzcm6*dQ2*dQ5*m6*t2*t5*t8*t11*t34*2.0+Lxcm6*Lzcm6*dQ2*dQ5*m6*t3*t5*t7*t11*t34*2.0+Lxcm6*Lzcm6*dQ1*dQ5*m6*t4*t5*t9*t11*t33*2.0+Lxcm6*Lzcm6*dQ1*dQ6*m6*t3*t4*t8*t11*t35*4.0+Lxcm6*Lzcm6*dQ1*dQ6*m6*t4*t6*t9*t10*t32*2.0+Lxcm6*Lzcm6*dQ2*dQ6*m6*t2*t3*t9*t11*t35*2.0+Lxcm6*Lzcm6*dQ2*dQ6*m6*t2*t6*t8*t10*t34*2.0+Lxcm6*Lzcm6*dQ2*dQ6*m6*t3*t6*t7*t10*t34*2.0+Lxcm6*Lzcm6*dQ3*dQ5*m6*t2*t5*t8*t11*t34*2.0+Lxcm6*Lzcm6*dQ3*dQ5*m6*t3*t5*t7*t11*t34*2.0+Lxcm6*Lzcm6*dQ1*dQ6*m6*t4*t6*t9*t10*t33*2.0;
et209 = Lxcm6*Lzcm6*dQ3*dQ6*m6*t2*t3*t9*t11*t35*2.0+Lxcm6*Lzcm6*dQ3*dQ6*m6*t2*t6*t8*t10*t34*2.0+Lxcm6*Lzcm6*dQ3*dQ6*m6*t3*t6*t7*t10*t34*2.0-Lxcm6*Lzcm6*dQ4*dQ6*m6*t2*t4*t8*t11*t35*2.0-Lxcm6*Lzcm6*dQ4*dQ6*m6*t3*t4*t7*t11*t35*2.0-Lxcm6*Lzcm6*dQ2*dQ3*m6*t7*t8*t10*t11*t34*4.0-Lxcm6*Lzcm6*dQ2*dQ6*m6*t7*t8*t9*t11*t35*2.0-Lxcm6*Lzcm6*dQ3*dQ6*m6*t7*t8*t9*t11*t35*2.0-Lxcm5*Lzcm5*dQ1*dQ4*m5*t2*t7*t9*t33*t35*8.0-Lxcm5*Lzcm5*dQ1*dQ4*m5*t3*t8*t9*t32*t35*8.0-Lxcm6*Lzcm6*dQ1*dQ2*m6*t5*t9*t11*t32*t33*8.0-Lxcm6*Lzcm6*dQ1*dQ3*m6*t5*t9*t11*t32*t33*8.0-Lxcm6*Lzcm6*dQ1*dQ6*m6*t5*t10*t11*t32*t33*4.0+Lxcm6*Lzcm6*dQ1*dQ6*m6*t5*t10*t11*t32*t34*2.0+Lxcm6*Lzcm6*dQ1*dQ6*m6*t5*t10*t11*t33*t34*2.0;
et210 = Lxcm6*Lzcm6*dQ1*dQ2*m6*t4*t6*t32*t33*t35*1.6e+1+Lxcm6*Lzcm6*dQ1*dQ3*m6*t4*t6*t32*t33*t35*1.6e+1-Lxcm6*Lzcm6*dQ1*dQ4*m6*t10*t11*t32*t33*t34*8.0+Lxcm6*Lzcm6*dQ1*dQ5*m6*t6*t32*t33*t34*t35*8.0+Lycm6*Lz6*dQ1*dQ4*m6*t2*t4*t5*t6*t7*2.0+Lycm6*Lz6*dQ2*dQ3*m6*t2*t4*t5*t6*t8*2.0+Lycm6*Lz6*dQ2*dQ3*m6*t3*t4*t5*t6*t7*2.0+Lycm6*Lz6*dQ1*dQ4*m6*t3*t4*t5*t6*t8*2.0+Lycm6*Lz6*dQ2*dQ5*m6*t2*t3*t4*t6*t10*2.0+Lycm6*Lz6*dQ3*dQ5*m6*t2*t3*t4*t6*t10*2.0-Lycm6*Lz6*dQ4*dQ6*m6*t2*t3*t5*t6*t10*2.0-Lycm6*Lz6*dQ1*dQ5*m6*t2*t3*t7*t8*t11*4.0-Lycm6*Lz6*dQ1*dQ2*m6*t2*t5*t7*t10*t11*4.0-Lycm6*Lz6*dQ1*dQ3*m6*t2*t5*t7*t10*t11*4.0-Lycm6*Lz6*dQ1*dQ2*m6*t3*t5*t8*t10*t11*4.0;
et211 = Lycm6*Lz6*dQ1*dQ5*m6*t2*t6*t7*t9*t10*-2.0-Lycm6*Lz6*dQ1*dQ3*m6*t3*t5*t8*t10*t11*4.0-Lycm6*Lz6*dQ1*dQ6*m6*t2*t5*t7*t9*t11*2.0-Lycm6*Lz6*dQ1*dQ5*m6*t3*t6*t8*t9*t10*2.0+Lycm6*Lz6*dQ2*dQ4*m6*t2*t5*t8*t10*t11*4.0+Lycm6*Lz6*dQ2*dQ4*m6*t3*t5*t7*t10*t11*4.0-Lycm6*Lz6*dQ2*dQ5*m6*t4*t6*t7*t8*t10*2.0-Lycm6*Lz6*dQ1*dQ6*m6*t3*t5*t8*t9*t11*2.0+Lycm6*Lz6*dQ3*dQ4*m6*t2*t5*t8*t10*t11*4.0+Lycm6*Lz6*dQ3*dQ4*m6*t3*t5*t7*t10*t11*4.0-Lycm6*Lz6*dQ3*dQ5*m6*t4*t6*t7*t8*t10*2.0+Lycm6*Lz6*dQ4*dQ6*m6*t2*t5*t8*t9*t11*2.0+Lycm6*Lz6*dQ4*dQ6*m6*t3*t5*t7*t9*t11*2.0+Lycm6*Lz6*dQ4*dQ6*m6*t5*t6*t7*t8*t10*2.0+Lycm6*Lz6*dQ1*dQ6*m6*t2*t4*t6*t7*t33*4.0+Lycm6*Lz6*dQ1*dQ6*m6*t3*t4*t6*t8*t32*4.0;
et212 = Lycm6*Lz6*dQ2*dQ3*m6*t2*t3*t6*t10*t34*4.0+Lycm6*Lz6*dQ1*dQ6*m6*t2*t4*t6*t7*t35*4.0+Lycm6*Lz6*dQ1*dQ5*m6*t4*t5*t6*t9*t32*2.0+Lycm6*Lz6*dQ2*dQ5*m6*t2*t5*t6*t8*t34*2.0+Lycm6*Lz6*dQ2*dQ5*m6*t3*t5*t6*t7*t34*2.0+Lycm6*Lz6*dQ1*dQ5*m6*t4*t5*t6*t9*t33*2.0+Lycm6*Lz6*dQ1*dQ6*m6*t3*t4*t6*t8*t35*4.0+Lycm6*Lz6*dQ2*dQ6*m6*t2*t3*t6*t9*t35*2.0+Lycm6*Lz6*dQ3*dQ5*m6*t2*t5*t6*t8*t34*2.0+Lycm6*Lz6*dQ3*dQ5*m6*t3*t5*t6*t7*t34*2.0+Lycm6*Lz6*dQ3*dQ6*m6*t2*t3*t6*t9*t35*2.0-Lycm6*Lz6*dQ4*dQ6*m6*t2*t4*t6*t8*t35*2.0-Lycm6*Lz6*dQ4*dQ6*m6*t3*t4*t6*t7*t35*2.0-Lycm6*Lz6*dQ1*dQ4*m6*t2*t7*t9*t11*t33*4.0-Lycm6*Lz6*dQ1*dQ4*m6*t3*t8*t9*t11*t32*4.0-Lycm6*Lz6*dQ1*dQ4*m6*t2*t7*t9*t11*t35*4.0;
et213 = Lycm6*Lz6*dQ2*dQ3*m6*t2*t8*t9*t11*t35*-4.0-Lycm6*Lz6*dQ2*dQ3*m6*t3*t7*t9*t11*t35*4.0-Lycm6*Lz6*dQ2*dQ3*m6*t6*t7*t8*t10*t34*4.0-Lycm6*Lz6*dQ1*dQ4*m6*t3*t8*t9*t11*t35*4.0-Lycm6*Lz6*dQ1*dQ6*m6*t4*t9*t10*t11*t32*2.0-Lycm6*Lz6*dQ2*dQ6*m6*t2*t8*t10*t11*t34*2.0-Lycm6*Lz6*dQ2*dQ6*m6*t3*t7*t10*t11*t34*2.0-Lycm6*Lz6*dQ2*dQ6*m6*t6*t7*t8*t9*t35*2.0-Lycm6*Lz6*dQ1*dQ6*m6*t4*t9*t10*t11*t33*2.0-Lycm6*Lz6*dQ3*dQ6*m6*t2*t8*t10*t11*t34*2.0-Lycm6*Lz6*dQ3*dQ6*m6*t3*t7*t10*t11*t34*2.0-Lycm6*Lz6*dQ3*dQ6*m6*t6*t7*t8*t9*t35*2.0-Lycm6*Lz6*dQ1*dQ2*m6*t5*t6*t9*t32*t33*8.0-Lycm6*Lz6*dQ1*dQ3*m6*t5*t6*t9*t32*t33*8.0-Lycm6*Lz6*dQ1*dQ6*m6*t5*t6*t10*t32*t33*4.0;
et214 = Lycm6*Lz6*dQ1*dQ6*m6*t5*t6*t10*t32*t34*2.0+Lycm6*Lz6*dQ1*dQ6*m6*t5*t6*t10*t33*t34*2.0-Lycm6*Lz6*dQ1*dQ2*m6*t4*t11*t32*t33*t35*1.6e+1-Lycm6*Lz6*dQ1*dQ3*m6*t4*t11*t32*t33*t35*1.6e+1-Lycm6*Lz6*dQ1*dQ4*m6*t6*t10*t32*t33*t34*8.0-Lycm6*Lz6*dQ1*dQ5*m6*t11*t32*t33*t34*t35*8.0+Lycm4*Lzcm4*dQ1*dQ2*m4*t2*t3*t7*t8*t9*8.0+Lycm4*Lzcm4*dQ1*dQ3*m4*t2*t3*t7*t8*t9*8.0+Lycm6*Lzcm6*dQ1*dQ4*m6*t2*t4*t5*t6*t7*2.0+Lycm6*Lzcm6*dQ2*dQ3*m6*t2*t4*t5*t6*t8*2.0+Lycm6*Lzcm6*dQ2*dQ3*m6*t3*t4*t5*t6*t7*2.0+Lycm6*Lzcm6*dQ1*dQ4*m6*t3*t4*t5*t6*t8*2.0-Lycm5*Lzcm5*dQ1*dQ2*m5*t2*t4*t7*t9*t10*4.0-Lycm5*Lzcm5*dQ1*dQ4*m5*t2*t3*t7*t8*t10*4.0+Lycm6*Lzcm6*dQ2*dQ5*m6*t2*t3*t4*t6*t10*2.0;
et215 = Lycm5*Lzcm5*dQ1*dQ3*m5*t2*t4*t7*t9*t10*-4.0+Lycm6*Lzcm6*dQ3*dQ5*m6*t2*t3*t4*t6*t10*2.0-Lycm5*Lzcm5*dQ1*dQ2*m5*t3*t4*t8*t9*t10*4.0-Lycm5*Lzcm5*dQ1*dQ3*m5*t3*t4*t8*t9*t10*4.0-Lycm5*Lzcm5*dQ2*dQ4*m5*t2*t4*t8*t9*t10*4.0-Lycm5*Lzcm5*dQ2*dQ4*m5*t3*t4*t7*t9*t10*4.0-Lycm6*Lzcm6*dQ4*dQ6*m6*t2*t3*t5*t6*t10*2.0-Lycm5*Lzcm5*dQ3*dQ4*m5*t2*t4*t8*t9*t10*4.0-Lycm5*Lzcm5*dQ3*dQ4*m5*t3*t4*t7*t9*t10*4.0-Lycm6*Lzcm6*dQ1*dQ5*m6*t2*t3*t7*t8*t11*4.0-Lycm6*Lzcm6*dQ1*dQ2*m6*t2*t5*t7*t10*t11*4.0-Lycm6*Lzcm6*dQ1*dQ3*m6*t2*t5*t7*t10*t11*4.0-Lycm6*Lzcm6*dQ1*dQ2*m6*t3*t5*t8*t10*t11*4.0-Lycm6*Lzcm6*dQ1*dQ5*m6*t2*t6*t7*t9*t10*2.0-Lycm6*Lzcm6*dQ1*dQ3*m6*t3*t5*t8*t10*t11*4.0;
et216 = Lycm6*Lzcm6*dQ1*dQ6*m6*t2*t5*t7*t9*t11*-2.0-Lycm6*Lzcm6*dQ1*dQ5*m6*t3*t6*t8*t9*t10*2.0+Lycm6*Lzcm6*dQ2*dQ4*m6*t2*t5*t8*t10*t11*4.0+Lycm6*Lzcm6*dQ2*dQ4*m6*t3*t5*t7*t10*t11*4.0-Lycm6*Lzcm6*dQ2*dQ5*m6*t4*t6*t7*t8*t10*2.0-Lycm6*Lzcm6*dQ1*dQ6*m6*t3*t5*t8*t9*t11*2.0+Lycm6*Lzcm6*dQ3*dQ4*m6*t2*t5*t8*t10*t11*4.0+Lycm6*Lzcm6*dQ3*dQ4*m6*t3*t5*t7*t10*t11*4.0-Lycm6*Lzcm6*dQ3*dQ5*m6*t4*t6*t7*t8*t10*2.0+Lycm6*Lzcm6*dQ4*dQ6*m6*t2*t5*t8*t9*t11*2.0+Lycm6*Lzcm6*dQ4*dQ6*m6*t3*t5*t7*t9*t11*2.0+Lycm6*Lzcm6*dQ4*dQ6*m6*t5*t6*t7*t8*t10*2.0-Lycm5*Lzcm5*dQ1*dQ4*m5*t2*t4*t5*t7*t33*4.0-Lycm5*Lzcm5*dQ1*dQ4*m5*t3*t4*t5*t8*t32*4.0+Lycm6*Lzcm6*dQ1*dQ6*m6*t2*t4*t6*t7*t33*4.0+Lycm6*Lzcm6*dQ1*dQ6*m6*t3*t4*t6*t8*t32*4.0;
et217 = Lycm6*Lzcm6*dQ2*dQ3*m6*t2*t3*t6*t10*t34*4.0+Lycm6*Lzcm6*dQ1*dQ6*m6*t2*t4*t6*t7*t35*4.0+Lycm6*Lzcm6*dQ1*dQ5*m6*t4*t5*t6*t9*t32*2.0+Lycm6*Lzcm6*dQ2*dQ5*m6*t2*t5*t6*t8*t34*2.0+Lycm6*Lzcm6*dQ2*dQ5*m6*t3*t5*t6*t7*t34*2.0+Lycm6*Lzcm6*dQ1*dQ5*m6*t4*t5*t6*t9*t33*2.0+Lycm6*Lzcm6*dQ1*dQ6*m6*t3*t4*t6*t8*t35*4.0+Lycm6*Lzcm6*dQ2*dQ6*m6*t2*t3*t6*t9*t35*2.0+Lycm6*Lzcm6*dQ3*dQ5*m6*t2*t5*t6*t8*t34*2.0+Lycm6*Lzcm6*dQ3*dQ5*m6*t3*t5*t6*t7*t34*2.0+Lycm5*Lzcm5*dQ1*dQ5*m5*t2*t7*t9*t10*t33*4.0+Lycm6*Lzcm6*dQ3*dQ6*m6*t2*t3*t6*t9*t35*2.0+Lycm5*Lzcm5*dQ1*dQ5*m5*t3*t8*t9*t10*t32*4.0-Lycm6*Lzcm6*dQ4*dQ6*m6*t2*t4*t6*t8*t35*2.0-Lycm6*Lzcm6*dQ4*dQ6*m6*t3*t4*t6*t7*t35*2.0-Lycm6*Lzcm6*dQ1*dQ4*m6*t2*t7*t9*t11*t33*4.0;
et218 = Lycm6*Lzcm6*dQ1*dQ4*m6*t3*t8*t9*t11*t32*-4.0-Lycm6*Lzcm6*dQ1*dQ4*m6*t2*t7*t9*t11*t35*4.0-Lycm6*Lzcm6*dQ2*dQ3*m6*t2*t8*t9*t11*t35*4.0-Lycm6*Lzcm6*dQ2*dQ3*m6*t3*t7*t9*t11*t35*4.0-Lycm6*Lzcm6*dQ2*dQ3*m6*t6*t7*t8*t10*t34*4.0-Lycm6*Lzcm6*dQ1*dQ4*m6*t3*t8*t9*t11*t35*4.0-Lycm6*Lzcm6*dQ1*dQ6*m6*t4*t9*t10*t11*t32*2.0-Lycm6*Lzcm6*dQ2*dQ6*m6*t2*t8*t10*t11*t34*2.0-Lycm6*Lzcm6*dQ2*dQ6*m6*t3*t7*t10*t11*t34*2.0-Lycm6*Lzcm6*dQ2*dQ6*m6*t6*t7*t8*t9*t35*2.0-Lycm6*Lzcm6*dQ1*dQ6*m6*t4*t9*t10*t11*t33*2.0-Lycm6*Lzcm6*dQ3*dQ6*m6*t2*t8*t10*t11*t34*2.0-Lycm6*Lzcm6*dQ3*dQ6*m6*t3*t7*t10*t11*t34*2.0-Lycm6*Lzcm6*dQ3*dQ6*m6*t6*t7*t8*t9*t35*2.0-Lycm5*Lzcm5*dQ1*dQ5*m5*t4*t5*t9*t32*t33*4.0;
et219 = Lycm6*Lzcm6*dQ1*dQ2*m6*t5*t6*t9*t32*t33*-8.0-Lycm6*Lzcm6*dQ1*dQ3*m6*t5*t6*t9*t32*t33*8.0-Lycm6*Lzcm6*dQ1*dQ6*m6*t5*t6*t10*t32*t33*4.0+Lycm6*Lzcm6*dQ1*dQ6*m6*t5*t6*t10*t32*t34*2.0+Lycm6*Lzcm6*dQ1*dQ6*m6*t5*t6*t10*t33*t34*2.0-Lycm6*Lzcm6*dQ1*dQ2*m6*t4*t11*t32*t33*t35*1.6e+1-Lycm6*Lzcm6*dQ1*dQ3*m6*t4*t11*t32*t33*t35*1.6e+1-Lycm6*Lzcm6*dQ1*dQ4*m6*t6*t10*t32*t33*t34*8.0-Lycm6*Lzcm6*dQ1*dQ5*m6*t11*t32*t33*t34*t35*8.0+Lz6*Lzcm6*dQ1*dQ4*m6*t2*t5*t7*t9*t10*4.0+Lz6*Lzcm6*dQ2*dQ3*m6*t2*t5*t8*t9*t10*4.0+Lz6*Lzcm6*dQ2*dQ3*m6*t3*t5*t7*t9*t10*4.0+Lz6*Lzcm6*dQ1*dQ4*m6*t3*t5*t8*t9*t10*4.0-Lz6*Lzcm6*dQ2*dQ3*m6*t2*t3*t4*t9*t35*4.0+Lz6*Lzcm6*dQ2*dQ3*m6*t4*t7*t8*t9*t35*4.0;
et220 = Lz6*Lzcm6*dQ1*dQ2*m6*t4*t5*t10*t32*t33*1.6e+1+Lz6*Lzcm6*dQ1*dQ5*m6*t2*t4*t7*t33*t35*1.6e+1+Lz6*Lzcm6*dQ1*dQ3*m6*t4*t5*t10*t32*t33*1.6e+1+Lz6*Lzcm6*dQ1*dQ5*m6*t3*t4*t8*t32*t35*1.6e+1+Lz6*Lzcm6*dQ1*dQ2*m6*t2*t7*t33*t34*t35*8.0+Lz6*Lzcm6*dQ1*dQ2*m6*t3*t8*t32*t34*t35*8.0+Lz6*Lzcm6*dQ1*dQ3*m6*t2*t7*t33*t34*t35*8.0+Lz6*Lzcm6*dQ1*dQ3*m6*t3*t8*t32*t34*t35*8.0+Lz6*Lzcm6*dQ1*dQ4*m6*t4*t9*t32*t33*t35*8.0+Lz6*Lzcm6*dQ1*dQ5*m6*t5*t10*t32*t33*t34*8.0-Ixx5*dQ1*dQ2*t2*t3*t4*t5*t7*t8*t10*8.0-Ixx5*dQ1*dQ3*t2*t3*t4*t5*t7*t8*t10*8.0+Ixx6*dQ1*dQ2*t2*t4*t5*t6*t7*t9*t11*4.0+Ixx6*dQ1*dQ3*t2*t4*t5*t6*t7*t9*t11*4.0+Ixx6*dQ1*dQ2*t3*t4*t5*t6*t8*t9*t11*4.0;
et221 = Ixx6*dQ1*dQ3*t3*t4*t5*t6*t8*t9*t11*4.0+Ixx6*dQ2*dQ4*t2*t4*t5*t6*t8*t9*t11*4.0+Ixx6*dQ2*dQ4*t3*t4*t5*t6*t7*t9*t11*4.0+Ixx6*dQ1*dQ6*t2*t4*t5*t6*t7*t10*t11*4.0+Ixx6*dQ3*dQ4*t2*t4*t5*t6*t8*t9*t11*4.0+Ixx6*dQ3*dQ4*t3*t4*t5*t6*t7*t9*t11*4.0+Ixx6*dQ1*dQ6*t3*t4*t5*t6*t8*t10*t11*4.0+Ixx6*dQ2*dQ6*t2*t3*t5*t6*t9*t10*t11*2.0+Ixx6*dQ3*dQ6*t2*t3*t5*t6*t9*t10*t11*2.0-Ixx6*dQ2*dQ6*t5*t6*t7*t8*t9*t10*t11*2.0-Ixx6*dQ3*dQ6*t5*t6*t7*t8*t9*t10*t11*2.0-Ixx5*dQ1*dQ5*t2*t3*t5*t7*t8*t10*t34*4.0-Ixx6*dQ1*dQ5*t2*t3*t5*t7*t8*t10*t36*4.0-Ixx6*dQ1*dQ4*t2*t4*t6*t7*t10*t11*t33*4.0-Ixx6*dQ1*dQ6*t2*t3*t6*t7*t8*t11*t34*4.0-Ixx6*dQ1*dQ4*t3*t4*t6*t8*t10*t11*t32*4.0;
et222 = Ixx6*dQ1*dQ5*t2*t5*t6*t7*t9*t11*t33*-4.0-Ixx6*dQ1*dQ6*t2*t3*t6*t7*t8*t11*t35*4.0-Ixx6*dQ1*dQ5*t3*t5*t6*t8*t9*t11*t32*4.0-Ixx6*dQ1*dQ4*t2*t5*t7*t9*t10*t33*t36*4.0-Ixx6*dQ1*dQ4*t3*t5*t8*t9*t10*t32*t36*4.0-Ixx6*dQ1*dQ5*t4*t6*t9*t10*t11*t32*t33*4.0-Iyy6*dQ1*dQ2*t2*t3*t4*t5*t7*t8*t10*8.0-Iyy6*dQ1*dQ3*t2*t3*t4*t5*t7*t8*t10*8.0-Iyy6*dQ1*dQ2*t2*t4*t5*t6*t7*t9*t11*4.0-Iyy6*dQ1*dQ3*t2*t4*t5*t6*t7*t9*t11*4.0-Iyy6*dQ1*dQ2*t3*t4*t5*t6*t8*t9*t11*4.0-Iyy6*dQ1*dQ3*t3*t4*t5*t6*t8*t9*t11*4.0-Iyy6*dQ2*dQ4*t2*t4*t5*t6*t8*t9*t11*4.0-Iyy6*dQ2*dQ4*t3*t4*t5*t6*t7*t9*t11*4.0-Iyy6*dQ1*dQ6*t2*t4*t5*t6*t7*t10*t11*4.0;
et223 = Iyy6*dQ3*dQ4*t2*t4*t5*t6*t8*t9*t11*-4.0-Iyy6*dQ3*dQ4*t3*t4*t5*t6*t7*t9*t11*4.0-Iyy6*dQ1*dQ6*t3*t4*t5*t6*t8*t10*t11*4.0-Iyy6*dQ2*dQ6*t2*t3*t5*t6*t9*t10*t11*2.0-Iyy6*dQ3*dQ6*t2*t3*t5*t6*t9*t10*t11*2.0+Iyy6*dQ2*dQ6*t5*t6*t7*t8*t9*t10*t11*2.0+Iyy6*dQ3*dQ6*t5*t6*t7*t8*t9*t10*t11*2.0-Iyy6*dQ1*dQ5*t2*t3*t5*t7*t8*t10*t34*4.0+Iyy6*dQ1*dQ5*t2*t3*t5*t7*t8*t10*t36*4.0+Iyy6*dQ1*dQ4*t2*t4*t6*t7*t10*t11*t33*4.0+Iyy6*dQ1*dQ6*t2*t3*t6*t7*t8*t11*t34*4.0+Iyy6*dQ1*dQ4*t3*t4*t6*t8*t10*t11*t32*4.0+Iyy6*dQ1*dQ5*t2*t5*t6*t7*t9*t11*t33*4.0+Iyy6*dQ1*dQ6*t2*t3*t6*t7*t8*t11*t35*4.0+Iyy6*dQ1*dQ5*t3*t5*t6*t8*t9*t11*t32*4.0-Iyy6*dQ2*dQ5*t2*t4*t5*t8*t9*t10*t36*2.0;
et224 = Iyy6*dQ2*dQ5*t3*t4*t5*t7*t9*t10*t36*-2.0-Iyy6*dQ3*dQ5*t2*t4*t5*t8*t9*t10*t36*2.0-Iyy6*dQ3*dQ5*t3*t4*t5*t7*t9*t10*t36*2.0-Iyy6*dQ2*dQ6*t2*t4*t6*t8*t9*t11*t35*2.0-Iyy6*dQ2*dQ6*t3*t4*t6*t7*t9*t11*t35*2.0-Iyy6*dQ3*dQ6*t2*t4*t6*t8*t9*t11*t35*2.0-Iyy6*dQ3*dQ6*t3*t4*t6*t7*t9*t11*t35*2.0+Iyy6*dQ1*dQ4*t2*t5*t7*t9*t10*t33*t36*4.0+Iyy6*dQ1*dQ4*t3*t5*t8*t9*t10*t32*t36*4.0+Iyy6*dQ1*dQ5*t4*t6*t9*t10*t11*t32*t33*4.0+Izz5*dQ1*dQ2*t2*t3*t4*t5*t7*t8*t10*8.0+Izz5*dQ1*dQ3*t2*t3*t4*t5*t7*t8*t10*8.0+Izz6*dQ1*dQ2*t2*t3*t4*t5*t7*t8*t10*8.0+Izz6*dQ1*dQ3*t2*t3*t4*t5*t7*t8*t10*8.0+Izz5*dQ1*dQ5*t2*t3*t5*t7*t8*t10*t34*4.0;
et225 = Izz6*dQ1*dQ5*t2*t3*t5*t7*t8*t10*t34*4.0+dQ1*dQ4*m4*t2*t3*t4*t7*t8*t9*t14*4.0+dQ1*dQ4*m5*t2*t3*t4*t7*t8*t9*t14*4.0+dQ1*dQ4*m4*t2*t3*t4*t7*t8*t9*t16*4.0+dQ1*dQ4*m6*t2*t3*t4*t7*t8*t9*t14*4.0-dQ1*dQ4*m4*t2*t3*t4*t7*t8*t9*t19*4.0-dQ1*dQ4*m6*t2*t3*t4*t7*t8*t9*t18*4.0+dQ2*dQ5*m6*t2*t3*t4*t5*t6*t11*t18*2.0-dQ1*dQ4*m5*t2*t3*t4*t7*t8*t9*t20*4.0+dQ1*dQ5*m5*t2*t3*t5*t7*t8*t10*t17*4.0+dQ3*dQ5*m6*t2*t3*t4*t5*t6*t11*t18*2.0-dQ2*dQ5*m6*t2*t3*t4*t5*t6*t11*t21*2.0+dQ1*dQ4*m6*t2*t3*t4*t7*t8*t9*t22*4.0-dQ3*dQ5*m6*t2*t3*t4*t5*t6*t11*t21*2.0-dQ2*dQ5*m5*t2*t4*t5*t8*t9*t10*t17*2.0-dQ2*dQ5*m5*t3*t4*t5*t7*t9*t10*t17*2.0;
et226 = dQ1*dQ4*m5*t2*t3*t4*t7*t8*t9*t25*4.0+dQ1*dQ5*m6*t2*t3*t5*t7*t8*t10*t21*4.0-dQ1*dQ6*m6*t2*t3*t6*t7*t8*t11*t18*8.0-dQ3*dQ5*m5*t2*t4*t5*t8*t9*t10*t17*2.0-dQ3*dQ5*m5*t3*t4*t5*t7*t9*t10*t17*2.0-dQ1*dQ4*m6*t2*t4*t6*t7*t10*t11*t18*2.0-dQ1*dQ5*m6*t2*t3*t5*t7*t8*t10*t22*4.0+dQ1*dQ4*m6*t2*t3*t4*t7*t8*t9*t26*4.0-dQ1*dQ5*m6*t2*t5*t6*t7*t9*t11*t18*2.0-dQ2*dQ3*m6*t2*t4*t6*t8*t10*t11*t18*2.0-dQ2*dQ3*m6*t3*t4*t6*t7*t10*t11*t18*2.0-dQ1*dQ4*m6*t3*t4*t6*t8*t10*t11*t18*2.0-dQ1*dQ5*m5*t2*t3*t5*t7*t8*t10*t25*4.0+dQ1*dQ6*m6*t2*t3*t6*t7*t8*t11*t21*8.0+dQ1*dQ4*m6*t2*t4*t6*t7*t10*t11*t21*2.0;
et227 = dQ1*dQ5*m6*t3*t5*t6*t8*t9*t11*t18*-2.0-dQ2*dQ5*m6*t2*t4*t5*t8*t9*t10*t21*2.0-dQ2*dQ5*m6*t3*t4*t5*t7*t9*t10*t21*2.0-dQ2*dQ5*m6*t4*t5*t6*t7*t8*t11*t18*2.0-dQ2*dQ6*m6*t2*t4*t6*t8*t9*t11*t18*2.0-dQ2*dQ6*m6*t3*t4*t6*t7*t9*t11*t18*2.0-dQ1*dQ5*m6*t2*t3*t5*t7*t8*t10*t26*4.0+dQ1*dQ5*m6*t2*t5*t6*t7*t9*t11*t21*2.0+dQ2*dQ3*m6*t2*t4*t6*t8*t10*t11*t21*2.0+dQ2*dQ3*m6*t3*t4*t6*t7*t10*t11*t21*2.0+dQ2*dQ5*m6*t2*t4*t5*t8*t9*t10*t22*2.0+dQ2*dQ5*m6*t3*t4*t5*t7*t9*t10*t22*2.0-dQ3*dQ5*m6*t2*t4*t5*t8*t9*t10*t21*2.0-dQ3*dQ5*m6*t3*t4*t5*t7*t9*t10*t21*2.0-dQ3*dQ5*m6*t4*t5*t6*t7*t8*t11*t18*2.0;
et228 = dQ3*dQ6*m6*t2*t4*t6*t8*t9*t11*t18*-2.0-dQ3*dQ6*m6*t3*t4*t6*t7*t9*t11*t18*2.0+dQ1*dQ4*m6*t3*t4*t6*t8*t10*t11*t21*2.0+dQ3*dQ5*m6*t2*t4*t5*t8*t9*t10*t22*2.0+dQ3*dQ5*m6*t3*t4*t5*t7*t9*t10*t22*2.0+dQ1*dQ5*m6*t3*t5*t6*t8*t9*t11*t21*2.0+dQ2*dQ5*m5*t2*t4*t5*t8*t9*t10*t25*2.0+dQ2*dQ5*m5*t3*t4*t5*t7*t9*t10*t25*2.0+dQ2*dQ5*m6*t4*t5*t6*t7*t8*t11*t21*2.0+dQ2*dQ6*m6*t2*t4*t6*t8*t9*t11*t21*2.0+dQ2*dQ6*m6*t3*t4*t6*t7*t9*t11*t21*2.0+dQ3*dQ5*m5*t2*t4*t5*t8*t9*t10*t25*2.0+dQ3*dQ5*m5*t3*t4*t5*t7*t9*t10*t25*2.0+dQ3*dQ5*m6*t4*t5*t6*t7*t8*t11*t21*2.0+dQ3*dQ6*m6*t2*t4*t6*t8*t9*t11*t21*2.0+dQ3*dQ6*m6*t3*t4*t6*t7*t9*t11*t21*2.0;
et229 = dQ2*dQ5*m6*t2*t4*t5*t8*t9*t10*t26*2.0+dQ2*dQ5*m6*t3*t4*t5*t7*t9*t10*t26*2.0+dQ3*dQ5*m6*t2*t4*t5*t8*t9*t10*t26*2.0+dQ3*dQ5*m6*t3*t4*t5*t7*t9*t10*t26*2.0+dQ2*dQ3*m6*t2*t3*t5*t6*t11*t18*t34*4.0+dQ1*dQ4*m5*t2*t5*t7*t9*t10*t17*t33*4.0-dQ2*dQ3*m6*t2*t3*t5*t6*t11*t21*t34*4.0+dQ1*dQ4*m5*t3*t5*t8*t9*t10*t17*t32*4.0-dQ1*dQ4*m6*t2*t5*t7*t9*t10*t18*t36*2.0+dQ1*dQ4*m6*t2*t5*t7*t9*t10*t21*t33*4.0-dQ1*dQ4*m6*t2*t5*t7*t9*t10*t22*t33*4.0+dQ1*dQ4*m6*t3*t5*t8*t9*t10*t21*t32*4.0-dQ2*dQ3*m6*t2*t5*t8*t9*t10*t18*t36*2.0-dQ2*dQ3*m6*t3*t5*t7*t9*t10*t18*t36*2.0-dQ1*dQ4*m6*t3*t5*t8*t9*t10*t18*t36*2.0-dQ1*dQ4*m6*t3*t5*t8*t9*t10*t22*t32*4.0;
et230 = dQ2*dQ3*m6*t5*t6*t7*t8*t11*t18*t34*-4.0-dQ1*dQ4*m5*t2*t5*t7*t9*t10*t25*t33*4.0+dQ1*dQ4*m6*t2*t5*t7*t9*t10*t21*t36*2.0-dQ1*dQ4*m5*t3*t5*t8*t9*t10*t25*t32*4.0-dQ1*dQ5*m6*t4*t6*t9*t10*t11*t18*t32*2.0+dQ2*dQ3*m6*t2*t5*t8*t9*t10*t21*t36*2.0+dQ2*dQ3*m6*t3*t5*t7*t9*t10*t21*t36*2.0-dQ2*dQ5*m6*t2*t6*t8*t10*t11*t18*t34*2.0-dQ2*dQ5*m6*t3*t6*t7*t10*t11*t18*t34*2.0-dQ1*dQ4*m6*t2*t5*t7*t9*t10*t26*t33*4.0+dQ1*dQ4*m6*t3*t5*t8*t9*t10*t21*t36*2.0-dQ1*dQ5*m6*t4*t6*t9*t10*t11*t18*t33*2.0+dQ2*dQ3*m6*t5*t6*t7*t8*t11*t21*t34*4.0-dQ3*dQ5*m6*t2*t6*t8*t10*t11*t18*t34*2.0-dQ3*dQ5*m6*t3*t6*t7*t10*t11*t18*t34*2.0;
et231 = dQ1*dQ4*m6*t3*t5*t8*t9*t10*t26*t32*-4.0+dQ1*dQ5*m6*t4*t6*t9*t10*t11*t21*t32*2.0+dQ2*dQ5*m6*t2*t6*t8*t10*t11*t21*t34*2.0+dQ2*dQ5*m6*t3*t6*t7*t10*t11*t21*t34*2.0+dQ1*dQ5*m6*t4*t6*t9*t10*t11*t21*t33*2.0+dQ3*dQ5*m6*t2*t6*t8*t10*t11*t21*t34*2.0+dQ3*dQ5*m6*t3*t6*t7*t10*t11*t21*t34*2.0+dQ2*dQ3*m6*t2*t3*t4*t9*t18*t35*t36*2.0-dQ2*dQ3*m6*t2*t3*t4*t9*t21*t35*t36*2.0+dQ1*dQ2*m6*t6*t9*t10*t11*t18*t32*t33*8.0+dQ1*dQ6*m6*t2*t7*t9*t10*t18*t33*t36*8.0-dQ2*dQ3*m6*t4*t7*t8*t9*t18*t35*t36*2.0+dQ1*dQ3*m6*t6*t9*t10*t11*t18*t32*t33*8.0+dQ1*dQ6*m6*t3*t8*t9*t10*t18*t32*t36*8.0-dQ1*dQ2*m6*t6*t9*t10*t11*t21*t32*t33*8.0;
et232 = dQ1*dQ6*m6*t2*t7*t9*t10*t21*t33*t36*-8.0+dQ2*dQ3*m6*t4*t7*t8*t9*t21*t35*t36*2.0-dQ1*dQ3*m6*t6*t9*t10*t11*t21*t32*t33*8.0-dQ1*dQ6*m6*t3*t8*t9*t10*t21*t32*t36*8.0-dQ1*dQ2*m6*t4*t5*t10*t18*t32*t33*t36*8.0-dQ1*dQ5*m6*t2*t4*t7*t18*t33*t35*t36*8.0-dQ1*dQ3*m6*t4*t5*t10*t18*t32*t33*t36*8.0-dQ1*dQ5*m6*t3*t4*t8*t18*t32*t35*t36*8.0+dQ1*dQ2*m6*t4*t5*t10*t21*t32*t33*t36*8.0-dQ1*dQ4*m6*t5*t6*t11*t18*t32*t33*t34*8.0+dQ1*dQ5*m6*t2*t4*t7*t21*t33*t35*t36*8.0-dQ1*dQ6*m6*t4*t5*t9*t18*t32*t33*t36*8.0+dQ1*dQ3*m6*t4*t5*t10*t21*t32*t33*t36*8.0+dQ1*dQ5*m6*t3*t4*t8*t21*t32*t35*t36*8.0;
et233 = dQ1*dQ4*m6*t5*t6*t11*t21*t32*t33*t34*8.0+dQ1*dQ6*m6*t4*t5*t9*t21*t32*t33*t36*8.0-dQ1*dQ2*m6*t2*t7*t18*t33*t34*t35*t36*4.0-dQ1*dQ2*m6*t3*t8*t18*t32*t34*t35*t36*4.0-dQ1*dQ3*m6*t2*t7*t18*t33*t34*t35*t36*4.0-dQ1*dQ3*m6*t3*t8*t18*t32*t34*t35*t36*4.0+dQ1*dQ2*m6*t2*t7*t21*t33*t34*t35*t36*4.0+dQ1*dQ2*m6*t3*t8*t21*t32*t34*t35*t36*4.0+dQ1*dQ3*m6*t2*t7*t21*t33*t34*t35*t36*4.0-dQ1*dQ4*m6*t4*t9*t18*t32*t33*t35*t36*4.0+dQ1*dQ3*m6*t3*t8*t21*t32*t34*t35*t36*4.0-dQ1*dQ5*m6*t5*t10*t18*t32*t33*t34*t36*4.0+dQ1*dQ4*m6*t4*t9*t21*t32*t33*t35*t36*4.0-dQ1*dQ6*m6*t6*t11*t18*t32*t33*t34*t35*4.0+dQ1*dQ5*m6*t5*t10*t21*t32*t33*t34*t36*4.0;
et234 = dQ1*dQ6*m6*t6*t11*t21*t32*t33*t34*t35*4.0+Ixx6*dQ1*dQ2*t2*t3*t6*t7*t8*t9*t10*t11*8.0+Ixx6*dQ1*dQ3*t2*t3*t6*t7*t8*t9*t10*t11*8.0-Ixx6*dQ1*dQ2*t2*t3*t4*t5*t7*t8*t10*t36*8.0-Ixx6*dQ1*dQ3*t2*t3*t4*t5*t7*t8*t10*t36*8.0-Ixx6*dQ1*dQ2*t2*t4*t5*t6*t7*t9*t11*t33*8.0-Ixx6*dQ1*dQ2*t3*t4*t5*t6*t8*t9*t11*t32*8.0-Ixx6*dQ1*dQ3*t2*t4*t5*t6*t7*t9*t11*t33*8.0-Ixx6*dQ1*dQ3*t3*t4*t5*t6*t8*t9*t11*t32*8.0-Ixx6*dQ1*dQ6*t2*t4*t5*t6*t7*t10*t11*t33*8.0-Ixx6*dQ1*dQ6*t3*t4*t5*t6*t8*t10*t11*t32*8.0-Ixx6*dQ1*dQ5*t2*t3*t5*t7*t8*t10*t34*t36*4.0-Ixx6*dQ1*dQ6*t2*t3*t6*t7*t8*t11*t34*t35*4.0;
et235 = Iyy6*dQ1*dQ2*t2*t3*t6*t7*t8*t9*t10*t11*-8.0-Iyy6*dQ1*dQ3*t2*t3*t6*t7*t8*t9*t10*t11*8.0+Iyy6*dQ1*dQ2*t2*t3*t4*t5*t7*t8*t10*t36*8.0+Iyy6*dQ1*dQ3*t2*t3*t4*t5*t7*t8*t10*t36*8.0+Iyy6*dQ1*dQ2*t2*t4*t5*t6*t7*t9*t11*t33*8.0+Iyy6*dQ1*dQ2*t3*t4*t5*t6*t8*t9*t11*t32*8.0+Iyy6*dQ1*dQ3*t2*t4*t5*t6*t7*t9*t11*t33*8.0+Iyy6*dQ1*dQ3*t3*t4*t5*t6*t8*t9*t11*t32*8.0+Iyy6*dQ1*dQ6*t2*t4*t5*t6*t7*t10*t11*t33*8.0+Iyy6*dQ1*dQ6*t3*t4*t5*t6*t8*t10*t11*t32*8.0+Iyy6*dQ1*dQ5*t2*t3*t5*t7*t8*t10*t34*t36*4.0+Iyy6*dQ1*dQ6*t2*t3*t6*t7*t8*t11*t34*t35*4.0+dQ1*dQ2*m5*t2*t3*t4*t5*t7*t8*t10*t17*8.0+dQ1*dQ3*m5*t2*t3*t4*t5*t7*t8*t10*t17*8.0;
et236 = dQ1*dQ2*m6*t2*t3*t4*t5*t7*t8*t10*t21*8.0-dQ1*dQ6*m6*t2*t3*t4*t5*t7*t8*t9*t18*4.0-dQ1*dQ2*m6*t2*t3*t4*t5*t7*t8*t10*t22*8.0+dQ1*dQ3*m6*t2*t3*t4*t5*t7*t8*t10*t21*8.0-dQ1*dQ2*m6*t2*t4*t5*t6*t7*t9*t11*t18*4.0-dQ1*dQ3*m6*t2*t3*t4*t5*t7*t8*t10*t22*8.0-dQ1*dQ4*m6*t2*t3*t5*t6*t7*t8*t11*t18*4.0-dQ1*dQ2*m5*t2*t3*t4*t5*t7*t8*t10*t25*8.0-dQ1*dQ3*m6*t2*t4*t5*t6*t7*t9*t11*t18*4.0+dQ1*dQ6*m6*t2*t3*t4*t5*t7*t8*t9*t21*4.0-dQ1*dQ2*m6*t3*t4*t5*t6*t8*t9*t11*t18*4.0-dQ1*dQ3*m5*t2*t3*t4*t5*t7*t8*t10*t25*8.0-dQ1*dQ2*m6*t2*t3*t4*t5*t7*t8*t10*t26*8.0+dQ1*dQ2*m6*t2*t4*t5*t6*t7*t9*t11*t21*4.0;
et237 = dQ1*dQ3*m6*t3*t4*t5*t6*t8*t9*t11*t18*-4.0+dQ1*dQ4*m6*t2*t3*t5*t6*t7*t8*t11*t21*4.0-dQ1*dQ3*m6*t2*t3*t4*t5*t7*t8*t10*t26*8.0+dQ1*dQ3*m6*t2*t4*t5*t6*t7*t9*t11*t21*4.0-dQ2*dQ4*m6*t2*t4*t5*t6*t8*t9*t11*t18*4.0-dQ2*dQ4*m6*t3*t4*t5*t6*t7*t9*t11*t18*4.0+dQ1*dQ2*m6*t3*t4*t5*t6*t8*t9*t11*t21*4.0-dQ1*dQ6*m6*t2*t4*t5*t6*t7*t10*t11*t18*4.0-dQ3*dQ4*m6*t2*t4*t5*t6*t8*t9*t11*t18*4.0-dQ3*dQ4*m6*t3*t4*t5*t6*t7*t9*t11*t18*4.0+dQ1*dQ3*m6*t3*t4*t5*t6*t8*t9*t11*t21*4.0-dQ1*dQ6*m6*t3*t4*t5*t6*t8*t10*t11*t18*4.0+dQ2*dQ4*m6*t2*t4*t5*t6*t8*t9*t11*t21*4.0+dQ2*dQ4*m6*t3*t4*t5*t6*t7*t9*t11*t21*4.0;
et238 = dQ2*dQ6*m6*t2*t3*t5*t6*t9*t10*t11*t18*-2.0+dQ1*dQ6*m6*t2*t4*t5*t6*t7*t10*t11*t21*4.0+dQ3*dQ4*m6*t2*t4*t5*t6*t8*t9*t11*t21*4.0+dQ3*dQ4*m6*t3*t4*t5*t6*t7*t9*t11*t21*4.0-dQ3*dQ6*m6*t2*t3*t5*t6*t9*t10*t11*t18*2.0+dQ4*dQ6*m6*t2*t4*t5*t6*t8*t10*t11*t18*2.0+dQ4*dQ6*m6*t3*t4*t5*t6*t7*t10*t11*t18*2.0+dQ1*dQ6*m6*t3*t4*t5*t6*t8*t10*t11*t21*4.0+dQ2*dQ6*m6*t2*t3*t5*t6*t9*t10*t11*t21*2.0+dQ3*dQ6*m6*t2*t3*t5*t6*t9*t10*t11*t21*2.0-dQ4*dQ6*m6*t2*t4*t5*t6*t8*t10*t11*t21*2.0-dQ4*dQ6*m6*t3*t4*t5*t6*t7*t10*t11*t21*2.0+dQ2*dQ6*m6*t5*t6*t7*t8*t9*t10*t11*t18*2.0+dQ3*dQ6*m6*t5*t6*t7*t8*t9*t10*t11*t18*2.0-dQ2*dQ6*m6*t5*t6*t7*t8*t9*t10*t11*t21*2.0;
et239 = dQ3*dQ6*m6*t5*t6*t7*t8*t9*t10*t11*t21*-2.0+dQ1*dQ4*m5*t2*t3*t4*t7*t8*t9*t17*t35*4.0+dQ1*dQ5*m5*t2*t3*t5*t7*t8*t10*t17*t34*4.0+dQ1*dQ4*m6*t2*t3*t4*t7*t8*t9*t18*t36*4.0+dQ1*dQ4*m6*t2*t3*t4*t7*t8*t9*t21*t35*4.0-dQ1*dQ4*m6*t2*t3*t4*t7*t8*t9*t21*t36*4.0-dQ1*dQ4*m6*t2*t3*t4*t7*t8*t9*t22*t35*4.0+dQ1*dQ5*m6*t2*t3*t5*t7*t8*t10*t18*t36*4.0+dQ1*dQ4*m6*t2*t4*t6*t7*t10*t11*t18*t33*4.0+dQ1*dQ5*m6*t2*t3*t5*t7*t8*t10*t21*t34*4.0+dQ1*dQ6*m6*t2*t3*t6*t7*t8*t11*t18*t34*4.0-dQ1*dQ4*m5*t2*t3*t4*t7*t8*t9*t25*t35*4.0+dQ1*dQ4*m6*t3*t4*t6*t8*t10*t11*t18*t32*4.0-dQ1*dQ5*m6*t2*t3*t5*t7*t8*t10*t22*t34*4.0+dQ1*dQ5*m6*t2*t5*t6*t7*t9*t11*t18*t33*4.0;
et240 = dQ1*dQ6*m6*t2*t3*t6*t7*t8*t11*t18*t35*4.0-dQ1*dQ5*m6*t2*t3*t5*t7*t8*t10*t21*t36*4.0+dQ1*dQ5*m6*t3*t5*t6*t8*t9*t11*t18*t32*4.0-dQ1*dQ4*m6*t2*t3*t4*t7*t8*t9*t26*t35*4.0-dQ1*dQ4*m6*t2*t4*t6*t7*t10*t11*t21*t33*4.0-dQ1*dQ5*m5*t2*t3*t5*t7*t8*t10*t25*t34*4.0-dQ1*dQ6*m6*t2*t3*t6*t7*t8*t11*t21*t34*4.0-dQ2*dQ5*m6*t2*t4*t5*t8*t9*t10*t18*t36*2.0-dQ2*dQ5*m6*t3*t4*t5*t7*t9*t10*t18*t36*2.0-dQ1*dQ4*m6*t3*t4*t6*t8*t10*t11*t21*t32*4.0-dQ1*dQ5*m6*t2*t5*t6*t7*t9*t11*t21*t33*4.0-dQ1*dQ6*m6*t2*t3*t6*t7*t8*t11*t21*t35*4.0-dQ3*dQ5*m6*t2*t4*t5*t8*t9*t10*t18*t36*2.0-dQ3*dQ5*m6*t3*t4*t5*t7*t9*t10*t18*t36*2.0;
et241 = dQ1*dQ5*m6*t2*t3*t5*t7*t8*t10*t26*t34*-4.0-dQ1*dQ5*m6*t3*t5*t6*t8*t9*t11*t21*t32*4.0-dQ2*dQ6*m6*t2*t4*t6*t8*t9*t11*t18*t35*2.0-dQ2*dQ6*m6*t3*t4*t6*t7*t9*t11*t18*t35*2.0-dQ3*dQ6*m6*t2*t4*t6*t8*t9*t11*t18*t35*2.0-dQ3*dQ6*m6*t3*t4*t6*t7*t9*t11*t18*t35*2.0+dQ1*dQ4*m6*t2*t5*t7*t9*t10*t18*t33*t36*4.0+dQ1*dQ4*m6*t3*t5*t8*t9*t10*t18*t32*t36*4.0-dQ1*dQ4*m6*t2*t5*t7*t9*t10*t21*t33*t36*4.0-dQ1*dQ4*m6*t3*t5*t8*t9*t10*t21*t32*t36*4.0+dQ1*dQ5*m6*t4*t6*t9*t10*t11*t18*t32*t33*4.0-dQ1*dQ5*m6*t4*t6*t9*t10*t11*t21*t32*t33*4.0-Lx2*Lxcm6*dQ1*dQ2*m6*t2*t3*t4*t5*t6*t7*4.0-Lx2*Lxcm6*dQ1*dQ3*m6*t2*t3*t4*t5*t6*t7*2.0;
et242 = Lx4*Lxcm4*dQ1*dQ4*m4*t2*t3*t4*t7*t8*t9*8.0+Lx4*Lxcm6*dQ2*dQ3*m6*t2*t3*t4*t5*t6*t9*4.0+Lx4*Lxcm5*dQ1*dQ2*m5*t2*t3*t4*t7*t8*t10*8.0+Lx3*Lxcm5*dQ1*dQ4*m5*t2*t3*t5*t7*t8*t9*4.0+Lx4*Lxcm5*dQ1*dQ3*m5*t2*t3*t4*t7*t8*t10*8.0+Lx3*Lxcm5*dQ1*dQ5*m5*t2*t3*t4*t7*t8*t10*4.0+Lx3*Lxcm6*dQ1*dQ2*m6*t2*t3*t6*t7*t8*t10*8.0+Lx3*Lxcm6*dQ1*dQ3*m6*t2*t3*t6*t7*t8*t10*8.0+Lx3*Lxcm6*dQ1*dQ4*m6*t2*t3*t4*t7*t8*t11*4.0+Lx2*Lxcm6*dQ1*dQ4*m6*t2*t5*t6*t7*t8*t9*2.0+Lx2*Lxcm6*dQ1*dQ5*m6*t2*t4*t6*t7*t8*t10*2.0+Lx3*Lxcm6*dQ1*dQ6*m6*t2*t3*t6*t7*t8*t9*4.0+Lx2*Lxcm6*dQ1*dQ6*m6*t2*t4*t5*t7*t8*t11*2.0-Lx4*Lxcm6*dQ2*dQ3*m6*t4*t5*t6*t7*t8*t9*4.0;
et243 = Lx4*Lxcm6*dQ2*dQ5*m6*t2*t4*t6*t8*t9*t10*-2.0-Lx4*Lxcm6*dQ2*dQ5*m6*t3*t4*t6*t7*t9*t10*2.0-Lx4*Lxcm6*dQ2*dQ6*m6*t2*t4*t5*t8*t9*t11*2.0-Lx4*Lxcm6*dQ2*dQ6*m6*t3*t4*t5*t7*t9*t11*2.0-Lx4*Lxcm6*dQ3*dQ5*m6*t2*t4*t6*t8*t9*t10*2.0-Lx4*Lxcm6*dQ3*dQ5*m6*t3*t4*t6*t7*t9*t10*2.0-Lx4*Lxcm6*dQ3*dQ6*m6*t2*t4*t5*t8*t9*t11*2.0-Lx4*Lxcm6*dQ3*dQ6*m6*t3*t4*t5*t7*t9*t11*2.0-Lx3*Lxcm6*dQ1*dQ2*m6*t2*t4*t5*t6*t7*t33*8.0-Lx3*Lxcm6*dQ1*dQ2*m6*t3*t4*t5*t6*t8*t32*8.0-Lx3*Lxcm6*dQ1*dQ3*m6*t2*t4*t5*t6*t7*t33*8.0-Lx3*Lxcm6*dQ1*dQ3*m6*t3*t4*t5*t6*t8*t32*8.0-Lx4*Lxcm6*dQ1*dQ5*m6*t2*t4*t5*t6*t7*t33*4.0-Lx4*Lxcm6*dQ1*dQ5*m6*t3*t4*t5*t6*t8*t32*4.0;
et244 = Lx4*Lxcm5*dQ1*dQ5*m5*t2*t3*t7*t8*t10*t34*4.0+Lx4*Lxcm6*dQ1*dQ2*m6*t2*t4*t7*t9*t11*t33*8.0+Lx4*Lxcm6*dQ1*dQ2*m6*t3*t4*t8*t9*t11*t32*8.0+Lx4*Lxcm6*dQ1*dQ3*m6*t2*t4*t7*t9*t11*t33*8.0+Lx4*Lxcm6*dQ1*dQ4*m6*t2*t3*t7*t8*t11*t34*8.0+Lx4*Lxcm6*dQ1*dQ3*m6*t3*t4*t8*t9*t11*t32*8.0+Lx4*Lxcm6*dQ1*dQ4*m6*t2*t6*t7*t9*t10*t33*4.0+Lx4*Lxcm6*dQ1*dQ4*m6*t3*t6*t8*t9*t10*t32*4.0+Lx4*Lxcm6*dQ1*dQ6*m6*t2*t4*t7*t10*t11*t33*4.0+Lx4*Lxcm6*dQ1*dQ6*m6*t3*t4*t8*t10*t11*t32*4.0-Lx4*Lxcm6*dQ1*dQ2*m6*t2*t5*t6*t7*t33*t34*8.0-Lx4*Lxcm6*dQ1*dQ2*m6*t3*t5*t6*t8*t32*t34*8.0-Lx4*Lxcm6*dQ1*dQ3*m6*t2*t5*t6*t7*t33*t34*8.0-Lx4*Lxcm6*dQ1*dQ3*m6*t3*t5*t6*t8*t32*t34*8.0;
et245 = Lx4*Lxcm6*dQ1*dQ4*m6*t4*t5*t6*t9*t32*t33*-8.0+Lx2*Lycm6*dQ1*dQ2*m6*t2*t3*t4*t5*t7*t11*4.0+Lx2*Lycm6*dQ1*dQ3*m6*t2*t3*t4*t5*t7*t11*2.0+Lx3*Lycm6*dQ1*dQ4*m6*t2*t3*t4*t6*t7*t8*4.0+Lx2*Lycm6*dQ1*dQ6*m6*t2*t4*t5*t6*t7*t8*2.0-Lx4*Lycm6*dQ2*dQ3*m6*t2*t3*t4*t5*t9*t11*4.0-Lx4*Lycm6*dQ2*dQ6*m6*t2*t4*t5*t6*t8*t9*2.0-Lx4*Lycm6*dQ2*dQ6*m6*t3*t4*t5*t6*t7*t9*2.0-Lx3*Lycm6*dQ1*dQ2*m6*t2*t3*t7*t8*t10*t11*8.0-Lx4*Lycm6*dQ3*dQ6*m6*t2*t4*t5*t6*t8*t9*2.0-Lx4*Lycm6*dQ3*dQ6*m6*t3*t4*t5*t6*t7*t9*2.0-Lx3*Lycm6*dQ1*dQ3*m6*t2*t3*t7*t8*t10*t11*8.0-Lx2*Lycm6*dQ1*dQ4*m6*t2*t5*t7*t8*t9*t11*2.0-Lx2*Lycm6*dQ1*dQ5*m6*t2*t4*t7*t8*t10*t11*2.0;
et246 = Lx3*Lycm6*dQ1*dQ6*m6*t2*t3*t7*t8*t9*t11*-4.0+Lx4*Lycm6*dQ2*dQ3*m6*t4*t5*t7*t8*t9*t11*4.0+Lx4*Lycm6*dQ2*dQ5*m6*t2*t4*t8*t9*t10*t11*2.0+Lx4*Lycm6*dQ2*dQ5*m6*t3*t4*t7*t9*t10*t11*2.0+Lx4*Lycm6*dQ3*dQ5*m6*t2*t4*t8*t9*t10*t11*2.0+Lx4*Lycm6*dQ3*dQ5*m6*t3*t4*t7*t9*t10*t11*2.0+Lx3*Lycm6*dQ1*dQ2*m6*t2*t4*t5*t7*t11*t33*8.0+Lx4*Lycm6*dQ1*dQ2*m6*t2*t4*t6*t7*t9*t33*8.0+Lx3*Lycm6*dQ1*dQ2*m6*t3*t4*t5*t8*t11*t32*8.0+Lx3*Lycm6*dQ1*dQ3*m6*t2*t4*t5*t7*t11*t33*8.0+Lx4*Lycm6*dQ1*dQ2*m6*t3*t4*t6*t8*t9*t32*8.0+Lx4*Lycm6*dQ1*dQ3*m6*t2*t4*t6*t7*t9*t33*8.0+Lx4*Lycm6*dQ1*dQ4*m6*t2*t3*t6*t7*t8*t34*8.0+Lx3*Lycm6*dQ1*dQ3*m6*t3*t4*t5*t8*t11*t32*8.0;
et247 = Lx4*Lycm6*dQ1*dQ3*m6*t3*t4*t6*t8*t9*t32*8.0+Lx4*Lycm6*dQ1*dQ5*m6*t2*t4*t5*t7*t11*t33*4.0+Lx4*Lycm6*dQ1*dQ5*m6*t3*t4*t5*t8*t11*t32*4.0+Lx4*Lycm6*dQ1*dQ6*m6*t2*t4*t6*t7*t10*t33*4.0+Lx4*Lycm6*dQ1*dQ6*m6*t3*t4*t6*t8*t10*t32*4.0-Lx4*Lycm6*dQ1*dQ4*m6*t2*t7*t9*t10*t11*t33*4.0-Lx4*Lycm6*dQ1*dQ4*m6*t3*t8*t9*t10*t11*t32*4.0+Lx4*Lycm6*dQ1*dQ2*m6*t2*t5*t7*t11*t33*t34*8.0+Lx4*Lycm6*dQ1*dQ2*m6*t3*t5*t8*t11*t32*t34*8.0+Lx4*Lycm6*dQ1*dQ3*m6*t2*t5*t7*t11*t33*t34*8.0+Lx4*Lycm6*dQ1*dQ3*m6*t3*t5*t8*t11*t32*t34*8.0+Lx4*Lycm6*dQ1*dQ4*m6*t4*t5*t9*t11*t32*t33*8.0-Lxcm5*Lycm5*dQ1*dQ2*m5*t2*t3*t7*t8*t9*t10*8.0-Lxcm5*Lycm5*dQ1*dQ3*m5*t2*t3*t7*t8*t9*t10*8.0;
et248 = Lxcm6*Lycm6*dQ2*dQ3*m6*t2*t3*t4*t6*t9*t11*-4.0+Lxcm6*Lycm6*dQ1*dQ2*m6*t2*t3*t7*t8*t9*t10*8.0+Lxcm6*Lycm6*dQ1*dQ3*m6*t2*t3*t7*t8*t9*t10*8.0-Lxcm6*Lycm6*dQ2*dQ6*m6*t2*t3*t4*t6*t10*t11*4.0-Lxcm6*Lycm6*dQ3*dQ6*m6*t2*t3*t4*t6*t10*t11*4.0+Lxcm6*Lycm6*dQ4*dQ5*m6*t2*t3*t5*t6*t10*t11*4.0-Lxcm6*Lycm6*dQ5*dQ6*m6*t2*t4*t5*t6*t8*t11*4.0-Lxcm6*Lycm6*dQ5*dQ6*m6*t3*t4*t5*t6*t7*t11*4.0+Lxcm6*Lycm6*dQ2*dQ3*m6*t4*t6*t7*t8*t9*t11*4.0+Lxcm6*Lycm6*dQ1*dQ6*m6*t2*t6*t7*t9*t10*t11*8.0+Lxcm6*Lycm6*dQ1*dQ6*m6*t3*t6*t8*t9*t10*t11*8.0+Lxcm6*Lycm6*dQ2*dQ6*m6*t4*t6*t7*t8*t10*t11*4.0+Lxcm6*Lycm6*dQ3*dQ6*m6*t4*t6*t7*t8*t10*t11*4.0-Lxcm6*Lycm6*dQ4*dQ5*m6*t5*t6*t7*t8*t10*t11*4.0;
et249 = Lxcm6*Lycm6*dQ4*dQ6*m6*t2*t6*t8*t9*t10*t11*-4.0-Lxcm6*Lycm6*dQ4*dQ6*m6*t3*t6*t7*t9*t10*t11*4.0+Lxcm5*Lycm5*dQ1*dQ2*m5*t2*t4*t5*t7*t9*t33*8.0+Lxcm5*Lycm5*dQ1*dQ2*m5*t3*t4*t5*t8*t9*t32*8.0+Lxcm5*Lycm5*dQ1*dQ3*m5*t2*t4*t5*t7*t9*t33*8.0+Lxcm5*Lycm5*dQ1*dQ4*m5*t2*t3*t5*t7*t8*t34*8.0+Lxcm5*Lycm5*dQ1*dQ3*m5*t3*t4*t5*t8*t9*t32*8.0-Lxcm6*Lycm6*dQ1*dQ2*m6*t2*t4*t5*t7*t9*t33*8.0-Lxcm6*Lycm6*dQ1*dQ2*m6*t3*t4*t5*t8*t9*t32*8.0-Lxcm6*Lycm6*dQ1*dQ3*m6*t2*t4*t5*t7*t9*t33*8.0-Lxcm6*Lycm6*dQ1*dQ4*m6*t2*t3*t5*t7*t8*t34*8.0-Lxcm6*Lycm6*dQ1*dQ3*m6*t3*t4*t5*t8*t9*t32*8.0-Lxcm6*Lycm6*dQ1*dQ2*m6*t2*t4*t5*t7*t9*t36*8.0;
et250 = Lxcm6*Lycm6*dQ1*dQ4*m6*t2*t3*t5*t7*t8*t36*-8.0-Lxcm6*Lycm6*dQ1*dQ3*m6*t2*t4*t5*t7*t9*t36*8.0-Lxcm6*Lycm6*dQ1*dQ2*m6*t3*t4*t5*t8*t9*t36*8.0-Lxcm6*Lycm6*dQ1*dQ6*m6*t2*t4*t5*t7*t10*t33*8.0-Lxcm6*Lycm6*dQ1*dQ3*m6*t3*t4*t5*t8*t9*t36*8.0-Lxcm6*Lycm6*dQ1*dQ5*m6*t2*t4*t6*t7*t11*t33*8.0-Lxcm6*Lycm6*dQ1*dQ6*m6*t3*t4*t5*t8*t10*t32*8.0-Lxcm6*Lycm6*dQ1*dQ5*m6*t3*t4*t6*t8*t11*t32*8.0-Lxcm6*Lycm6*dQ2*dQ4*m6*t2*t4*t5*t8*t9*t36*8.0-Lxcm6*Lycm6*dQ2*dQ4*m6*t3*t4*t5*t7*t9*t36*8.0-Lxcm6*Lycm6*dQ1*dQ2*m6*t4*t5*t6*t10*t11*t32*8.0-Lxcm6*Lycm6*dQ1*dQ5*m6*t2*t4*t6*t7*t11*t35*8.0-Lxcm6*Lycm6*dQ1*dQ6*m6*t2*t4*t5*t7*t10*t36*8.0;
et251 = Lxcm6*Lycm6*dQ3*dQ4*m6*t2*t4*t5*t8*t9*t36*-8.0-Lxcm6*Lycm6*dQ3*dQ4*m6*t3*t4*t5*t7*t9*t36*8.0-Lxcm6*Lycm6*dQ1*dQ2*m6*t4*t5*t6*t10*t11*t33*8.0-Lxcm6*Lycm6*dQ1*dQ3*m6*t4*t5*t6*t10*t11*t32*8.0-Lxcm6*Lycm6*dQ1*dQ3*m6*t4*t5*t6*t10*t11*t33*8.0-Lxcm6*Lycm6*dQ1*dQ5*m6*t3*t4*t6*t8*t11*t35*8.0-Lxcm6*Lycm6*dQ1*dQ6*m6*t3*t4*t5*t8*t10*t36*8.0-Lxcm6*Lycm6*dQ2*dQ5*m6*t2*t3*t6*t9*t11*t35*4.0-Lxcm6*Lycm6*dQ2*dQ6*m6*t2*t3*t5*t9*t10*t36*4.0-Lxcm6*Lycm6*dQ1*dQ6*m6*t4*t5*t6*t9*t11*t32*8.0-Lxcm6*Lycm6*dQ2*dQ6*m6*t2*t5*t6*t8*t11*t34*8.0-Lxcm6*Lycm6*dQ2*dQ6*m6*t3*t5*t6*t7*t11*t34*8.0-Lxcm6*Lycm6*dQ3*dQ5*m6*t2*t3*t6*t9*t11*t35*4.0;
et252 = Lxcm6*Lycm6*dQ3*dQ6*m6*t2*t3*t5*t9*t10*t36*-4.0-Lxcm6*Lycm6*dQ1*dQ6*m6*t4*t5*t6*t9*t11*t33*8.0-Lxcm6*Lycm6*dQ3*dQ6*m6*t2*t5*t6*t8*t11*t34*8.0-Lxcm6*Lycm6*dQ3*dQ6*m6*t3*t5*t6*t7*t11*t34*8.0+Lxcm6*Lycm6*dQ4*dQ5*m6*t2*t4*t6*t8*t11*t35*4.0+Lxcm6*Lycm6*dQ4*dQ5*m6*t3*t4*t6*t7*t11*t35*4.0+Lxcm6*Lycm6*dQ4*dQ6*m6*t2*t4*t5*t8*t10*t36*4.0+Lxcm6*Lycm6*dQ4*dQ6*m6*t3*t4*t5*t7*t10*t36*4.0+Lxcm6*Lycm6*dQ2*dQ5*m6*t6*t7*t8*t9*t11*t35*4.0+Lxcm6*Lycm6*dQ2*dQ6*m6*t5*t7*t8*t9*t10*t36*4.0+Lxcm6*Lycm6*dQ3*dQ5*m6*t6*t7*t8*t9*t11*t35*4.0+Lxcm6*Lycm6*dQ3*dQ6*m6*t5*t7*t8*t9*t10*t36*4.0+Lxcm6*Lycm6*dQ1*dQ2*m6*t2*t6*t7*t11*t33*t34*8.0-Lxcm6*Lycm6*dQ1*dQ6*m6*t2*t3*t7*t8*t34*t35*4.0;
et253 = Lxcm6*Lycm6*dQ1*dQ2*m6*t2*t6*t7*t11*t33*t35*8.0+Lxcm6*Lycm6*dQ1*dQ2*m6*t3*t6*t8*t11*t32*t34*8.0+Lxcm6*Lycm6*dQ1*dQ3*m6*t2*t6*t7*t11*t33*t34*8.0+Lxcm6*Lycm6*dQ1*dQ4*m6*t2*t4*t7*t10*t33*t36*8.0+Lxcm6*Lycm6*dQ1*dQ6*m6*t2*t3*t7*t8*t34*t36*8.0-Lxcm6*Lycm6*dQ1*dQ2*m6*t2*t6*t7*t11*t34*t35*4.0+Lxcm6*Lycm6*dQ1*dQ2*m6*t3*t6*t8*t11*t32*t35*8.0+Lxcm6*Lycm6*dQ1*dQ3*m6*t2*t6*t7*t11*t33*t35*8.0+Lxcm6*Lycm6*dQ1*dQ3*m6*t3*t6*t8*t11*t32*t34*8.0+Lxcm6*Lycm6*dQ1*dQ4*m6*t3*t4*t8*t10*t32*t36*8.0+Lxcm6*Lycm6*dQ1*dQ5*m6*t2*t5*t7*t9*t33*t36*8.0+Lxcm6*Lycm6*dQ1*dQ6*m6*t2*t3*t7*t8*t35*t36*8.0-Lxcm6*Lycm6*dQ1*dQ3*m6*t2*t6*t7*t11*t34*t35*4.0+Lxcm6*Lycm6*dQ1*dQ3*m6*t3*t6*t8*t11*t32*t35*8.0;
et254 = Lxcm6*Lycm6*dQ1*dQ5*m6*t3*t5*t8*t9*t32*t36*8.0-Lxcm6*Lycm6*dQ1*dQ2*m6*t3*t6*t8*t11*t34*t35*4.0+Lxcm6*Lycm6*dQ1*dQ4*m6*t4*t6*t9*t11*t32*t33*8.0-Lxcm6*Lycm6*dQ1*dQ3*m6*t3*t6*t8*t11*t34*t35*4.0-Lxcm6*Lycm6*dQ1*dQ4*m6*t4*t6*t9*t11*t32*t35*4.0-Lxcm6*Lycm6*dQ2*dQ4*m6*t2*t6*t8*t11*t34*t35*4.0-Lxcm6*Lycm6*dQ2*dQ4*m6*t3*t6*t7*t11*t34*t35*4.0-Lxcm6*Lycm6*dQ2*dQ6*m6*t2*t4*t8*t9*t35*t36*4.0-Lxcm6*Lycm6*dQ2*dQ6*m6*t3*t4*t7*t9*t35*t36*4.0-Lxcm6*Lycm6*dQ1*dQ4*m6*t4*t6*t9*t11*t33*t35*4.0+Lxcm6*Lycm6*dQ1*dQ5*m6*t5*t6*t10*t11*t32*t33*8.0-Lxcm6*Lycm6*dQ3*dQ4*m6*t2*t6*t8*t11*t34*t35*4.0-Lxcm6*Lycm6*dQ3*dQ4*m6*t3*t6*t7*t11*t34*t35*4.0-Lxcm6*Lycm6*dQ3*dQ6*m6*t2*t4*t8*t9*t35*t36*4.0;
et255 = Lxcm6*Lycm6*dQ3*dQ6*m6*t3*t4*t7*t9*t35*t36*-4.0-Lxcm6*Lycm6*dQ1*dQ5*m6*t5*t6*t10*t11*t32*t34*4.0-Lxcm6*Lycm6*dQ1*dQ5*m6*t5*t6*t10*t11*t33*t34*4.0+Lxcm6*Lycm6*dQ1*dQ5*m6*t4*t9*t10*t32*t33*t36*8.0-Lx4*Lz6*dQ1*dQ2*m6*t2*t3*t4*t5*t7*t8*8.0-Lx4*Lz6*dQ1*dQ3*m6*t2*t3*t4*t5*t7*t8*8.0-Lx3*Lz6*dQ1*dQ5*m6*t2*t3*t4*t5*t7*t8*4.0+Lx3*Lz6*dQ1*dQ4*m6*t2*t3*t7*t8*t9*t10*4.0-Lx4*Lz6*dQ1*dQ5*m6*t2*t3*t5*t7*t8*t34*4.0-Lx4*Lzcm5*dQ1*dQ2*m5*t2*t3*t4*t5*t7*t8*8.0-Lx4*Lzcm5*dQ1*dQ3*m5*t2*t3*t4*t5*t7*t8*8.0-Lx3*Lzcm5*dQ1*dQ5*m5*t2*t3*t4*t5*t7*t8*4.0-Lx4*Lzcm6*dQ1*dQ2*m6*t2*t3*t4*t5*t7*t8*8.0;
et256 = Lx4*Lzcm6*dQ1*dQ3*m6*t2*t3*t4*t5*t7*t8*-8.0-Lx3*Lzcm6*dQ1*dQ5*m6*t2*t3*t4*t5*t7*t8*4.0+Lxcm6*Lz6*dQ1*dQ2*m6*t2*t3*t4*t6*t7*t8*8.0+Lxcm6*Lz6*dQ1*dQ3*m6*t2*t3*t4*t6*t7*t8*8.0+Lx3*Lzcm5*dQ1*dQ4*m5*t2*t3*t7*t8*t9*t10*4.0+Lxcm6*Lz6*dQ1*dQ5*m6*t2*t4*t5*t6*t7*t10*8.0+Lx3*Lzcm6*dQ1*dQ4*m6*t2*t3*t7*t8*t9*t10*4.0+Lxcm6*Lz6*dQ1*dQ5*m6*t3*t4*t5*t6*t8*t10*8.0+Lxcm6*Lz6*dQ2*dQ5*m6*t2*t3*t5*t6*t9*t10*4.0+Lxcm6*Lz6*dQ3*dQ5*m6*t2*t3*t5*t6*t9*t10*4.0-Lxcm6*Lz6*dQ4*dQ5*m6*t2*t4*t5*t6*t8*t10*4.0-Lxcm6*Lz6*dQ4*dQ5*m6*t3*t4*t5*t6*t7*t10*4.0-Lxcm6*Lz6*dQ1*dQ2*m6*t2*t4*t7*t9*t10*t11*4.0-Lxcm6*Lz6*dQ1*dQ4*m6*t2*t3*t7*t8*t10*t11*4.0;
et257 = Lxcm6*Lz6*dQ1*dQ3*m6*t2*t4*t7*t9*t10*t11*-4.0-Lxcm6*Lz6*dQ1*dQ2*m6*t3*t4*t8*t9*t10*t11*4.0-Lxcm6*Lz6*dQ1*dQ3*m6*t3*t4*t8*t9*t10*t11*4.0-Lxcm6*Lz6*dQ2*dQ4*m6*t2*t4*t8*t9*t10*t11*4.0-Lxcm6*Lz6*dQ2*dQ4*m6*t3*t4*t7*t9*t10*t11*4.0-Lxcm6*Lz6*dQ3*dQ4*m6*t2*t4*t8*t9*t10*t11*4.0-Lxcm6*Lz6*dQ3*dQ4*m6*t3*t4*t7*t9*t10*t11*4.0-Lxcm6*Lz6*dQ2*dQ5*m6*t5*t6*t7*t8*t9*t10*4.0-Lxcm6*Lz6*dQ3*dQ5*m6*t5*t6*t7*t8*t9*t10*4.0-Lx4*Lzcm5*dQ1*dQ5*m5*t2*t3*t5*t7*t8*t34*4.0-Lx4*Lzcm6*dQ1*dQ5*m6*t2*t3*t5*t7*t8*t34*4.0-Lxcm6*Lz6*dQ1*dQ2*m6*t2*t5*t6*t7*t10*t33*8.0+Lxcm6*Lz6*dQ1*dQ5*m6*t2*t3*t6*t7*t8*t34*4.0+Lxcm6*Lz6*dQ1*dQ2*m6*t2*t5*t6*t7*t10*t34*4.0;
et258 = Lxcm6*Lz6*dQ1*dQ2*m6*t3*t5*t6*t8*t10*t32*-8.0-Lxcm6*Lz6*dQ1*dQ3*m6*t2*t5*t6*t7*t10*t33*8.0-Lxcm6*Lz6*dQ1*dQ4*m6*t2*t4*t5*t7*t11*t33*4.0-Lxcm6*Lz6*dQ1*dQ5*m6*t2*t3*t6*t7*t8*t35*8.0+Lxcm6*Lz6*dQ1*dQ3*m6*t2*t5*t6*t7*t10*t34*4.0-Lxcm6*Lz6*dQ1*dQ3*m6*t3*t5*t6*t8*t10*t32*8.0-Lxcm6*Lz6*dQ1*dQ4*m6*t3*t4*t5*t8*t11*t32*4.0+Lxcm6*Lz6*dQ1*dQ2*m6*t3*t5*t6*t8*t10*t34*4.0-Lxcm6*Lz6*dQ1*dQ6*m6*t2*t5*t6*t7*t9*t33*4.0+Lxcm6*Lz6*dQ1*dQ3*m6*t3*t5*t6*t8*t10*t34*4.0-Lxcm6*Lz6*dQ1*dQ6*m6*t3*t5*t6*t8*t9*t32*4.0+Lxcm6*Lz6*dQ1*dQ4*m6*t4*t5*t6*t9*t10*t32*4.0+Lxcm6*Lz6*dQ2*dQ4*m6*t2*t5*t6*t8*t10*t34*4.0+Lxcm6*Lz6*dQ2*dQ4*m6*t3*t5*t6*t7*t10*t34*4.0;
et259 = Lxcm6*Lz6*dQ1*dQ4*m6*t4*t5*t6*t9*t10*t33*4.0+Lxcm6*Lz6*dQ3*dQ4*m6*t2*t5*t6*t8*t10*t34*4.0+Lxcm6*Lz6*dQ3*dQ4*m6*t3*t5*t6*t7*t10*t34*4.0+Lxcm6*Lz6*dQ1*dQ5*m6*t2*t7*t9*t10*t11*t33*4.0+Lxcm6*Lz6*dQ1*dQ5*m6*t3*t8*t9*t10*t11*t32*4.0-Lxcm6*Lz6*dQ1*dQ4*m6*t2*t6*t7*t9*t33*t35*8.0-Lxcm6*Lz6*dQ1*dQ4*m6*t3*t6*t8*t9*t32*t35*8.0-Lxcm6*Lz6*dQ1*dQ6*m6*t2*t4*t7*t11*t33*t35*8.0-Lxcm6*Lz6*dQ1*dQ5*m6*t4*t5*t9*t11*t32*t33*4.0-Lxcm6*Lz6*dQ1*dQ6*m6*t3*t4*t8*t11*t32*t35*8.0-Lxcm6*Lz6*dQ1*dQ6*m6*t4*t6*t9*t10*t32*t33*4.0-Lxcm6*Lz6*dQ1*dQ6*m6*t5*t10*t11*t32*t33*t34*4.0+Lxcm6*Lzcm6*dQ1*dQ2*m6*t2*t3*t4*t6*t7*t8*8.0+Lxcm6*Lzcm6*dQ1*dQ3*m6*t2*t3*t4*t6*t7*t8*8.0;
et260 = Lxcm5*Lzcm5*dQ2*dQ3*m5*t2*t3*t4*t5*t9*t10*4.0+Lxcm6*Lzcm6*dQ1*dQ5*m6*t2*t4*t5*t6*t7*t10*8.0+Lxcm6*Lzcm6*dQ1*dQ5*m6*t3*t4*t5*t6*t8*t10*8.0+Lxcm6*Lzcm6*dQ2*dQ5*m6*t2*t3*t5*t6*t9*t10*4.0+Lxcm6*Lzcm6*dQ3*dQ5*m6*t2*t3*t5*t6*t9*t10*4.0-Lxcm6*Lzcm6*dQ4*dQ5*m6*t2*t4*t5*t6*t8*t10*4.0-Lxcm6*Lzcm6*dQ4*dQ5*m6*t3*t4*t5*t6*t7*t10*4.0-Lxcm5*Lzcm5*dQ2*dQ3*m5*t4*t5*t7*t8*t9*t10*4.0-Lxcm6*Lzcm6*dQ1*dQ2*m6*t2*t4*t7*t9*t10*t11*4.0-Lxcm6*Lzcm6*dQ1*dQ4*m6*t2*t3*t7*t8*t10*t11*4.0-Lxcm6*Lzcm6*dQ1*dQ3*m6*t2*t4*t7*t9*t10*t11*4.0-Lxcm6*Lzcm6*dQ1*dQ2*m6*t3*t4*t8*t9*t10*t11*4.0-Lxcm6*Lzcm6*dQ1*dQ3*m6*t3*t4*t8*t9*t10*t11*4.0-Lxcm6*Lzcm6*dQ2*dQ4*m6*t2*t4*t8*t9*t10*t11*4.0;
et261 = Lxcm6*Lzcm6*dQ2*dQ4*m6*t3*t4*t7*t9*t10*t11*-4.0-Lxcm6*Lzcm6*dQ3*dQ4*m6*t2*t4*t8*t9*t10*t11*4.0-Lxcm6*Lzcm6*dQ3*dQ4*m6*t3*t4*t7*t9*t10*t11*4.0-Lxcm6*Lzcm6*dQ2*dQ5*m6*t5*t6*t7*t8*t9*t10*4.0-Lxcm6*Lzcm6*dQ3*dQ5*m6*t5*t6*t7*t8*t9*t10*4.0-Lxcm5*Lzcm5*dQ1*dQ2*m5*t2*t3*t4*t7*t8*t35*1.6e+1-Lxcm5*Lzcm5*dQ1*dQ3*m5*t2*t3*t4*t7*t8*t35*1.6e+1-Lxcm5*Lzcm5*dQ1*dQ5*m5*t2*t4*t5*t7*t10*t33*1.6e+1-Lxcm5*Lzcm5*dQ1*dQ5*m5*t3*t4*t5*t8*t10*t32*1.6e+1-Lxcm6*Lzcm6*dQ1*dQ2*m6*t2*t5*t6*t7*t10*t33*8.0+Lxcm6*Lzcm6*dQ1*dQ5*m6*t2*t3*t6*t7*t8*t34*4.0+Lxcm6*Lzcm6*dQ1*dQ2*m6*t2*t5*t6*t7*t10*t34*4.0-Lxcm6*Lzcm6*dQ1*dQ2*m6*t3*t5*t6*t8*t10*t32*8.0;
et262 = Lxcm6*Lzcm6*dQ1*dQ3*m6*t2*t5*t6*t7*t10*t33*-8.0-Lxcm6*Lzcm6*dQ1*dQ4*m6*t2*t4*t5*t7*t11*t33*4.0-Lxcm6*Lzcm6*dQ1*dQ5*m6*t2*t3*t6*t7*t8*t35*8.0+Lxcm6*Lzcm6*dQ1*dQ3*m6*t2*t5*t6*t7*t10*t34*4.0-Lxcm6*Lzcm6*dQ1*dQ3*m6*t3*t5*t6*t8*t10*t32*8.0-Lxcm6*Lzcm6*dQ1*dQ4*m6*t3*t4*t5*t8*t11*t32*4.0+Lxcm6*Lzcm6*dQ1*dQ2*m6*t3*t5*t6*t8*t10*t34*4.0-Lxcm6*Lzcm6*dQ1*dQ6*m6*t2*t5*t6*t7*t9*t33*4.0+Lxcm6*Lzcm6*dQ1*dQ3*m6*t3*t5*t6*t8*t10*t34*4.0-Lxcm6*Lzcm6*dQ1*dQ6*m6*t3*t5*t6*t8*t9*t32*4.0+Lxcm6*Lzcm6*dQ1*dQ4*m6*t4*t5*t6*t9*t10*t32*4.0+Lxcm6*Lzcm6*dQ2*dQ4*m6*t2*t5*t6*t8*t10*t34*4.0+Lxcm6*Lzcm6*dQ2*dQ4*m6*t3*t5*t6*t7*t10*t34*4.0+Lxcm6*Lzcm6*dQ1*dQ4*m6*t4*t5*t6*t9*t10*t33*4.0;
et263 = Lxcm6*Lzcm6*dQ3*dQ4*m6*t2*t5*t6*t8*t10*t34*4.0+Lxcm6*Lzcm6*dQ3*dQ4*m6*t3*t5*t6*t7*t10*t34*4.0+Lxcm6*Lzcm6*dQ1*dQ5*m6*t2*t7*t9*t10*t11*t33*4.0+Lxcm6*Lzcm6*dQ1*dQ5*m6*t3*t8*t9*t10*t11*t32*4.0-Lxcm5*Lzcm5*dQ1*dQ2*m5*t2*t5*t7*t10*t33*t34*8.0-Lxcm5*Lzcm5*dQ1*dQ2*m5*t3*t5*t8*t10*t32*t34*8.0-Lxcm5*Lzcm5*dQ1*dQ3*m5*t2*t5*t7*t10*t33*t34*8.0-Lxcm5*Lzcm5*dQ1*dQ5*m5*t2*t3*t7*t8*t34*t35*8.0-Lxcm5*Lzcm5*dQ1*dQ3*m5*t3*t5*t8*t10*t32*t34*8.0-Lxcm5*Lzcm5*dQ1*dQ4*m5*t4*t5*t9*t10*t32*t33*8.0-Lxcm6*Lzcm6*dQ1*dQ4*m6*t2*t6*t7*t9*t33*t35*8.0-Lxcm6*Lzcm6*dQ1*dQ4*m6*t3*t6*t8*t9*t32*t35*8.0-Lxcm6*Lzcm6*dQ1*dQ6*m6*t2*t4*t7*t11*t33*t35*8.0;
et264 = Lxcm6*Lzcm6*dQ1*dQ5*m6*t4*t5*t9*t11*t32*t33*-4.0-Lxcm6*Lzcm6*dQ1*dQ6*m6*t3*t4*t8*t11*t32*t35*8.0-Lxcm6*Lzcm6*dQ1*dQ6*m6*t4*t6*t9*t10*t32*t33*4.0-Lxcm6*Lzcm6*dQ1*dQ6*m6*t5*t10*t11*t32*t33*t34*4.0-Lycm6*Lz6*dQ1*dQ2*m6*t2*t3*t4*t7*t8*t11*8.0-Lycm6*Lz6*dQ1*dQ3*m6*t2*t3*t4*t7*t8*t11*8.0-Lycm6*Lz6*dQ1*dQ2*m6*t2*t4*t6*t7*t9*t10*4.0-Lycm6*Lz6*dQ1*dQ4*m6*t2*t3*t6*t7*t8*t10*4.0-Lycm6*Lz6*dQ1*dQ3*m6*t2*t4*t6*t7*t9*t10*4.0-Lycm6*Lz6*dQ1*dQ2*m6*t3*t4*t6*t8*t9*t10*4.0-Lycm6*Lz6*dQ1*dQ3*m6*t3*t4*t6*t8*t9*t10*4.0-Lycm6*Lz6*dQ1*dQ5*m6*t2*t4*t5*t7*t10*t11*8.0-Lycm6*Lz6*dQ2*dQ4*m6*t2*t4*t6*t8*t9*t10*4.0-Lycm6*Lz6*dQ2*dQ4*m6*t3*t4*t6*t7*t9*t10*4.0;
et265 = Lycm6*Lz6*dQ3*dQ4*m6*t2*t4*t6*t8*t9*t10*-4.0-Lycm6*Lz6*dQ3*dQ4*m6*t3*t4*t6*t7*t9*t10*4.0-Lycm6*Lz6*dQ1*dQ5*m6*t3*t4*t5*t8*t10*t11*8.0-Lycm6*Lz6*dQ2*dQ5*m6*t2*t3*t5*t9*t10*t11*4.0-Lycm6*Lz6*dQ3*dQ5*m6*t2*t3*t5*t9*t10*t11*4.0+Lycm6*Lz6*dQ4*dQ5*m6*t2*t4*t5*t8*t10*t11*4.0+Lycm6*Lz6*dQ4*dQ5*m6*t3*t4*t5*t7*t10*t11*4.0+Lycm6*Lz6*dQ2*dQ5*m6*t5*t7*t8*t9*t10*t11*4.0+Lycm6*Lz6*dQ3*dQ5*m6*t5*t7*t8*t9*t10*t11*4.0-Lycm6*Lz6*dQ1*dQ4*m6*t2*t4*t5*t6*t7*t33*4.0-Lycm6*Lz6*dQ1*dQ4*m6*t3*t4*t5*t6*t8*t32*4.0+Lycm6*Lz6*dQ1*dQ2*m6*t2*t5*t7*t10*t11*t33*8.0-Lycm6*Lz6*dQ1*dQ5*m6*t2*t3*t7*t8*t11*t34*4.0-Lycm6*Lz6*dQ1*dQ2*m6*t2*t5*t7*t10*t11*t34*4.0;
et266 = Lycm6*Lz6*dQ1*dQ2*m6*t3*t5*t8*t10*t11*t32*8.0+Lycm6*Lz6*dQ1*dQ3*m6*t2*t5*t7*t10*t11*t33*8.0+Lycm6*Lz6*dQ1*dQ5*m6*t2*t3*t7*t8*t11*t35*8.0-Lycm6*Lz6*dQ1*dQ3*m6*t2*t5*t7*t10*t11*t34*4.0+Lycm6*Lz6*dQ1*dQ3*m6*t3*t5*t8*t10*t11*t32*8.0+Lycm6*Lz6*dQ1*dQ5*m6*t2*t6*t7*t9*t10*t33*4.0-Lycm6*Lz6*dQ1*dQ2*m6*t3*t5*t8*t10*t11*t34*4.0+Lycm6*Lz6*dQ1*dQ5*m6*t3*t6*t8*t9*t10*t32*4.0+Lycm6*Lz6*dQ1*dQ6*m6*t2*t5*t7*t9*t11*t33*4.0-Lycm6*Lz6*dQ1*dQ3*m6*t3*t5*t8*t10*t11*t34*4.0+Lycm6*Lz6*dQ1*dQ6*m6*t3*t5*t8*t9*t11*t32*4.0-Lycm6*Lz6*dQ1*dQ4*m6*t4*t5*t9*t10*t11*t32*4.0-Lycm6*Lz6*dQ2*dQ4*m6*t2*t5*t8*t10*t11*t34*4.0-Lycm6*Lz6*dQ2*dQ4*m6*t3*t5*t7*t10*t11*t34*4.0;
et267 = Lycm6*Lz6*dQ2*dQ5*m6*t2*t4*t8*t9*t11*t35*-4.0-Lycm6*Lz6*dQ2*dQ5*m6*t3*t4*t7*t9*t11*t35*4.0-Lycm6*Lz6*dQ1*dQ4*m6*t4*t5*t9*t10*t11*t33*4.0-Lycm6*Lz6*dQ3*dQ4*m6*t2*t5*t8*t10*t11*t34*4.0-Lycm6*Lz6*dQ3*dQ4*m6*t3*t5*t7*t10*t11*t34*4.0-Lycm6*Lz6*dQ3*dQ5*m6*t2*t4*t8*t9*t11*t35*4.0-Lycm6*Lz6*dQ3*dQ5*m6*t3*t4*t7*t9*t11*t35*4.0-Lycm6*Lz6*dQ1*dQ6*m6*t2*t4*t6*t7*t33*t35*8.0-Lycm6*Lz6*dQ1*dQ5*m6*t4*t5*t6*t9*t32*t33*4.0-Lycm6*Lz6*dQ1*dQ6*m6*t3*t4*t6*t8*t32*t35*8.0+Lycm6*Lz6*dQ1*dQ4*m6*t2*t7*t9*t11*t33*t35*8.0+Lycm6*Lz6*dQ1*dQ4*m6*t3*t8*t9*t11*t32*t35*8.0+Lycm6*Lz6*dQ1*dQ6*m6*t4*t9*t10*t11*t32*t33*4.0-Lycm6*Lz6*dQ1*dQ6*m6*t5*t6*t10*t32*t33*t34*4.0;
et268 = Lycm5*Lzcm5*dQ1*dQ2*m5*t2*t3*t5*t7*t8*t9*8.0+Lycm5*Lzcm5*dQ1*dQ3*m5*t2*t3*t5*t7*t8*t9*8.0-Lycm6*Lzcm6*dQ1*dQ2*m6*t2*t3*t4*t7*t8*t11*8.0-Lycm6*Lzcm6*dQ1*dQ3*m6*t2*t3*t4*t7*t8*t11*8.0-Lycm6*Lzcm6*dQ1*dQ2*m6*t2*t4*t6*t7*t9*t10*4.0-Lycm6*Lzcm6*dQ1*dQ4*m6*t2*t3*t6*t7*t8*t10*4.0-Lycm6*Lzcm6*dQ1*dQ3*m6*t2*t4*t6*t7*t9*t10*4.0-Lycm6*Lzcm6*dQ1*dQ2*m6*t3*t4*t6*t8*t9*t10*4.0-Lycm6*Lzcm6*dQ1*dQ3*m6*t3*t4*t6*t8*t9*t10*4.0-Lycm6*Lzcm6*dQ1*dQ5*m6*t2*t4*t5*t7*t10*t11*8.0-Lycm6*Lzcm6*dQ2*dQ4*m6*t2*t4*t6*t8*t9*t10*4.0-Lycm6*Lzcm6*dQ2*dQ4*m6*t3*t4*t6*t7*t9*t10*4.0-Lycm6*Lzcm6*dQ3*dQ4*m6*t2*t4*t6*t8*t9*t10*4.0-Lycm6*Lzcm6*dQ3*dQ4*m6*t3*t4*t6*t7*t9*t10*4.0;
et269 = Lycm6*Lzcm6*dQ1*dQ5*m6*t3*t4*t5*t8*t10*t11*-8.0-Lycm6*Lzcm6*dQ2*dQ5*m6*t2*t3*t5*t9*t10*t11*4.0-Lycm6*Lzcm6*dQ3*dQ5*m6*t2*t3*t5*t9*t10*t11*4.0+Lycm6*Lzcm6*dQ4*dQ5*m6*t2*t4*t5*t8*t10*t11*4.0+Lycm6*Lzcm6*dQ4*dQ5*m6*t3*t4*t5*t7*t10*t11*4.0+Lycm6*Lzcm6*dQ2*dQ5*m6*t5*t7*t8*t9*t10*t11*4.0+Lycm6*Lzcm6*dQ3*dQ5*m6*t5*t7*t8*t9*t10*t11*4.0-Lycm6*Lzcm6*dQ1*dQ4*m6*t2*t4*t5*t6*t7*t33*4.0-Lycm6*Lzcm6*dQ1*dQ4*m6*t3*t4*t5*t6*t8*t32*4.0+Lycm5*Lzcm5*dQ1*dQ2*m5*t2*t4*t7*t9*t10*t33*8.0+Lycm5*Lzcm5*dQ1*dQ2*m5*t3*t4*t8*t9*t10*t32*8.0+Lycm5*Lzcm5*dQ1*dQ3*m5*t2*t4*t7*t9*t10*t33*8.0+Lycm5*Lzcm5*dQ1*dQ4*m5*t2*t3*t7*t8*t10*t34*8.0+Lycm5*Lzcm5*dQ1*dQ3*m5*t3*t4*t8*t9*t10*t32*8.0;
et270 = Lycm6*Lzcm6*dQ1*dQ2*m6*t2*t5*t7*t10*t11*t33*8.0-Lycm6*Lzcm6*dQ1*dQ5*m6*t2*t3*t7*t8*t11*t34*4.0-Lycm6*Lzcm6*dQ1*dQ2*m6*t2*t5*t7*t10*t11*t34*4.0+Lycm6*Lzcm6*dQ1*dQ2*m6*t3*t5*t8*t10*t11*t32*8.0+Lycm6*Lzcm6*dQ1*dQ3*m6*t2*t5*t7*t10*t11*t33*8.0+Lycm6*Lzcm6*dQ1*dQ5*m6*t2*t3*t7*t8*t11*t35*8.0-Lycm6*Lzcm6*dQ1*dQ3*m6*t2*t5*t7*t10*t11*t34*4.0+Lycm6*Lzcm6*dQ1*dQ3*m6*t3*t5*t8*t10*t11*t32*8.0+Lycm6*Lzcm6*dQ1*dQ5*m6*t2*t6*t7*t9*t10*t33*4.0-Lycm6*Lzcm6*dQ1*dQ2*m6*t3*t5*t8*t10*t11*t34*4.0+Lycm6*Lzcm6*dQ1*dQ5*m6*t3*t6*t8*t9*t10*t32*4.0+Lycm6*Lzcm6*dQ1*dQ6*m6*t2*t5*t7*t9*t11*t33*4.0-Lycm6*Lzcm6*dQ1*dQ3*m6*t3*t5*t8*t10*t11*t34*4.0+Lycm6*Lzcm6*dQ1*dQ6*m6*t3*t5*t8*t9*t11*t32*4.0;
et271 = Lycm6*Lzcm6*dQ1*dQ4*m6*t4*t5*t9*t10*t11*t32*-4.0-Lycm6*Lzcm6*dQ2*dQ4*m6*t2*t5*t8*t10*t11*t34*4.0-Lycm6*Lzcm6*dQ2*dQ4*m6*t3*t5*t7*t10*t11*t34*4.0-Lycm6*Lzcm6*dQ2*dQ5*m6*t2*t4*t8*t9*t11*t35*4.0-Lycm6*Lzcm6*dQ2*dQ5*m6*t3*t4*t7*t9*t11*t35*4.0-Lycm6*Lzcm6*dQ1*dQ4*m6*t4*t5*t9*t10*t11*t33*4.0-Lycm6*Lzcm6*dQ3*dQ4*m6*t2*t5*t8*t10*t11*t34*4.0-Lycm6*Lzcm6*dQ3*dQ4*m6*t3*t5*t7*t10*t11*t34*4.0-Lycm6*Lzcm6*dQ3*dQ5*m6*t2*t4*t8*t9*t11*t35*4.0-Lycm6*Lzcm6*dQ3*dQ5*m6*t3*t4*t7*t9*t11*t35*4.0-Lycm6*Lzcm6*dQ1*dQ6*m6*t2*t4*t6*t7*t33*t35*8.0-Lycm6*Lzcm6*dQ1*dQ5*m6*t4*t5*t6*t9*t32*t33*4.0-Lycm6*Lzcm6*dQ1*dQ6*m6*t3*t4*t6*t8*t32*t35*8.0+Lycm6*Lzcm6*dQ1*dQ4*m6*t2*t7*t9*t11*t33*t35*8.0;
et272 = Lycm6*Lzcm6*dQ1*dQ4*m6*t3*t8*t9*t11*t32*t35*8.0+Lycm6*Lzcm6*dQ1*dQ6*m6*t4*t9*t10*t11*t32*t33*4.0-Lycm6*Lzcm6*dQ1*dQ6*m6*t5*t6*t10*t32*t33*t34*4.0+Lz6*Lzcm6*dQ1*dQ4*m6*t2*t3*t4*t7*t8*t9*8.0-Lz6*Lzcm6*dQ1*dQ5*m6*t2*t3*t5*t7*t8*t10*8.0+Lz6*Lzcm6*dQ2*dQ5*m6*t2*t4*t5*t8*t9*t10*4.0+Lz6*Lzcm6*dQ2*dQ5*m6*t3*t4*t5*t7*t9*t10*4.0+Lz6*Lzcm6*dQ3*dQ5*m6*t2*t4*t5*t8*t9*t10*4.0+Lz6*Lzcm6*dQ3*dQ5*m6*t3*t4*t5*t7*t9*t10*4.0-Lz6*Lzcm6*dQ1*dQ4*m6*t2*t5*t7*t9*t10*t33*8.0-Lz6*Lzcm6*dQ1*dQ4*m6*t3*t5*t8*t9*t10*t32*8.0+Lx4*Lxcm5*dQ1*dQ4*m5*t2*t3*t4*t5*t7*t8*t9*8.0+Lx4*Lxcm6*dQ1*dQ2*m6*t2*t3*t4*t6*t7*t8*t10*8.0+Lx3*Lxcm6*dQ1*dQ4*m6*t2*t3*t5*t6*t7*t8*t9*4.0;
et273 = Lx4*Lxcm6*dQ1*dQ3*m6*t2*t3*t4*t6*t7*t8*t10*8.0+Lx3*Lxcm6*dQ1*dQ5*m6*t2*t3*t4*t6*t7*t8*t10*4.0+Lx3*Lxcm6*dQ1*dQ6*m6*t2*t3*t4*t5*t7*t8*t11*4.0+Lx4*Lxcm6*dQ1*dQ6*m6*t2*t3*t4*t6*t7*t8*t9*4.0+Lx4*Lxcm6*dQ1*dQ5*m6*t2*t3*t6*t7*t8*t10*t34*4.0+Lx4*Lxcm6*dQ1*dQ6*m6*t2*t3*t5*t7*t8*t11*t34*4.0+Lx3*Lycm6*dQ1*dQ6*m6*t2*t3*t4*t5*t6*t7*t8*4.0-Lx4*Lycm6*dQ1*dQ2*m6*t2*t3*t4*t7*t8*t10*t11*8.0-Lx3*Lycm6*dQ1*dQ4*m6*t2*t3*t5*t7*t8*t9*t11*4.0-Lx4*Lycm6*dQ1*dQ3*m6*t2*t3*t4*t7*t8*t10*t11*8.0-Lx3*Lycm6*dQ1*dQ5*m6*t2*t3*t4*t7*t8*t10*t11*4.0-Lx4*Lycm6*dQ1*dQ6*m6*t2*t3*t4*t7*t8*t9*t11*4.0+Lx4*Lycm6*dQ1*dQ6*m6*t2*t3*t5*t6*t7*t8*t34*4.0;
et274 = Lx4*Lycm6*dQ1*dQ5*m6*t2*t3*t7*t8*t10*t11*t34*-4.0-Lxcm5*Lycm5*dQ1*dQ5*m5*t2*t3*t4*t7*t8*t9*t10*4.0+Lxcm6*Lycm6*dQ1*dQ5*m6*t2*t3*t4*t7*t8*t9*t10*4.0+Lxcm6*Lycm6*dQ1*dQ4*m6*t2*t5*t6*t7*t9*t10*t11*4.0+Lxcm6*Lycm6*dQ2*dQ3*m6*t2*t5*t6*t8*t9*t10*t11*4.0+Lxcm6*Lycm6*dQ2*dQ3*m6*t3*t5*t6*t7*t9*t10*t11*4.0+Lxcm6*Lycm6*dQ1*dQ4*m6*t3*t5*t6*t8*t9*t10*t11*4.0-Lxcm6*Lycm6*dQ2*dQ3*m6*t2*t3*t4*t6*t9*t11*t35*4.0-Lxcm6*Lycm6*dQ1*dQ2*m6*t2*t3*t7*t8*t9*t10*t36*1.6e+1-Lxcm6*Lycm6*dQ1*dQ3*m6*t2*t3*t7*t8*t9*t10*t36*1.6e+1-Lxcm6*Lycm6*dQ1*dQ6*m6*t2*t6*t7*t9*t10*t11*t33*1.6e+1+Lxcm6*Lycm6*dQ2*dQ3*m6*t4*t6*t7*t8*t9*t11*t35*4.0-Lxcm6*Lycm6*dQ1*dQ6*m6*t3*t6*t8*t9*t10*t11*t32*1.6e+1;
et275 = Lxcm6*Lycm6*dQ1*dQ2*m6*t2*t4*t5*t7*t9*t33*t36*1.6e+1+Lxcm6*Lycm6*dQ1*dQ2*m6*t3*t4*t5*t8*t9*t32*t36*1.6e+1+Lxcm6*Lycm6*dQ1*dQ3*m6*t2*t4*t5*t7*t9*t33*t36*1.6e+1+Lxcm6*Lycm6*dQ1*dQ4*m6*t2*t3*t5*t7*t8*t34*t36*1.6e+1+Lxcm6*Lycm6*dQ1*dQ3*m6*t3*t4*t5*t8*t9*t32*t36*1.6e+1+Lxcm6*Lycm6*dQ1*dQ2*m6*t4*t5*t6*t10*t11*t32*t33*1.6e+1+Lxcm6*Lycm6*dQ1*dQ5*m6*t2*t4*t6*t7*t11*t33*t35*1.6e+1+Lxcm6*Lycm6*dQ1*dQ6*m6*t2*t4*t5*t7*t10*t33*t36*1.6e+1+Lxcm6*Lycm6*dQ1*dQ3*m6*t4*t5*t6*t10*t11*t32*t33*1.6e+1+Lxcm6*Lycm6*dQ1*dQ5*m6*t3*t4*t6*t8*t11*t32*t35*1.6e+1+Lxcm6*Lycm6*dQ1*dQ6*m6*t3*t4*t5*t8*t10*t32*t36*1.6e+1+Lxcm6*Lycm6*dQ1*dQ6*m6*t4*t5*t6*t9*t11*t32*t33*1.6e+1+Lxcm6*Lycm6*dQ1*dQ2*m6*t2*t6*t7*t11*t33*t34*t35*8.0;
et276 = Lxcm6*Lycm6*dQ1*dQ2*m6*t3*t6*t8*t11*t32*t34*t35*8.0+Lxcm6*Lycm6*dQ1*dQ3*m6*t2*t6*t7*t11*t33*t34*t35*8.0+Lxcm6*Lycm6*dQ1*dQ6*m6*t2*t3*t7*t8*t34*t35*t36*8.0+Lxcm6*Lycm6*dQ1*dQ3*m6*t3*t6*t8*t11*t32*t34*t35*8.0+Lxcm6*Lycm6*dQ1*dQ4*m6*t4*t6*t9*t11*t32*t33*t35*8.0+Lxcm6*Lycm6*dQ1*dQ5*m6*t5*t6*t10*t11*t32*t33*t34*8.0+Lx4*Lz6*dQ1*dQ4*m6*t2*t3*t4*t7*t8*t9*t10*8.0+Lx4*Lzcm5*dQ1*dQ4*m5*t2*t3*t4*t7*t8*t9*t10*8.0+Lxcm6*Lz6*dQ2*dQ3*m6*t2*t3*t4*t5*t6*t9*t10*4.0+Lx4*Lzcm6*dQ1*dQ4*m6*t2*t3*t4*t7*t8*t9*t10*8.0+Lxcm6*Lz6*dQ1*dQ2*m6*t2*t3*t5*t7*t8*t9*t11*8.0+Lxcm6*Lz6*dQ1*dQ3*m6*t2*t3*t5*t7*t8*t9*t11*8.0+Lxcm6*Lz6*dQ1*dQ6*m6*t2*t3*t5*t7*t8*t10*t11*4.0;
et277 = Lxcm6*Lz6*dQ2*dQ3*m6*t4*t5*t6*t7*t8*t9*t10*-4.0-Lxcm6*Lz6*dQ2*dQ6*m6*t2*t4*t5*t8*t9*t10*t11*2.0-Lxcm6*Lz6*dQ2*dQ6*m6*t3*t4*t5*t7*t9*t10*t11*2.0-Lxcm6*Lz6*dQ3*dQ6*m6*t2*t4*t5*t8*t9*t10*t11*2.0-Lxcm6*Lz6*dQ3*dQ6*m6*t3*t4*t5*t7*t9*t10*t11*2.0-Lxcm6*Lz6*dQ1*dQ2*m6*t2*t3*t4*t6*t7*t8*t35*1.6e+1-Lxcm6*Lz6*dQ1*dQ3*m6*t2*t3*t4*t6*t7*t8*t35*1.6e+1-Lxcm6*Lz6*dQ1*dQ5*m6*t2*t4*t5*t6*t7*t10*t33*1.6e+1-Lxcm6*Lz6*dQ1*dQ5*m6*t3*t4*t5*t6*t8*t10*t32*1.6e+1+Lxcm6*Lz6*dQ1*dQ2*m6*t2*t4*t7*t9*t10*t11*t33*8.0+Lxcm6*Lz6*dQ1*dQ2*m6*t3*t4*t8*t9*t10*t11*t32*8.0+Lxcm6*Lz6*dQ1*dQ3*m6*t2*t4*t7*t9*t10*t11*t33*8.0+Lxcm6*Lz6*dQ1*dQ4*m6*t2*t3*t7*t8*t10*t11*t34*8.0;
et278 = Lxcm6*Lz6*dQ1*dQ3*m6*t3*t4*t8*t9*t10*t11*t32*8.0-Lxcm6*Lz6*dQ1*dQ2*m6*t2*t5*t6*t7*t10*t33*t34*8.0-Lxcm6*Lz6*dQ1*dQ2*m6*t3*t5*t6*t8*t10*t32*t34*8.0-Lxcm6*Lz6*dQ1*dQ3*m6*t2*t5*t6*t7*t10*t33*t34*8.0-Lxcm6*Lz6*dQ1*dQ5*m6*t2*t3*t6*t7*t8*t34*t35*8.0-Lxcm6*Lz6*dQ1*dQ3*m6*t3*t5*t6*t8*t10*t32*t34*8.0-Lxcm6*Lz6*dQ1*dQ4*m6*t4*t5*t6*t9*t10*t32*t33*8.0+Lxcm6*Lzcm6*dQ2*dQ3*m6*t2*t3*t4*t5*t6*t9*t10*4.0+Lxcm6*Lzcm6*dQ1*dQ2*m6*t2*t3*t5*t7*t8*t9*t11*8.0+Lxcm6*Lzcm6*dQ1*dQ3*m6*t2*t3*t5*t7*t8*t9*t11*8.0+Lxcm6*Lzcm6*dQ1*dQ6*m6*t2*t3*t5*t7*t8*t10*t11*4.0-Lxcm6*Lzcm6*dQ2*dQ3*m6*t4*t5*t6*t7*t8*t9*t10*4.0-Lxcm6*Lzcm6*dQ2*dQ6*m6*t2*t4*t5*t8*t9*t10*t11*2.0;
et279 = Lxcm6*Lzcm6*dQ2*dQ6*m6*t3*t4*t5*t7*t9*t10*t11*-2.0-Lxcm6*Lzcm6*dQ3*dQ6*m6*t2*t4*t5*t8*t9*t10*t11*2.0-Lxcm6*Lzcm6*dQ3*dQ6*m6*t3*t4*t5*t7*t9*t10*t11*2.0-Lxcm6*Lzcm6*dQ1*dQ2*m6*t2*t3*t4*t6*t7*t8*t35*1.6e+1-Lxcm6*Lzcm6*dQ1*dQ3*m6*t2*t3*t4*t6*t7*t8*t35*1.6e+1-Lxcm6*Lzcm6*dQ1*dQ5*m6*t2*t4*t5*t6*t7*t10*t33*1.6e+1-Lxcm6*Lzcm6*dQ1*dQ5*m6*t3*t4*t5*t6*t8*t10*t32*1.6e+1+Lxcm6*Lzcm6*dQ1*dQ2*m6*t2*t4*t7*t9*t10*t11*t33*8.0+Lxcm6*Lzcm6*dQ1*dQ2*m6*t3*t4*t8*t9*t10*t11*t32*8.0+Lxcm6*Lzcm6*dQ1*dQ3*m6*t2*t4*t7*t9*t10*t11*t33*8.0+Lxcm6*Lzcm6*dQ1*dQ4*m6*t2*t3*t7*t8*t10*t11*t34*8.0+Lxcm6*Lzcm6*dQ1*dQ3*m6*t3*t4*t8*t9*t10*t11*t32*8.0-Lxcm6*Lzcm6*dQ1*dQ2*m6*t2*t5*t6*t7*t10*t33*t34*8.0;
et280 = Lxcm6*Lzcm6*dQ1*dQ2*m6*t3*t5*t6*t8*t10*t32*t34*-8.0-Lxcm6*Lzcm6*dQ1*dQ3*m6*t2*t5*t6*t7*t10*t33*t34*8.0-Lxcm6*Lzcm6*dQ1*dQ5*m6*t2*t3*t6*t7*t8*t34*t35*8.0-Lxcm6*Lzcm6*dQ1*dQ3*m6*t3*t5*t6*t8*t10*t32*t34*8.0-Lxcm6*Lzcm6*dQ1*dQ4*m6*t4*t5*t6*t9*t10*t32*t33*8.0+Lycm6*Lz6*dQ1*dQ2*m6*t2*t3*t5*t6*t7*t8*t9*8.0+Lycm6*Lz6*dQ1*dQ3*m6*t2*t3*t5*t6*t7*t8*t9*8.0+Lycm6*Lz6*dQ1*dQ6*m6*t2*t3*t5*t6*t7*t8*t10*4.0-Lycm6*Lz6*dQ2*dQ3*m6*t2*t3*t4*t5*t9*t10*t11*4.0-Lycm6*Lz6*dQ2*dQ6*m6*t2*t4*t5*t6*t8*t9*t10*2.0-Lycm6*Lz6*dQ2*dQ6*m6*t3*t4*t5*t6*t7*t9*t10*2.0-Lycm6*Lz6*dQ3*dQ6*m6*t2*t4*t5*t6*t8*t9*t10*2.0-Lycm6*Lz6*dQ3*dQ6*m6*t3*t4*t5*t6*t7*t9*t10*2.0;
et281 = Lycm6*Lz6*dQ2*dQ3*m6*t4*t5*t7*t8*t9*t10*t11*4.0+Lycm6*Lz6*dQ1*dQ2*m6*t2*t3*t4*t7*t8*t11*t35*1.6e+1+Lycm6*Lz6*dQ1*dQ2*m6*t2*t4*t6*t7*t9*t10*t33*8.0+Lycm6*Lz6*dQ1*dQ3*m6*t2*t3*t4*t7*t8*t11*t35*1.6e+1+Lycm6*Lz6*dQ1*dQ2*m6*t3*t4*t6*t8*t9*t10*t32*8.0+Lycm6*Lz6*dQ1*dQ3*m6*t2*t4*t6*t7*t9*t10*t33*8.0+Lycm6*Lz6*dQ1*dQ4*m6*t2*t3*t6*t7*t8*t10*t34*8.0+Lycm6*Lz6*dQ1*dQ3*m6*t3*t4*t6*t8*t9*t10*t32*8.0+Lycm6*Lz6*dQ1*dQ5*m6*t2*t4*t5*t7*t10*t11*t33*1.6e+1+Lycm6*Lz6*dQ1*dQ5*m6*t3*t4*t5*t8*t10*t11*t32*1.6e+1+Lycm6*Lz6*dQ1*dQ2*m6*t2*t5*t7*t10*t11*t33*t34*8.0+Lycm6*Lz6*dQ1*dQ2*m6*t3*t5*t8*t10*t11*t32*t34*8.0+Lycm6*Lz6*dQ1*dQ3*m6*t2*t5*t7*t10*t11*t33*t34*8.0;
et282 = Lycm6*Lz6*dQ1*dQ5*m6*t2*t3*t7*t8*t11*t34*t35*8.0+Lycm6*Lz6*dQ1*dQ3*m6*t3*t5*t8*t10*t11*t32*t34*8.0+Lycm6*Lz6*dQ1*dQ4*m6*t4*t5*t9*t10*t11*t32*t33*8.0+Lycm5*Lzcm5*dQ1*dQ5*m5*t2*t3*t4*t5*t7*t8*t9*4.0+Lycm6*Lzcm6*dQ1*dQ2*m6*t2*t3*t5*t6*t7*t8*t9*8.0+Lycm6*Lzcm6*dQ1*dQ3*m6*t2*t3*t5*t6*t7*t8*t9*8.0+Lycm6*Lzcm6*dQ1*dQ6*m6*t2*t3*t5*t6*t7*t8*t10*4.0-Lycm6*Lzcm6*dQ2*dQ3*m6*t2*t3*t4*t5*t9*t10*t11*4.0-Lycm6*Lzcm6*dQ2*dQ6*m6*t2*t4*t5*t6*t8*t9*t10*2.0-Lycm6*Lzcm6*dQ2*dQ6*m6*t3*t4*t5*t6*t7*t9*t10*2.0-Lycm6*Lzcm6*dQ3*dQ6*m6*t2*t4*t5*t6*t8*t9*t10*2.0-Lycm6*Lzcm6*dQ3*dQ6*m6*t3*t4*t5*t6*t7*t9*t10*2.0+Lycm6*Lzcm6*dQ2*dQ3*m6*t4*t5*t7*t8*t9*t10*t11*4.0;
et283 = Lycm6*Lzcm6*dQ1*dQ2*m6*t2*t3*t4*t7*t8*t11*t35*1.6e+1+Lycm6*Lzcm6*dQ1*dQ2*m6*t2*t4*t6*t7*t9*t10*t33*8.0+Lycm6*Lzcm6*dQ1*dQ3*m6*t2*t3*t4*t7*t8*t11*t35*1.6e+1+Lycm6*Lzcm6*dQ1*dQ2*m6*t3*t4*t6*t8*t9*t10*t32*8.0+Lycm6*Lzcm6*dQ1*dQ3*m6*t2*t4*t6*t7*t9*t10*t33*8.0+Lycm6*Lzcm6*dQ1*dQ4*m6*t2*t3*t6*t7*t8*t10*t34*8.0+Lycm6*Lzcm6*dQ1*dQ3*m6*t3*t4*t6*t8*t9*t10*t32*8.0+Lycm6*Lzcm6*dQ1*dQ5*m6*t2*t4*t5*t7*t10*t11*t33*1.6e+1+Lycm6*Lzcm6*dQ1*dQ5*m6*t3*t4*t5*t8*t10*t11*t32*1.6e+1+Lycm6*Lzcm6*dQ1*dQ2*m6*t2*t5*t7*t10*t11*t33*t34*8.0+Lycm6*Lzcm6*dQ1*dQ2*m6*t3*t5*t8*t10*t11*t32*t34*8.0+Lycm6*Lzcm6*dQ1*dQ3*m6*t2*t5*t7*t10*t11*t33*t34*8.0+Lycm6*Lzcm6*dQ1*dQ5*m6*t2*t3*t7*t8*t11*t34*t35*8.0;
et284 = Lycm6*Lzcm6*dQ1*dQ3*m6*t3*t5*t8*t10*t11*t32*t34*8.0+Lycm6*Lzcm6*dQ1*dQ4*m6*t4*t5*t9*t10*t11*t32*t33*8.0-Lz6*Lzcm6*dQ1*dQ2*m6*t2*t3*t4*t5*t7*t8*t10*1.6e+1-Lz6*Lzcm6*dQ1*dQ3*m6*t2*t3*t4*t5*t7*t8*t10*1.6e+1-Lz6*Lzcm6*dQ1*dQ4*m6*t2*t3*t4*t7*t8*t9*t35*8.0-Lz6*Lzcm6*dQ1*dQ5*m6*t2*t3*t5*t7*t8*t10*t34*8.0-dQ1*dQ2*m6*t2*t3*t6*t7*t8*t9*t10*t11*t18*8.0-dQ1*dQ3*m6*t2*t3*t6*t7*t8*t9*t10*t11*t18*8.0+dQ1*dQ2*m6*t2*t3*t6*t7*t8*t9*t10*t11*t21*8.0+dQ1*dQ3*m6*t2*t3*t6*t7*t8*t9*t10*t11*t21*8.0+dQ1*dQ2*m6*t2*t3*t4*t5*t7*t8*t10*t18*t36*8.0+dQ1*dQ3*m6*t2*t3*t4*t5*t7*t8*t10*t18*t36*8.0;
et285 = dQ1*dQ2*m6*t2*t4*t5*t6*t7*t9*t11*t18*t33*8.0-dQ1*dQ2*m6*t2*t3*t4*t5*t7*t8*t10*t21*t36*8.0+dQ1*dQ2*m6*t3*t4*t5*t6*t8*t9*t11*t18*t32*8.0+dQ1*dQ3*m6*t2*t4*t5*t6*t7*t9*t11*t18*t33*8.0+dQ1*dQ4*m6*t2*t3*t5*t6*t7*t8*t11*t18*t34*8.0+dQ1*dQ6*m6*t2*t3*t4*t5*t7*t8*t9*t18*t36*8.0-dQ1*dQ3*m6*t2*t3*t4*t5*t7*t8*t10*t21*t36*8.0+dQ1*dQ3*m6*t3*t4*t5*t6*t8*t9*t11*t18*t32*8.0-dQ1*dQ2*m6*t2*t4*t5*t6*t7*t9*t11*t21*t33*8.0-dQ1*dQ2*m6*t3*t4*t5*t6*t8*t9*t11*t21*t32*8.0-dQ1*dQ3*m6*t2*t4*t5*t6*t7*t9*t11*t21*t33*8.0-dQ1*dQ4*m6*t2*t3*t5*t6*t7*t8*t11*t21*t34*8.0;
et286 = dQ1*dQ6*m6*t2*t3*t4*t5*t7*t8*t9*t21*t36*-8.0-dQ1*dQ3*m6*t3*t4*t5*t6*t8*t9*t11*t21*t32*8.0+dQ1*dQ6*m6*t2*t4*t5*t6*t7*t10*t11*t18*t33*8.0+dQ1*dQ6*m6*t3*t4*t5*t6*t8*t10*t11*t18*t32*8.0-dQ1*dQ6*m6*t2*t4*t5*t6*t7*t10*t11*t21*t33*8.0-dQ1*dQ6*m6*t3*t4*t5*t6*t8*t10*t11*t21*t32*8.0+dQ1*dQ4*m6*t2*t3*t4*t7*t8*t9*t18*t35*t36*4.0+dQ1*dQ5*m6*t2*t3*t5*t7*t8*t10*t18*t34*t36*4.0-dQ1*dQ4*m6*t2*t3*t4*t7*t8*t9*t21*t35*t36*4.0+dQ1*dQ6*m6*t2*t3*t6*t7*t8*t11*t18*t34*t35*4.0-dQ1*dQ5*m6*t2*t3*t5*t7*t8*t10*t21*t34*t36*4.0-dQ1*dQ6*m6*t2*t3*t6*t7*t8*t11*t21*t34*t35*4.0-dQ1*dQ5*m6*t2*t3*t4*t6*t7*t8*t9*t10*t11*t18*4.0;
et287 = dQ1*dQ5*m6*t2*t3*t4*t6*t7*t8*t9*t10*t11*t21*4.0+Lx4*Lxcm6*dQ1*dQ4*m6*t2*t3*t4*t5*t6*t7*t8*t9*8.0-Lx4*Lycm6*dQ1*dQ4*m6*t2*t3*t4*t5*t7*t8*t9*t11*8.0-Lxcm6*Lycm6*dQ1*dQ4*m6*t2*t3*t4*t6*t7*t8*t9*t11*8.0-Lxcm6*Lycm6*dQ1*dQ5*m6*t2*t3*t5*t6*t7*t8*t10*t11*8.0-Lxcm6*Lycm6*dQ1*dQ5*m6*t2*t3*t4*t7*t8*t9*t10*t36*8.0-Lxcm6*Lycm6*dQ1*dQ4*m6*t2*t5*t6*t7*t9*t10*t11*t33*8.0-Lxcm6*Lycm6*dQ1*dQ4*m6*t3*t5*t6*t8*t9*t10*t11*t32*8.0+Lxcm6*Lz6*dQ1*dQ5*m6*t2*t3*t4*t5*t7*t8*t9*t11*4.0+Lxcm6*Lz6*dQ1*dQ6*m6*t2*t3*t4*t6*t7*t8*t9*t10*4.0+Lxcm6*Lz6*dQ1*dQ6*m6*t2*t3*t5*t7*t8*t10*t11*t34*4.0+Lxcm5*Lzcm5*dQ1*dQ4*m5*t2*t3*t4*t5*t7*t8*t9*t10*8.0;
et288 = Lxcm6*Lzcm6*dQ1*dQ5*m6*t2*t3*t4*t5*t7*t8*t9*t11*4.0+Lxcm6*Lzcm6*dQ1*dQ6*m6*t2*t3*t4*t6*t7*t8*t9*t10*4.0+Lxcm6*Lzcm6*dQ1*dQ6*m6*t2*t3*t5*t7*t8*t10*t11*t34*4.0+Lycm6*Lz6*dQ1*dQ5*m6*t2*t3*t4*t5*t6*t7*t8*t9*4.0-Lycm6*Lz6*dQ1*dQ6*m6*t2*t3*t4*t7*t8*t9*t10*t11*4.0+Lycm6*Lz6*dQ1*dQ6*m6*t2*t3*t5*t6*t7*t8*t10*t34*4.0+Lycm6*Lzcm6*dQ1*dQ5*m6*t2*t3*t4*t5*t6*t7*t8*t9*4.0-Lycm6*Lzcm6*dQ1*dQ6*m6*t2*t3*t4*t7*t8*t9*t10*t11*4.0+Lycm6*Lzcm6*dQ1*dQ6*m6*t2*t3*t5*t6*t7*t8*t10*t34*4.0-Lxcm6*Lycm6*dQ1*dQ2*m6*t2*t3*t4*t5*t6*t7*t8*t10*t11*1.6e+1-Lxcm6*Lycm6*dQ1*dQ3*m6*t2*t3*t4*t5*t6*t7*t8*t10*t11*1.6e+1-Lxcm6*Lycm6*dQ1*dQ6*m6*t2*t3*t4*t5*t6*t7*t8*t9*t11*1.6e+1;
et289 = Lxcm6*Lycm6*dQ1*dQ4*m6*t2*t3*t4*t6*t7*t8*t9*t11*t35*-8.0-Lxcm6*Lycm6*dQ1*dQ5*m6*t2*t3*t5*t6*t7*t8*t10*t11*t34*8.0+Lxcm6*Lz6*dQ1*dQ4*m6*t2*t3*t4*t5*t6*t7*t8*t9*t10*8.0+Lxcm6*Lzcm6*dQ1*dQ4*m6*t2*t3*t4*t5*t6*t7*t8*t9*t10*8.0-Lycm6*Lz6*dQ1*dQ4*m6*t2*t3*t4*t5*t7*t8*t9*t10*t11*8.0-Lycm6*Lzcm6*dQ1*dQ4*m6*t2*t3*t4*t5*t7*t8*t9*t10*t11*8.0;
et290 = et1+et2+et3+et4+et5+et6+et7+et8+et9+et10+et11+et12+et13+et14+et15+et16+et17+et18+et19+et20+et21+et22+et23+et24+et25+et26+et27+et28+et29+et30+et31+et32+et33+et34+et35+et36+et37+et38+et39+et40+et41+et42+et43+et44+et45+et46+et47+et48+et49+et50+et51+et52+et53+et54+et55+et56+et57+et58+et59+et60+et61+et62+et63+et64+et65+et66+et67+et68+et69+et70+et71+et72+et73+et74+et75+et76+et77+et78+et79+et80+et81+et82+et83+et84+et85+et86+et87+et88+et89+et90+et91+et92+et93+et94+et95+et96+et97+et98+et99+et100+et101+et102+et103+et104+et105+et106+et107+et108+et109+et110+et111+et112+et113+et114+et115+et116+et117+et118+et119+et120+et121+et122+et123+et124+et125+et126+et127+et128+et129+et130+et131+et132+et133+et134+et135+et136+et137+et138+et139+et140+et141+et142+et143+et144+et145+et146+et147+et148+et149+et150+et151+et152+et153+et154+et155+et156+et157+et158+et159+et160+et161+et162+et163+et164+et165+et166+et167+et168+et169+et170+et171+et172+et173+et174+et175+et176+et177+et178+et179+et180+et181+et182+et183+et184+et185+et186+et187+et188+et189+et190+et191+et192+et193+et194+et195+et196+et197+et198+et199+et200;
et291 = et201+et202+et203+et204+et205+et206+et207+et208+et209+et210+et211+et212+et213+et214+et215+et216+et217+et218+et219+et220+et221+et222+et223+et224+et225+et226+et227+et228+et229+et230+et231+et232+et233+et234+et235+et236+et237+et238+et239+et240+et241+et242+et243+et244+et245+et246+et247+et248+et249+et250+et251+et252+et253+et254+et255+et256+et257+et258+et259+et260+et261+et262+et263+et264+et265+et266+et267+et268+et269+et270+et271+et272+et273+et274+et275+et276+et277+et278+et279+et280+et281+et282+et283+et284+et285+et286+et287+et288+et289;
et292 = t42+t45+t48+t49+t50+t51+t52+t53+t54+t55+t56+t57+t58+t59+t60+t61+t72+t73+t74+t75+t76+t77+t78+t79+t80+t81+t82+t83+t86+t92+t93+t95+t96+t97+t98+t99+t100+t101+t102+t103+t108+t109+t110+t111+t114+t115+t116+t117+t118+t127+t128+t131+t132+t137+t138+t139+t140+t141+t142+t143+t144+t145+t146+t147+t152+t153+t154+t157+t158+t160+t161+t163+t164+t165+t166+t167+t168+t169+t170+t171+t172+t173+t174+t175+t176+t177+t178+t179+t180+t181+t182+t183+t184+t185+t186+t187+t188+t189+t190+t191+t192+t199+t201+t208+t211+t212+t227+t228+t229+t230+t231+t232+t233+t234+t235+t236+t252+t253+t254+t255+t256+t257+t262+t263+t264+t265+t266+t277+t278+t279+t280+t281+t282+t289+t290+t291+t292+t293+t294+t295+t296+t297+t298+t299+t300+t301+t302+t303+t304+t305+t306+t307+t308+t309+t310+t311+t312+t313+t314+t316+t318+t320+t321+t322+t323+t324+t325+t326+t327+t328+t329+t330+t331+t332+t333+t334+t335+t336+t337+t338+t339+t340+t341+t342+t343+t344+t345+t346+t347+t348+t349+t350+t351+t352+t353+t354+t355+t356+t357+t358;
et293 = t363+t364+t365+t366+t369+t370+t371+t372+t380+t382+t383+t384+t385+t386+t387+t388+t389+t401+t402+t403+t404+t409+t410+t411+t412+t413+t414+t415+t416+t417+t418+t419+t420+t421+t422+t423+t424+t425+t426+t427+t428+t429+t430+t431+t436+t437+t438+t439+t440+t441+t442+t443+t446+t447+t450+t451+t454+t459+t460+t461+t463+t464+t465+t471+t472+t473+t474+t476+t477+t478+t479+t480+t481+t492+t493+t494+t495+t496+t497+t498+t499+t500+t501+t503+t506+t509+t510+t511+t512+t513+t516+t518+t519+t521+t522+t524+t525+t527+t528+t542+t543+t544+t545+t546+t547+t548+t549+t551+t552+t556+t557+t558+t559+t560+t561+t562+t563+t564+t565+t566+t567+t568+t569+t570+t571+t572+t573+t574+t575+t576+t577+t578+t579+t580+t581+t582+t583+t584+t585+t586+t587+t588+t589+t590+t591+t592+t593+t595+t596+t597+t598+t599+t600+t607+t608+t609+t610+t611+t612+t613+t614+t615+t616+t617+t618+t619+t620+t621+t622+t623+t624+t625+t626+t627+t628+t629+t630+t631+t632+t633+t634+t635+t636+t637+t638+t639+t640+t641+t642+t643+t644+t645+t646+t647+t648+t649+t650+t651+t654+t655;
et294 = t656+t657+t658+t659+t660+t668+t674+t675+t676+t677+t686+t687+t691+t692+t693+t694+t695+t696+t697+t701+t702+t703+t704+t705+t706+t707+t708+t709+t710+t711+t712+t713+t714+t715+t716+t724+t736+t737+t742+t743+t744+t745+t746+t747+t756+t757+t758+t761+t762+t763+t765+t767+t768+t770+t772+t773+t774+t776+t777+t778+t779+t780+t781+t782+t783+t787+t788+t789+t790+t791+t792+t793+t794+t795+t806+t807+t808+t809+t816+t819+t820+t821+t822+t823+t824+t825+t826+t827+t830+t833+t834+t836+t837+t843+t844+t845+t846+t847+t848+t849+t850+t851+t852+t853+t854+t855+t856+t857+t858+t859+t860+t861+t862+t863+t864+t865+t866+t867+t868+t869+t870+t871+t872+t873+t874+t875+t876+t877+t878+t879+t880+t881+t882+t883+t884+t885+t886+t887+t888+t889+t890+t891+t892+t893+t894+t895+t896+t897+t898+t899+t900+t901+t902+t903+t904+t905+t906+t907+t909+t910+t911+t912+t913+t914+t915+t916+t917+t918+t919+t920+t921+t922+t923+t924+t925+t926+t927+t928+t929+t930+t931+t932+t933+t934+t935+t936+t937+t938+t939+t940+t941+t942+t943+t944+t955+t957+t958+t960+t961+t967;
et295 = t968+t970+t973+t976+t979+t982+t983+t984+t985+t986+t987+t988+t989+t990+t991+t992+t993+t994+t995+t996+t997+t998+t999+t1000+t1001+t1002+t1003+t1004+t1005+t1006+t1007+t1008+t1009+t1010+t1015+t1016+t1017+t1018+t1019+t1020+t1023+t1024+t1031+t1032+t1033+t1034+t1039+t1042+t1043+t1044+t1045+t1046+t1049+t1050+t1058+t1059+t1060+t1061+t1062+t1063+t1066+t1067+t1068+t1069+t1070+t1071+t1074+t1077+t1079+t1082+t1083+t1084+t1085+t1086+t1087+t1088+t1090+t1091+t1092+t1093+t1094+t1095+t1096+t1097+t1098+t1099+t1100+t1101+t1102+t1103+t1104+t1105+t1106+t1107+t1108+t1109+t1110+t1111+t1112+t1113+t1114+t1115+t1125+t1126+t1127+t1128+t1129+t1130+t1131+t1132+t1133+t1134+t1135+t1136+t1137+t1140+t1143+t1144+t1147+t1150+t1151+t1152+t1153+t1154+t1155+t1156+t1174+t1175+t1177+t1178+t1182+t1183+t1185+t1186+t1187+t1188+t1189+t1190+t1197+t1200+t1201+t1202+t1203+t1204+t1205+t1206+t1207+t1208+t1209+t1210+t1211+t1212+t1213+t1214+t1215+t1216+t1218+t1219+t1220+t1221+t1222+t1223+t1224+t1225+t1226+t1227+t1228+t1229+t1230+t1231+t1232+t1233+t1234+t1235+t1245+t1246+t1247+t1248+t1249+t1250+t1251+t1252+t1253+t1254+t1258+t1260+t1263+t1264+t1265+t1266+t1267+t1268+t1269+t1270+t1271+t1272+t1273+t1274+t1275+t1276;
et296 = t1277+t1278+t1279+t1280+t1281+t1282+t1283+t1284+t1285+t1286+t1287+t1288+t1289+t1293+t1294+t1295+t1296+t1297+t1298+t1299+t1300+t1301+t1302+t1303+t1304+t1305+t1306+t1307+t1308+t1309+t1310+t1311+t1312+t1313+t1314+t1315+t1316+t1317+t1318+t1319+t1321+t1322+t1323+t1324+t1331+t1332+t1333+t1334+t1335+t1336+t1337+t1341+t1342+t1343+t1344+t1345+t1346+t1347+t1348+t1349+t1350+t1351+t1352+t1355+t1356+t1362+t1363+t1364+t1365+t1366+t1367+t1368+t1369+t1370+t1371+t1372+t1373+t1374+t1375+t1376+t1377+t1378+t1379+t1380+t1381+t1382+t1383+t1384+t1396+t1401+t1402+t1403+t1404+t1405+t1406+t1407+t1408+t1409+t1410+t1411+t1412+t1416+t1417+t1418+t1419+t1420+t1434+t1435+t1436+t1437+t1438+t1439+t1440+t1441+t1449+t1450+t1451+t1455+t1456+t1457+t1460+t1461+t1462+t1463+t1465+t1466+t1467+t1468+t1469+t1470+t1471+t1472+t1473+t1474+t1475+t1476+t1477+t1478+t1479+t1480+t1481+t1482+t1484+t1485+t1486+t1487+t1488+t1489+t1490+t1491+t1492+t1493+t1494+t1495+t1496+t1498+t1499+t1500+t1501+t1502+t1503+t1504+t1505+t1506+t1507+t1508+t1509+t1510+t1511+t1512+t1513+t1514+t1515+t1516+t1517+t1518+t1519+t1520+t1521+t1522+t1530+t1531+t1532+t1533+t1534+t1535+t1536+t1537+t1538+t1539+t1540+t1541+t1542+t1543+t1545+t1546+t1547+t1548+t1549+t1550;
et297 = t1557+t1558+t1561+t1562+t1563+t1564+t1565+t1566+t1573+t1574+t1575+t1578+t1579+t1580+t1586+t1587+t1594+t1595+t1596+t1597+t1598+t1599+t1600+t1601+t1602+t1603+t1604+t1605+t1606+t1607+t1608+t1609+t1610+t1611+t1612+t1613+t1614+t1615+t1618+t1619+t1620+t1621+t1622+t1623+t1624+t1625+t1626+t1627+t1628+t1629+t1645+t1646+t1647+t1648+t1649+t1650+t1651+t1652+t1653+t1654+t1655+t1656+t1657+t1658+t1662+t1663+t1664+t1665+t1667+t1668+t1669+t1670+t1671+t1676+t1677+t1678+t1683+t1685+t1686+t1687+t1688+t1689+t1690+t1691+t1692+t1693+t1694+t1695+t1696+t1697+t1698+t1699+t1700+t1701+t1706+t1707+t1708+t1709+t1710+t1711+t1712+t1713+t1714+t1715+t1716+t1717+t1718+t1719+t1720+t1721+t1722+t1727+t1728+t1729+t1730+t1731+t1732+t1735+t1736+t1737+t1738+t1739+t1740-Lx2*Lx3*dQ2*dQ3*m3*t8*2.0-Lx2*Lx3*dQ2*dQ3*m4*t8*2.0-Lx2*Lx3*dQ2*dQ3*m5*t8*2.0-Lx2*Lx3*dQ2*dQ3*m6*t8*2.0-Lx2*Lxcm3*dQ2*dQ3*m3*t8*2.0+Lx2*Lzcm3*dQ2*dQ3*m3*t3*2.0+Lx2*Lzcm4*dQ2*dQ3*m4*t3*2.0+Lx2*Lx4*dQ1*dQ4*m4*t4*t7*2.0;
et298 = Lx2*Lx4*dQ1*dQ4*m5*t4*t7*2.0-Lx2*Lx4*dQ2*dQ3*m4*t4*t8*2.0+Lx2*Lx4*dQ1*dQ4*m6*t4*t7*2.0-Lx2*Lx4*dQ2*dQ3*m5*t4*t8*2.0-Lx2*Lx4*dQ2*dQ4*m4*t3*t9*2.0-Lx2*Lx4*dQ2*dQ3*m6*t4*t8*2.0-Lx2*Lx4*dQ2*dQ4*m5*t3*t9*2.0-Lx2*Lx4*dQ3*dQ4*m4*t3*t9*2.0-Lx2*Lx4*dQ2*dQ4*m6*t3*t9*2.0-Lx2*Lx4*dQ3*dQ4*m5*t3*t9*2.0-Lx2*Lx4*dQ3*dQ4*m6*t3*t9*2.0+Lx2*Lxcm4*dQ1*dQ4*m4*t4*t7*2.0-Lx2*Lxcm4*dQ2*dQ3*m4*t4*t8*2.0-Lx2*Lxcm4*dQ2*dQ4*m4*t3*t9*2.0-Lx2*Lxcm4*dQ3*dQ4*m4*t3*t9*2.0-Lx2*Lxcm5*dQ2*dQ3*m5*t3*t10*2.0-Lx2*Lxcm5*dQ2*dQ5*m5*t5*t8*2.0-Lx2*Lxcm5*dQ3*dQ5*m5*t5*t8*2.0-Lx2*Lycm4*dQ2*dQ4*m4*t3*t4*2.0-Lx2*Lycm4*dQ3*dQ4*m4*t3*t4*2.0;
et299 = Lx2*Lycm5*dQ2*dQ4*m5*t3*t4*-2.0-Lx2*Lycm5*dQ3*dQ4*m5*t3*t4*2.0-Lx2*Lycm4*dQ1*dQ4*m4*t7*t9*2.0+Lx2*Lycm4*dQ2*dQ3*m4*t8*t9*2.0-Lx2*Lycm5*dQ1*dQ4*m5*t7*t9*2.0+Lx2*Lycm5*dQ2*dQ3*m5*t8*t9*2.0+Lx2*Lz6*dQ2*dQ3*m6*t3*t5*2.0-Lx2*Lz6*dQ2*dQ5*m6*t8*t10*2.0-Lx2*Lz6*dQ3*dQ5*m6*t8*t10*2.0+Lx2*Lzcm5*dQ2*dQ3*m5*t3*t5*2.0+Lx2*Lzcm6*dQ2*dQ3*m6*t3*t5*2.0-Lx2*Lzcm5*dQ2*dQ5*m5*t8*t10*2.0-Lx2*Lzcm5*dQ3*dQ5*m5*t8*t10*2.0-Lx2*Lzcm6*dQ2*dQ5*m6*t8*t10*2.0-Lx2*Lzcm6*dQ3*dQ5*m6*t8*t10*2.0+Lx2*Lxcm5*dQ1*dQ4*m5*t4*t5*t7*2.0-Lx2*Lxcm5*dQ2*dQ3*m5*t4*t5*t8*2.0-Lx2*Lxcm5*dQ2*dQ4*m5*t3*t5*t9*2.0-Lx2*Lxcm5*dQ2*dQ5*m5*t3*t4*t10*2.0-Lx2*Lxcm5*dQ3*dQ4*m5*t3*t5*t9*2.0;
et300 = Lx2*Lxcm5*dQ3*dQ5*m5*t3*t4*t10*-2.0+Lx2*Lxcm6*dQ1*dQ6*m6*t4*t6*t7*2.0-Lx2*Lxcm6*dQ2*dQ3*m6*t3*t6*t10*2.0-Lx2*Lxcm6*dQ2*dQ4*m6*t3*t4*t11*2.0-Lx2*Lxcm6*dQ3*dQ4*m6*t3*t4*t11*2.0-Lx2*Lxcm6*dQ2*dQ5*m6*t5*t6*t8*2.0-Lx2*Lxcm6*dQ2*dQ6*m6*t3*t6*t9*2.0-Lx2*Lxcm6*dQ3*dQ5*m6*t5*t6*t8*2.0-Lx2*Lxcm6*dQ3*dQ6*m6*t3*t6*t9*2.0-Lx2*Lxcm6*dQ4*dQ6*m6*t4*t6*t8*2.0-Lx2*Lxcm5*dQ1*dQ5*m5*t7*t9*t10*2.0-Lx2*Lxcm6*dQ5*dQ6*m6*t3*t5*t11*2.0-Lx2*Lxcm6*dQ1*dQ4*m6*t7*t9*t11*2.0+Lx2*Lxcm6*dQ2*dQ3*m6*t8*t9*t11*2.0+Lx2*Lxcm5*dQ4*dQ5*m5*t8*t9*t10*2.0+Lx2*Lxcm6*dQ2*dQ6*m6*t8*t10*t11*2.0+Lx2*Lxcm6*dQ3*dQ6*m6*t8*t10*t11*2.0-Lx2*Lycm6*dQ2*dQ4*m6*t3*t4*t6*2.0;
et301 = Lx2*Lycm6*dQ3*dQ4*m6*t3*t4*t6*-2.0-Lx2*Lycm6*dQ5*dQ6*m6*t3*t5*t6*2.0-Lx2*Lycm6*dQ1*dQ4*m6*t6*t7*t9*2.0+Lx2*Lycm6*dQ2*dQ3*m6*t6*t8*t9*2.0-Lx2*Lycm6*dQ1*dQ6*m6*t4*t7*t11*2.0+Lx2*Lycm6*dQ2*dQ3*m6*t3*t10*t11*2.0+Lx2*Lycm6*dQ2*dQ5*m6*t5*t8*t11*2.0+Lx2*Lycm6*dQ2*dQ6*m6*t3*t9*t11*2.0+Lx2*Lycm6*dQ2*dQ6*m6*t6*t8*t10*2.0+Lx2*Lycm6*dQ3*dQ5*m6*t5*t8*t11*2.0+Lx2*Lycm6*dQ3*dQ6*m6*t3*t9*t11*2.0+Lx2*Lycm6*dQ3*dQ6*m6*t6*t8*t10*2.0+Lx2*Lycm6*dQ4*dQ6*m6*t4*t8*t11*2.0+Lx2*Lz6*dQ2*dQ5*m6*t3*t4*t5*2.0+Lx2*Lz6*dQ3*dQ5*m6*t3*t4*t5*2.0+Lx2*Lz6*dQ1*dQ4*m6*t4*t7*t10*2.0+Lx2*Lz6*dQ1*dQ5*m6*t5*t7*t9*2.0-Lx2*Lz6*dQ2*dQ3*m6*t4*t8*t10*2.0-Lx2*Lz6*dQ2*dQ4*m6*t3*t9*t10*2.0;
et302 = Lx2*Lz6*dQ3*dQ4*m6*t3*t9*t10*-2.0-Lx2*Lz6*dQ4*dQ5*m6*t5*t8*t9*2.0+Lx2*Lzcm5*dQ2*dQ5*m5*t3*t4*t5*2.0+Lx2*Lzcm5*dQ3*dQ5*m5*t3*t4*t5*2.0+Lx2*Lzcm6*dQ2*dQ5*m6*t3*t4*t5*2.0+Lx2*Lzcm6*dQ3*dQ5*m6*t3*t4*t5*2.0+Lx2*Lzcm5*dQ1*dQ4*m5*t4*t7*t10*2.0+Lx2*Lzcm5*dQ1*dQ5*m5*t5*t7*t9*2.0-Lx2*Lzcm5*dQ2*dQ3*m5*t4*t8*t10*2.0-Lx2*Lzcm5*dQ2*dQ4*m5*t3*t9*t10*2.0+Lx2*Lzcm6*dQ1*dQ4*m6*t4*t7*t10*2.0-Lx2*Lzcm5*dQ3*dQ4*m5*t3*t9*t10*2.0+Lx2*Lzcm6*dQ1*dQ5*m6*t5*t7*t9*2.0-Lx2*Lzcm6*dQ2*dQ3*m6*t4*t8*t10*2.0-Lx2*Lzcm6*dQ2*dQ4*m6*t3*t9*t10*2.0-Lx2*Lzcm5*dQ4*dQ5*m5*t5*t8*t9*2.0-Lx2*Lzcm6*dQ3*dQ4*m6*t3*t9*t10*2.0-Lx2*Lzcm6*dQ4*dQ5*m6*t5*t8*t9*2.0;
et303 = Lx2*Lxcm6*dQ1*dQ4*m6*t4*t5*t6*t7*2.0-Lx2*Lxcm6*dQ2*dQ3*m6*t4*t5*t6*t8*2.0-Lx2*Lxcm6*dQ2*dQ4*m6*t3*t5*t6*t9*2.0-Lx2*Lxcm6*dQ2*dQ5*m6*t3*t4*t6*t10*2.0-Lx2*Lxcm6*dQ3*dQ4*m6*t3*t5*t6*t9*2.0-Lx2*Lxcm6*dQ2*dQ6*m6*t3*t4*t5*t11*2.0-Lx2*Lxcm6*dQ3*dQ5*m6*t3*t4*t6*t10*2.0-Lx2*Lxcm6*dQ3*dQ6*m6*t3*t4*t5*t11*2.0-Lx2*Lxcm6*dQ1*dQ5*m6*t6*t7*t9*t10*2.0-Lx2*Lxcm6*dQ1*dQ6*m6*t5*t7*t9*t11*2.0+Lx2*Lxcm6*dQ4*dQ5*m6*t6*t8*t9*t10*2.0+Lx2*Lxcm6*dQ4*dQ6*m6*t5*t8*t9*t11*2.0+Lx2*Lxcm6*dQ5*dQ6*m6*t4*t8*t10*t11*2.0-Lx2*Lycm6*dQ2*dQ6*m6*t3*t4*t5*t6*2.0-Lx2*Lycm6*dQ3*dQ6*m6*t3*t4*t5*t6*2.0-Lx2*Lycm6*dQ1*dQ4*m6*t4*t5*t7*t11*2.0+Lx2*Lycm6*dQ2*dQ3*m6*t4*t5*t8*t11*2.0;
